simulink model "D_20210914_Modell_Inbetriebnahme_BreakOutBox_Jetson"  (R2021a)
(part 4 of 7)

  CAN Unpack52 : canmsglib/CAN Unpack  CANdbFile=eWolf_SensorCAN.dbc  MsgList=Radar_RawTarget_Data_051  MsgName=Radar_RawTarget_Data_051  MsgIDType=Standard (11-bit identifier)  MsgIdentifier=1075  MsgLength=8  SignalInfo={ 'AZ_Winkel', '22', '10', 'LE', 'unsigned', 'Multiplexed', '0', '0.16', '-81.76', '-81.76', '81.92'; 'EL_Angle', '37', '10', 'LE', 'unsigned', 'Multiplexed', '1', '0.04', '-20.44', '-20.44', '20.48'; 'Internal_used', '14', '8', 'LE', 'unsigned', 'Multiplexed', '0', '1', '0', '-Inf', 'Inf'; 'Internal_used2', '32', '7', 'LE', 'unsigned', 'Multiplexed', '0', '1', '0', '-Inf', 'Inf'; 'Internal_used3', '51', '7', 'LE', 'unsigned', 'Multiplexed', '0', '1', '0', '-Inf', 'Inf'; 'Internal_used4', '58', '6', 'LE', 'unsigned', 'Multiplexed', '0', '1', '0', '-Inf', 'Inf'; 'Internal_used5', '9', '8', 'LE', 'unsigned', 'Multiplexed', '1', '1', '0', '-Inf', 'Inf'; 'Internal_used6', '17', '8', 'LE', 'unsigned', 'Multiplexed', '1', '1', '0', '-Inf', 'Inf'; 'Internal_used7', '25', '7', 'LE', 'unsigned', 'Multiplexed', '1', '1', '0', '-Inf', 'Inf'; 'Mode_Signal', '0', '1', 'LE', 'unsigned', 'Multiplexor', '0', '1', '0', '0', '1'; 'RCS', '1', '7', 'LE', 'unsigned', 'Multiplexed', '1', '0.2', '-15', '-15', '36'; 'Range1', '1', '13', 'LE', 'unsigned', 'Multiplexed', '0', '0.04', '0', '0', '327.64'; 'Reserve_3', '32', '5', 'LE', 'unsigned', 'Multiplexed', '1', '1', '0', '-Inf', 'Inf'; 'Reserve_4', '47', '16', 'LE', 'unsigned', 'Multiplexed', '1', '1', '0', '-Inf', 'Inf'; 'Speed_Radial', '39', '12', 'LE', 'unsigned', 'Multiplexed', '0', '0.04', '-119.68', '-44.12', '119.68' }  IDPort=on  TimestampPort=on  ErrorPort=off  RemotePort=off  LengthPort=off  StatusPort=off  ApplyMinMax=off
      settings: SourceProductBaseCode=ME,XP,VN  DataFormat=CANdb specified signals
  CAN Unpack53 : canmsglib/CAN Unpack  CANdbFile=eWolf_SensorCAN.dbc  MsgList=Radar_RawTarget_Data_052  MsgName=Radar_RawTarget_Data_052  MsgIDType=Standard (11-bit identifier)  MsgIdentifier=1076  MsgLength=8  SignalInfo={ 'AZ_Winkel', '22', '10', 'LE', 'unsigned', 'Multiplexed', '0', '0.16', '-81.76', '-81.76', '81.92'; 'EL_Angle', '37', '10', 'LE', 'unsigned', 'Multiplexed', '1', '0.04', '-20.44', '-20.44', '20.48'; 'Internal_used', '14', '8', 'LE', 'unsigned', 'Multiplexed', '0', '1', '0', '-Inf', 'Inf'; 'Internal_used2', '32', '7', 'LE', 'unsigned', 'Multiplexed', '0', '1', '0', '-Inf', 'Inf'; 'Internal_used3', '51', '7', 'LE', 'unsigned', 'Multiplexed', '0', '1', '0', '-Inf', 'Inf'; 'Internal_used4', '58', '6', 'LE', 'unsigned', 'Multiplexed', '0', '1', '0', '-Inf', 'Inf'; 'Internal_used5', '9', '8', 'LE', 'unsigned', 'Multiplexed', '1', '1', '0', '-Inf', 'Inf'; 'Internal_used6', '17', '8', 'LE', 'unsigned', 'Multiplexed', '1', '1', '0', '-Inf', 'Inf'; 'Internal_used7', '25', '7', 'LE', 'unsigned', 'Multiplexed', '1', '1', '0', '-Inf', 'Inf'; 'Mode_Signal', '0', '1', 'LE', 'unsigned', 'Multiplexor', '0', '1', '0', '0', '1'; 'RCS', '1', '7', 'LE', 'unsigned', 'Multiplexed', '1', '0.2', '-15', '-15', '36'; 'Range1', '1', '13', 'LE', 'unsigned', 'Multiplexed', '0', '0.04', '0', '0', '327.64'; 'Reserve_3', '32', '5', 'LE', 'unsigned', 'Multiplexed', '1', '1', '0', '-Inf', 'Inf'; 'Reserve_4', '47', '16', 'LE', 'unsigned', 'Multiplexed', '1', '1', '0', '-Inf', 'Inf'; 'Speed_Radial', '39', '12', 'LE', 'unsigned', 'Multiplexed', '0', '0.04', '-119.68', '-44.12', '119.68' }  IDPort=on  TimestampPort=on  ErrorPort=off  RemotePort=off  LengthPort=off  StatusPort=off  ApplyMinMax=off
      settings: SourceProductBaseCode=ME,XP,VN  DataFormat=CANdb specified signals
  CAN Unpack54 : canmsglib/CAN Unpack  CANdbFile=eWolf_SensorCAN.dbc  MsgList=Radar_RawTarget_Data_053  MsgName=Radar_RawTarget_Data_053  MsgIDType=Standard (11-bit identifier)  MsgIdentifier=1077  MsgLength=8  SignalInfo={ 'AZ_Winkel', '22', '10', 'LE', 'unsigned', 'Multiplexed', '0', '0.16', '-81.76', '-81.76', '81.92'; 'EL_Angle', '37', '10', 'LE', 'unsigned', 'Multiplexed', '1', '0.04', '-20.44', '-20.44', '20.48'; 'Internal_used', '14', '8', 'LE', 'unsigned', 'Multiplexed', '0', '1', '0', '-Inf', 'Inf'; 'Internal_used2', '32', '7', 'LE', 'unsigned', 'Multiplexed', '0', '1', '0', '-Inf', 'Inf'; 'Internal_used3', '51', '7', 'LE', 'unsigned', 'Multiplexed', '0', '1', '0', '-Inf', 'Inf'; 'Internal_used4', '58', '6', 'LE', 'unsigned', 'Multiplexed', '0', '1', '0', '-Inf', 'Inf'; 'Internal_used5', '9', '8', 'LE', 'unsigned', 'Multiplexed', '1', '1', '0', '-Inf', 'Inf'; 'Internal_used6', '17', '8', 'LE', 'unsigned', 'Multiplexed', '1', '1', '0', '-Inf', 'Inf'; 'Internal_used7', '25', '7', 'LE', 'unsigned', 'Multiplexed', '1', '1', '0', '-Inf', 'Inf'; 'Mode_Signal', '0', '1', 'LE', 'unsigned', 'Multiplexor', '0', '1', '0', '0', '1'; 'RCS', '1', '7', 'LE', 'unsigned', 'Multiplexed', '1', '0.2', '-15', '-15', '36'; 'Range1', '1', '13', 'LE', 'unsigned', 'Multiplexed', '0', '0.04', '0', '0', '327.64'; 'Reserve_3', '32', '5', 'LE', 'unsigned', 'Multiplexed', '1', '1', '0', '-Inf', 'Inf'; 'Reserve_4', '47', '16', 'LE', 'unsigned', 'Multiplexed', '1', '1', '0', '-Inf', 'Inf'; 'Speed_Radial', '39', '12', 'LE', 'unsigned', 'Multiplexed', '0', '0.04', '-119.68', '-44.12', '119.68' }  IDPort=on  TimestampPort=on  ErrorPort=off  RemotePort=off  LengthPort=off  StatusPort=off  ApplyMinMax=off
      settings: SourceProductBaseCode=ME,XP,VN  DataFormat=CANdb specified signals
  CAN Unpack55 : canmsglib/CAN Unpack  CANdbFile=eWolf_SensorCAN.dbc  MsgList=Radar_RawTarget_Data_054  MsgName=Radar_RawTarget_Data_054  MsgIDType=Standard (11-bit identifier)  MsgIdentifier=1078  MsgLength=8  SignalInfo={ 'AZ_Winkel', '22', '10', 'LE', 'unsigned', 'Multiplexed', '0', '0.16', '-81.76', '-81.76', '81.92'; 'EL_Angle', '37', '10', 'LE', 'unsigned', 'Multiplexed', '1', '0.04', '-20.44', '-20.44', '20.48'; 'Internal_used', '14', '8', 'LE', 'unsigned', 'Multiplexed', '0', '1', '0', '-Inf', 'Inf'; 'Internal_used2', '32', '7', 'LE', 'unsigned', 'Multiplexed', '0', '1', '0', '-Inf', 'Inf'; 'Internal_used3', '51', '7', 'LE', 'unsigned', 'Multiplexed', '0', '1', '0', '-Inf', 'Inf'; 'Internal_used4', '58', '6', 'LE', 'unsigned', 'Multiplexed', '0', '1', '0', '-Inf', 'Inf'; 'Internal_used5', '9', '8', 'LE', 'unsigned', 'Multiplexed', '1', '1', '0', '-Inf', 'Inf'; 'Internal_used6', '17', '8', 'LE', 'unsigned', 'Multiplexed', '1', '1', '0', '-Inf', 'Inf'; 'Internal_used7', '25', '7', 'LE', 'unsigned', 'Multiplexed', '1', '1', '0', '-Inf', 'Inf'; 'Mode_Signal', '0', '1', 'LE', 'unsigned', 'Multiplexor', '0', '1', '0', '0', '1'; 'RCS', '1', '7', 'LE', 'unsigned', 'Multiplexed', '1', '0.2', '-15', '-15', '36'; 'Range1', '1', '13', 'LE', 'unsigned', 'Multiplexed', '0', '0.04', '0', '0', '327.64'; 'Reserve_3', '32', '5', 'LE', 'unsigned', 'Multiplexed', '1', '1', '0', '-Inf', 'Inf'; 'Reserve_4', '47', '16', 'LE', 'unsigned', 'Multiplexed', '1', '1', '0', '-Inf', 'Inf'; 'Speed_Radial', '39', '12', 'LE', 'unsigned', 'Multiplexed', '0', '0.04', '-119.68', '-44.12', '119.68' }  IDPort=on  TimestampPort=on  ErrorPort=off  RemotePort=off  LengthPort=off  StatusPort=off  ApplyMinMax=off
      settings: SourceProductBaseCode=ME,XP,VN  DataFormat=CANdb specified signals
  CAN Unpack56 : canmsglib/CAN Unpack  CANdbFile=eWolf_SensorCAN.dbc  MsgList=Radar_RawTarget_Data_055  MsgName=Radar_RawTarget_Data_055  MsgIDType=Standard (11-bit identifier)  MsgIdentifier=1079  MsgLength=8  SignalInfo={ 'AZ_Winkel', '22', '10', 'LE', 'unsigned', 'Multiplexed', '0', '0.16', '-81.76', '-81.76', '81.92'; 'EL_Angle', '37', '10', 'LE', 'unsigned', 'Multiplexed', '1', '0.04', '-20.44', '-20.44', '20.48'; 'Internal_used', '14', '8', 'LE', 'unsigned', 'Multiplexed', '0', '1', '0', '-Inf', 'Inf'; 'Internal_used2', '32', '7', 'LE', 'unsigned', 'Multiplexed', '0', '1', '0', '-Inf', 'Inf'; 'Internal_used3', '51', '7', 'LE', 'unsigned', 'Multiplexed', '0', '1', '0', '-Inf', 'Inf'; 'Internal_used4', '58', '6', 'LE', 'unsigned', 'Multiplexed', '0', '1', '0', '-Inf', 'Inf'; 'Internal_used5', '9', '8', 'LE', 'unsigned', 'Multiplexed', '1', '1', '0', '-Inf', 'Inf'; 'Internal_used6', '17', '8', 'LE', 'unsigned', 'Multiplexed', '1', '1', '0', '-Inf', 'Inf'; 'Internal_used7', '25', '7', 'LE', 'unsigned', 'Multiplexed', '1', '1', '0', '-Inf', 'Inf'; 'Mode_Signal', '0', '1', 'LE', 'unsigned', 'Multiplexor', '0', '1', '0', '0', '1'; 'RCS', '1', '7', 'LE', 'unsigned', 'Multiplexed', '1', '0.2', '-15', '-15', '36'; 'Range1', '1', '13', 'LE', 'unsigned', 'Multiplexed', '0', '0.04', '0', '0', '327.64'; 'Reserve_3', '32', '5', 'LE', 'unsigned', 'Multiplexed', '1', '1', '0', '-Inf', 'Inf'; 'Reserve_4', '47', '16', 'LE', 'unsigned', 'Multiplexed', '1', '1', '0', '-Inf', 'Inf'; 'Speed_Radial', '39', '12', 'LE', 'unsigned', 'Multiplexed', '0', '0.04', '-119.68', '-44.12', '119.68' }  IDPort=on  TimestampPort=on  ErrorPort=off  RemotePort=off  LengthPort=off  StatusPort=off  ApplyMinMax=off
      settings: SourceProductBaseCode=ME,XP,VN  DataFormat=CANdb specified signals
  CAN Unpack57 : canmsglib/CAN Unpack  CANdbFile=eWolf_SensorCAN.dbc  MsgList=Radar_RawTarget_Data_056  MsgName=Radar_RawTarget_Data_056  MsgIDType=Standard (11-bit identifier)  MsgIdentifier=1080  MsgLength=8  SignalInfo={ 'AZ_Winkel', '22', '10', 'LE', 'unsigned', 'Multiplexed', '0', '0.16', '-81.76', '-81.76', '81.92'; 'EL_Angle', '37', '10', 'LE', 'unsigned', 'Multiplexed', '1', '0.04', '-20.44', '-20.44', '20.48'; 'Internal_used', '14', '8', 'LE', 'unsigned', 'Multiplexed', '0', '1', '0', '-Inf', 'Inf'; 'Internal_used2', '32', '7', 'LE', 'unsigned', 'Multiplexed', '0', '1', '0', '-Inf', 'Inf'; 'Internal_used3', '51', '7', 'LE', 'unsigned', 'Multiplexed', '0', '1', '0', '-Inf', 'Inf'; 'Internal_used4', '58', '6', 'LE', 'unsigned', 'Multiplexed', '0', '1', '0', '-Inf', 'Inf'; 'Internal_used5', '9', '8', 'LE', 'unsigned', 'Multiplexed', '1', '1', '0', '-Inf', 'Inf'; 'Internal_used6', '17', '8', 'LE', 'unsigned', 'Multiplexed', '1', '1', '0', '-Inf', 'Inf'; 'Internal_used7', '25', '7', 'LE', 'unsigned', 'Multiplexed', '1', '1', '0', '-Inf', 'Inf'; 'Mode_Signal', '0', '1', 'LE', 'unsigned', 'Multiplexor', '0', '1', '0', '0', '1'; 'RCS', '1', '7', 'LE', 'unsigned', 'Multiplexed', '1', '0.2', '-15', '-15', '36'; 'Range1', '1', '13', 'LE', 'unsigned', 'Multiplexed', '0', '0.04', '0', '0', '327.64'; 'Reserve_3', '32', '5', 'LE', 'unsigned', 'Multiplexed', '1', '1', '0', '-Inf', 'Inf'; 'Reserve_4', '47', '16', 'LE', 'unsigned', 'Multiplexed', '1', '1', '0', '-Inf', 'Inf'; 'Speed_Radial', '39', '12', 'LE', 'unsigned', 'Multiplexed', '0', '0.04', '-119.68', '-44.12', '119.68' }  IDPort=on  TimestampPort=on  ErrorPort=off  RemotePort=off  LengthPort=off  StatusPort=off  ApplyMinMax=off
      settings: SourceProductBaseCode=ME,XP,VN  DataFormat=CANdb specified signals
  CAN Unpack58 : canmsglib/CAN Unpack  CANdbFile=eWolf_SensorCAN.dbc  MsgList=Radar_RawTarget_Data_057  MsgName=Radar_RawTarget_Data_057  MsgIDType=Standard (11-bit identifier)  MsgIdentifier=1081  MsgLength=8  SignalInfo={ 'AZ_Winkel', '22', '10', 'LE', 'unsigned', 'Multiplexed', '0', '0.16', '-81.76', '-81.76', '81.92'; 'EL_Angle', '37', '10', 'LE', 'unsigned', 'Multiplexed', '1', '0.04', '-20.44', '-20.44', '20.48'; 'Internal_used', '14', '8', 'LE', 'unsigned', 'Multiplexed', '0', '1', '0', '-Inf', 'Inf'; 'Internal_used2', '32', '7', 'LE', 'unsigned', 'Multiplexed', '0', '1', '0', '-Inf', 'Inf'; 'Internal_used3', '51', '7', 'LE', 'unsigned', 'Multiplexed', '0', '1', '0', '-Inf', 'Inf'; 'Internal_used4', '58', '6', 'LE', 'unsigned', 'Multiplexed', '0', '1', '0', '-Inf', 'Inf'; 'Internal_used5', '9', '8', 'LE', 'unsigned', 'Multiplexed', '1', '1', '0', '-Inf', 'Inf'; 'Internal_used6', '17', '8', 'LE', 'unsigned', 'Multiplexed', '1', '1', '0', '-Inf', 'Inf'; 'Internal_used7', '25', '7', 'LE', 'unsigned', 'Multiplexed', '1', '1', '0', '-Inf', 'Inf'; 'Mode_Signal', '0', '1', 'LE', 'unsigned', 'Multiplexor', '0', '1', '0', '0', '1'; 'RCS', '1', '7', 'LE', 'unsigned', 'Multiplexed', '1', '0.2', '-15', '-15', '36'; 'Range1', '1', '13', 'LE', 'unsigned', 'Multiplexed', '0', '0.04', '0', '0', '327.64'; 'Reserve_3', '32', '5', 'LE', 'unsigned', 'Multiplexed', '1', '1', '0', '-Inf', 'Inf'; 'Reserve_4', '47', '16', 'LE', 'unsigned', 'Multiplexed', '1', '1', '0', '-Inf', 'Inf'; 'Speed_Radial', '39', '12', 'LE', 'unsigned', 'Multiplexed', '0', '0.04', '-119.68', '-44.12', '119.68' }  IDPort=on  TimestampPort=on  ErrorPort=off  RemotePort=off  LengthPort=off  StatusPort=off  ApplyMinMax=off
      settings: SourceProductBaseCode=ME,XP,VN  DataFormat=CANdb specified signals
  CAN Unpack59 : canmsglib/CAN Unpack  CANdbFile=eWolf_SensorCAN.dbc  MsgList=Radar_RawTarget_Data_058  MsgName=Radar_RawTarget_Data_058  MsgIDType=Standard (11-bit identifier)  MsgIdentifier=1082  MsgLength=8  SignalInfo={ 'AZ_Winkel', '22', '10', 'LE', 'unsigned', 'Multiplexed', '0', '0.16', '-81.76', '-81.76', '81.92'; 'EL_Angle', '37', '10', 'LE', 'unsigned', 'Multiplexed', '1', '0.04', '-20.44', '-20.44', '20.48'; 'Internal_used', '14', '8', 'LE', 'unsigned', 'Multiplexed', '0', '1', '0', '-Inf', 'Inf'; 'Internal_used2', '32', '7', 'LE', 'unsigned', 'Multiplexed', '0', '1', '0', '-Inf', 'Inf'; 'Internal_used3', '51', '7', 'LE', 'unsigned', 'Multiplexed', '0', '1', '0', '-Inf', 'Inf'; 'Internal_used4', '58', '6', 'LE', 'unsigned', 'Multiplexed', '0', '1', '0', '-Inf', 'Inf'; 'Internal_used5', '9', '8', 'LE', 'unsigned', 'Multiplexed', '1', '1', '0', '-Inf', 'Inf'; 'Internal_used6', '17', '8', 'LE', 'unsigned', 'Multiplexed', '1', '1', '0', '-Inf', 'Inf'; 'Internal_used7', '25', '7', 'LE', 'unsigned', 'Multiplexed', '1', '1', '0', '-Inf', 'Inf'; 'Mode_Signal', '0', '1', 'LE', 'unsigned', 'Multiplexor', '0', '1', '0', '0', '1'; 'RCS', '1', '7', 'LE', 'unsigned', 'Multiplexed', '1', '0.2', '-15', '-15', '36'; 'Range1', '1', '13', 'LE', 'unsigned', 'Multiplexed', '0', '0.04', '0', '0', '327.64'; 'Reserve_3', '32', '5', 'LE', 'unsigned', 'Multiplexed', '1', '1', '0', '-Inf', 'Inf'; 'Reserve_4', '47', '16', 'LE', 'unsigned', 'Multiplexed', '1', '1', '0', '-Inf', 'Inf'; 'Speed_Radial', '39', '12', 'LE', 'unsigned', 'Multiplexed', '0', '0.04', '-119.68', '-44.12', '119.68' }  IDPort=on  TimestampPort=on  ErrorPort=off  RemotePort=off  LengthPort=off  StatusPort=off  ApplyMinMax=off
      settings: SourceProductBaseCode=ME,XP,VN  DataFormat=CANdb specified signals
  CAN Unpack6 : canmsglib/CAN Unpack  CANdbFile=eWolf_SensorCAN.dbc  MsgList=Radar_RawTarget_Data_005  MsgName=Radar_RawTarget_Data_005  MsgIDType=Standard (11-bit identifier)  MsgIdentifier=1029  MsgLength=8  SignalInfo={ 'AZ_Winkel', '22', '10', 'LE', 'unsigned', 'Multiplexed', '0', '0.16', '-81.76', '-81.76', '81.92'; 'EL_Angle', '37', '10', 'LE', 'unsigned', 'Multiplexed', '1', '0.04', '-20.44', '-20.44', '20.48'; 'Internal_used', '14', '8', 'LE', 'unsigned', 'Multiplexed', '0', '1', '0', '-Inf', 'Inf'; 'Internal_used2', '32', '7', 'LE', 'unsigned', 'Multiplexed', '0', '1', '0', '-Inf', 'Inf'; 'Internal_used3', '51', '7', 'LE', 'unsigned', 'Multiplexed', '0', '1', '0', '-Inf', 'Inf'; 'Internal_used4', '58', '6', 'LE', 'unsigned', 'Multiplexed', '0', '1', '0', '-Inf', 'Inf'; 'Internal_used5', '9', '8', 'LE', 'unsigned', 'Multiplexed', '1', '1', '0', '-Inf', 'Inf'; 'Internal_used6', '17', '8', 'LE', 'unsigned', 'Multiplexed', '1', '1', '0', '-Inf', 'Inf'; 'Internal_used7', '25', '7', 'LE', 'unsigned', 'Multiplexed', '1', '1', '0', '-Inf', 'Inf'; 'Mode_Signal', '0', '1', 'LE', 'unsigned', 'Multiplexor', '0', '1', '0', '0', '1'; 'RCS', '1', '7', 'LE', 'unsigned', 'Multiplexed', '1', '0.2', '-15', '-15', '36'; 'Range1', '1', '13', 'LE', 'unsigned', 'Multiplexed', '0', '0.04', '0', '0', '327.64'; 'Reserve_3', '32', '5', 'LE', 'unsigned', 'Multiplexed', '1', '1', '0', '-Inf', 'Inf'; 'Reserve_4', '47', '16', 'LE', 'unsigned', 'Multiplexed', '1', '1', '0', '-Inf', 'Inf'; 'Speed_Radial', '39', '12', 'LE', 'unsigned', 'Multiplexed', '0', '0.04', '-119.68', '-44.12', '119.68' }  IDPort=on  TimestampPort=on  ErrorPort=off  RemotePort=off  LengthPort=off  StatusPort=off  ApplyMinMax=off
      settings: SourceProductBaseCode=ME,XP,VN  DataFormat=CANdb specified signals
  CAN Unpack60 : canmsglib/CAN Unpack  CANdbFile=eWolf_SensorCAN.dbc  MsgList=Radar_RawTarget_Data_059  MsgName=Radar_RawTarget_Data_059  MsgIDType=Standard (11-bit identifier)  MsgIdentifier=1083  MsgLength=8  SignalInfo={ 'AZ_Winkel', '22', '10', 'LE', 'unsigned', 'Multiplexed', '0', '0.16', '-81.76', '-81.76', '81.92'; 'EL_Angle', '37', '10', 'LE', 'unsigned', 'Multiplexed', '1', '0.04', '-20.44', '-20.44', '20.48'; 'Internal_used', '14', '8', 'LE', 'unsigned', 'Multiplexed', '0', '1', '0', '-Inf', 'Inf'; 'Internal_used2', '32', '7', 'LE', 'unsigned', 'Multiplexed', '0', '1', '0', '-Inf', 'Inf'; 'Internal_used3', '51', '7', 'LE', 'unsigned', 'Multiplexed', '0', '1', '0', '-Inf', 'Inf'; 'Internal_used4', '58', '6', 'LE', 'unsigned', 'Multiplexed', '0', '1', '0', '-Inf', 'Inf'; 'Internal_used5', '9', '8', 'LE', 'unsigned', 'Multiplexed', '1', '1', '0', '-Inf', 'Inf'; 'Internal_used6', '17', '8', 'LE', 'unsigned', 'Multiplexed', '1', '1', '0', '-Inf', 'Inf'; 'Internal_used7', '25', '7', 'LE', 'unsigned', 'Multiplexed', '1', '1', '0', '-Inf', 'Inf'; 'Mode_Signal', '0', '1', 'LE', 'unsigned', 'Multiplexor', '0', '1', '0', '0', '1'; 'RCS', '1', '7', 'LE', 'unsigned', 'Multiplexed', '1', '0.2', '-15', '-15', '36'; 'Range1', '1', '13', 'LE', 'unsigned', 'Multiplexed', '0', '0.04', '0', '0', '327.64'; 'Reserve_3', '32', '5', 'LE', 'unsigned', 'Multiplexed', '1', '1', '0', '-Inf', 'Inf'; 'Reserve_4', '47', '16', 'LE', 'unsigned', 'Multiplexed', '1', '1', '0', '-Inf', 'Inf'; 'Speed_Radial', '39', '12', 'LE', 'unsigned', 'Multiplexed', '0', '0.04', '-119.68', '-44.12', '119.68' }  IDPort=on  TimestampPort=on  ErrorPort=off  RemotePort=off  LengthPort=off  StatusPort=off  ApplyMinMax=off
      settings: SourceProductBaseCode=ME,XP,VN  DataFormat=CANdb specified signals
  CAN Unpack61 : canmsglib/CAN Unpack  CANdbFile=eWolf_SensorCAN.dbc  MsgList=Radar_RawTarget_Data_060  MsgName=Radar_RawTarget_Data_060  MsgIDType=Standard (11-bit identifier)  MsgIdentifier=1084  MsgLength=8  SignalInfo={ 'AZ_Winkel', '22', '10', 'LE', 'unsigned', 'Multiplexed', '0', '0.16', '-81.76', '-81.76', '81.92'; 'EL_Angle', '37', '10', 'LE', 'unsigned', 'Multiplexed', '1', '0.04', '-20.44', '-20.44', '20.48'; 'Internal_used', '14', '8', 'LE', 'unsigned', 'Multiplexed', '0', '1', '0', '-Inf', 'Inf'; 'Internal_used2', '32', '7', 'LE', 'unsigned', 'Multiplexed', '0', '1', '0', '-Inf', 'Inf'; 'Internal_used3', '51', '7', 'LE', 'unsigned', 'Multiplexed', '0', '1', '0', '-Inf', 'Inf'; 'Internal_used4', '58', '6', 'LE', 'unsigned', 'Multiplexed', '0', '1', '0', '-Inf', 'Inf'; 'Internal_used5', '9', '8', 'LE', 'unsigned', 'Multiplexed', '1', '1', '0', '-Inf', 'Inf'; 'Internal_used6', '17', '8', 'LE', 'unsigned', 'Multiplexed', '1', '1', '0', '-Inf', 'Inf'; 'Internal_used7', '25', '7', 'LE', 'unsigned', 'Multiplexed', '1', '1', '0', '-Inf', 'Inf'; 'Mode_Signal', '0', '1', 'LE', 'unsigned', 'Multiplexor', '0', '1', '0', '0', '1'; 'RCS', '1', '7', 'LE', 'unsigned', 'Multiplexed', '1', '0.2', '-15', '-15', '36'; 'Range1', '1', '13', 'LE', 'unsigned', 'Multiplexed', '0', '0.04', '0', '0', '327.64'; 'Reserve_3', '32', '5', 'LE', 'unsigned', 'Multiplexed', '1', '1', '0', '-Inf', 'Inf'; 'Reserve_4', '47', '16', 'LE', 'unsigned', 'Multiplexed', '1', '1', '0', '-Inf', 'Inf'; 'Speed_Radial', '39', '12', 'LE', 'unsigned', 'Multiplexed', '0', '0.04', '-119.68', '-44.12', '119.68' }  IDPort=on  TimestampPort=on  ErrorPort=off  RemotePort=off  LengthPort=off  StatusPort=off  ApplyMinMax=off
      settings: SourceProductBaseCode=ME,XP,VN  DataFormat=CANdb specified signals
  CAN Unpack62 : canmsglib/CAN Unpack  CANdbFile=eWolf_SensorCAN.dbc  MsgList=Radar_RawTarget_Data_061  MsgName=Radar_RawTarget_Data_061  MsgIDType=Standard (11-bit identifier)  MsgIdentifier=1085  MsgLength=8  SignalInfo={ 'AZ_Winkel', '22', '10', 'LE', 'unsigned', 'Multiplexed', '0', '0.16', '-81.76', '-81.76', '81.92'; 'EL_Angle', '37', '10', 'LE', 'unsigned', 'Multiplexed', '1', '0.04', '-20.44', '-20.44', '20.48'; 'Internal_used', '14', '8', 'LE', 'unsigned', 'Multiplexed', '0', '1', '0', '-Inf', 'Inf'; 'Internal_used2', '32', '7', 'LE', 'unsigned', 'Multiplexed', '0', '1', '0', '-Inf', 'Inf'; 'Internal_used3', '51', '7', 'LE', 'unsigned', 'Multiplexed', '0', '1', '0', '-Inf', 'Inf'; 'Internal_used4', '58', '6', 'LE', 'unsigned', 'Multiplexed', '0', '1', '0', '-Inf', 'Inf'; 'Internal_used5', '9', '8', 'LE', 'unsigned', 'Multiplexed', '1', '1', '0', '-Inf', 'Inf'; 'Internal_used6', '17', '8', 'LE', 'unsigned', 'Multiplexed', '1', '1', '0', '-Inf', 'Inf'; 'Internal_used7', '25', '7', 'LE', 'unsigned', 'Multiplexed', '1', '1', '0', '-Inf', 'Inf'; 'Mode_Signal', '0', '1', 'LE', 'unsigned', 'Multiplexor', '0', '1', '0', '0', '1'; 'RCS', '1', '7', 'LE', 'unsigned', 'Multiplexed', '1', '0.2', '-15', '-15', '36'; 'Range1', '1', '13', 'LE', 'unsigned', 'Multiplexed', '0', '0.04', '0', '0', '327.64'; 'Reserve_3', '32', '5', 'LE', 'unsigned', 'Multiplexed', '1', '1', '0', '-Inf', 'Inf'; 'Reserve_4', '47', '16', 'LE', 'unsigned', 'Multiplexed', '1', '1', '0', '-Inf', 'Inf'; 'Speed_Radial', '39', '12', 'LE', 'unsigned', 'Multiplexed', '0', '0.04', '-119.68', '-44.12', '119.68' }  IDPort=on  TimestampPort=on  ErrorPort=off  RemotePort=off  LengthPort=off  StatusPort=off  ApplyMinMax=off
      settings: SourceProductBaseCode=ME,XP,VN  DataFormat=CANdb specified signals
  CAN Unpack63 : canmsglib/CAN Unpack  CANdbFile=eWolf_SensorCAN.dbc  MsgList=Radar_RawTarget_Data_062  MsgName=Radar_RawTarget_Data_062  MsgIDType=Standard (11-bit identifier)  MsgIdentifier=1086  MsgLength=8  SignalInfo={ 'AZ_Winkel', '22', '10', 'LE', 'unsigned', 'Multiplexed', '0', '0.16', '-81.76', '-81.76', '81.92'; 'EL_Angle', '37', '10', 'LE', 'unsigned', 'Multiplexed', '1', '0.04', '-20.44', '-20.44', '20.48'; 'Internal_used', '14', '8', 'LE', 'unsigned', 'Multiplexed', '0', '1', '0', '-Inf', 'Inf'; 'Internal_used2', '32', '7', 'LE', 'unsigned', 'Multiplexed', '0', '1', '0', '-Inf', 'Inf'; 'Internal_used3', '51', '7', 'LE', 'unsigned', 'Multiplexed', '0', '1', '0', '-Inf', 'Inf'; 'Internal_used4', '58', '6', 'LE', 'unsigned', 'Multiplexed', '0', '1', '0', '-Inf', 'Inf'; 'Internal_used5', '9', '8', 'LE', 'unsigned', 'Multiplexed', '1', '1', '0', '-Inf', 'Inf'; 'Internal_used6', '17', '8', 'LE', 'unsigned', 'Multiplexed', '1', '1', '0', '-Inf', 'Inf'; 'Internal_used7', '25', '7', 'LE', 'unsigned', 'Multiplexed', '1', '1', '0', '-Inf', 'Inf'; 'Mode_Signal', '0', '1', 'LE', 'unsigned', 'Multiplexor', '0', '1', '0', '0', '1'; 'RCS', '1', '7', 'LE', 'unsigned', 'Multiplexed', '1', '0.2', '-15', '-15', '36'; 'Range1', '1', '13', 'LE', 'unsigned', 'Multiplexed', '0', '0.04', '0', '0', '327.64'; 'Reserve_3', '32', '5', 'LE', 'unsigned', 'Multiplexed', '1', '1', '0', '-Inf', 'Inf'; 'Reserve_4', '47', '16', 'LE', 'unsigned', 'Multiplexed', '1', '1', '0', '-Inf', 'Inf'; 'Speed_Radial', '39', '12', 'LE', 'unsigned', 'Multiplexed', '0', '0.04', '-119.68', '-44.12', '119.68' }  IDPort=on  TimestampPort=on  ErrorPort=off  RemotePort=off  LengthPort=off  StatusPort=off  ApplyMinMax=off
      settings: SourceProductBaseCode=ME,XP,VN  DataFormat=CANdb specified signals
  CAN Unpack64 : canmsglib/CAN Unpack  CANdbFile=eWolf_SensorCAN.dbc  MsgList=Radar_RawTarget_Data_063  MsgName=Radar_RawTarget_Data_063  MsgIDType=Standard (11-bit identifier)  MsgIdentifier=1087  MsgLength=8  SignalInfo={ 'AZ_Winkel', '22', '10', 'LE', 'unsigned', 'Multiplexed', '0', '0.16', '-81.76', '-81.76', '81.92'; 'EL_Angle', '37', '10', 'LE', 'unsigned', 'Multiplexed', '1', '0.04', '-20.44', '-20.44', '20.48'; 'Internal_used', '14', '8', 'LE', 'unsigned', 'Multiplexed', '0', '1', '0', '-Inf', 'Inf'; 'Internal_used2', '32', '7', 'LE', 'unsigned', 'Multiplexed', '0', '1', '0', '-Inf', 'Inf'; 'Internal_used3', '51', '7', 'LE', 'unsigned', 'Multiplexed', '0', '1', '0', '-Inf', 'Inf'; 'Internal_used4', '58', '6', 'LE', 'unsigned', 'Multiplexed', '0', '1', '0', '-Inf', 'Inf'; 'Internal_used5', '9', '8', 'LE', 'unsigned', 'Multiplexed', '1', '1', '0', '-Inf', 'Inf'; 'Internal_used6', '17', '8', 'LE', 'unsigned', 'Multiplexed', '1', '1', '0', '-Inf', 'Inf'; 'Internal_used7', '25', '7', 'LE', 'unsigned', 'Multiplexed', '1', '1', '0', '-Inf', 'Inf'; 'Mode_Signal', '0', '1', 'LE', 'unsigned', 'Multiplexor', '0', '1', '0', '0', '1'; 'RCS', '1', '7', 'LE', 'unsigned', 'Multiplexed', '1', '0.2', '-15', '-15', '36'; 'Range1', '1', '13', 'LE', 'unsigned', 'Multiplexed', '0', '0.04', '0', '0', '327.64'; 'Reserve_3', '32', '5', 'LE', 'unsigned', 'Multiplexed', '1', '1', '0', '-Inf', 'Inf'; 'Reserve_4', '47', '16', 'LE', 'unsigned', 'Multiplexed', '1', '1', '0', '-Inf', 'Inf'; 'Speed_Radial', '39', '12', 'LE', 'unsigned', 'Multiplexed', '0', '0.04', '-119.68', '-44.12', '119.68' }  IDPort=on  TimestampPort=on  ErrorPort=off  RemotePort=off  LengthPort=off  StatusPort=off  ApplyMinMax=off
      settings: SourceProductBaseCode=ME,XP,VN  DataFormat=CANdb specified signals
  CAN Unpack65 : canmsglib/CAN Unpack  CANdbFile=eWolf_SensorCAN.dbc  MsgList=Radar_RawTarget_Data_064  MsgName=Radar_RawTarget_Data_064  MsgIDType=Standard (11-bit identifier)  MsgIdentifier=1088  MsgLength=8  SignalInfo={ 'AZ_Winkel', '22', '10', 'LE', 'unsigned', 'Multiplexed', '0', '0.16', '-81.76', '-81.76', '81.92'; 'EL_Angle', '37', '10', 'LE', 'unsigned', 'Multiplexed', '1', '0.04', '-20.44', '-20.44', '20.48'; 'Internal_used', '14', '8', 'LE', 'unsigned', 'Multiplexed', '0', '1', '0', '-Inf', 'Inf'; 'Internal_used2', '32', '7', 'LE', 'unsigned', 'Multiplexed', '0', '1', '0', '-Inf', 'Inf'; 'Internal_used3', '51', '7', 'LE', 'unsigned', 'Multiplexed', '0', '1', '0', '-Inf', 'Inf'; 'Internal_used4', '58', '6', 'LE', 'unsigned', 'Multiplexed', '0', '1', '0', '-Inf', 'Inf'; 'Internal_used5', '9', '8', 'LE', 'unsigned', 'Multiplexed', '1', '1', '0', '-Inf', 'Inf'; 'Internal_used6', '17', '8', 'LE', 'unsigned', 'Multiplexed', '1', '1', '0', '-Inf', 'Inf'; 'Internal_used7', '25', '7', 'LE', 'unsigned', 'Multiplexed', '1', '1', '0', '-Inf', 'Inf'; 'Mode_Signal', '0', '1', 'LE', 'unsigned', 'Multiplexor', '0', '1', '0', '0', '1'; 'RCS', '1', '7', 'LE', 'unsigned', 'Multiplexed', '1', '0.2', '-15', '-15', '36'; 'Range1', '1', '13', 'LE', 'unsigned', 'Multiplexed', '0', '0.04', '0', '0', '327.64'; 'Reserve_3', '32', '5', 'LE', 'unsigned', 'Multiplexed', '1', '1', '0', '-Inf', 'Inf'; 'Reserve_4', '47', '16', 'LE', 'unsigned', 'Multiplexed', '1', '1', '0', '-Inf', 'Inf'; 'Speed_Radial', '39', '12', 'LE', 'unsigned', 'Multiplexed', '0', '0.04', '-119.68', '-44.12', '119.68' }  IDPort=on  TimestampPort=on  ErrorPort=off  RemotePort=off  LengthPort=off  StatusPort=off  ApplyMinMax=off
      settings: SourceProductBaseCode=ME,XP,VN  DataFormat=CANdb specified signals
  CAN Unpack66 : canmsglib/CAN Unpack  CANdbFile=eWolf_SensorCAN.dbc  MsgList=Radar_RawTarget_Data_065  MsgName=Radar_RawTarget_Data_065  MsgIDType=Standard (11-bit identifier)  MsgIdentifier=1089  MsgLength=8  SignalInfo={ 'AZ_Winkel', '22', '10', 'LE', 'unsigned', 'Multiplexed', '0', '0.16', '-81.76', '-81.76', '81.92'; 'EL_Angle', '37', '10', 'LE', 'unsigned', 'Multiplexed', '1', '0.04', '-20.44', '-20.44', '20.48'; 'Internal_used', '14', '8', 'LE', 'unsigned', 'Multiplexed', '0', '1', '0', '-Inf', 'Inf'; 'Internal_used2', '32', '7', 'LE', 'unsigned', 'Multiplexed', '0', '1', '0', '-Inf', 'Inf'; 'Internal_used3', '51', '7', 'LE', 'unsigned', 'Multiplexed', '0', '1', '0', '-Inf', 'Inf'; 'Internal_used4', '58', '6', 'LE', 'unsigned', 'Multiplexed', '0', '1', '0', '-Inf', 'Inf'; 'Internal_used5', '9', '8', 'LE', 'unsigned', 'Multiplexed', '1', '1', '0', '-Inf', 'Inf'; 'Internal_used6', '17', '8', 'LE', 'unsigned', 'Multiplexed', '1', '1', '0', '-Inf', 'Inf'; 'Internal_used7', '25', '7', 'LE', 'unsigned', 'Multiplexed', '1', '1', '0', '-Inf', 'Inf'; 'Mode_Signal', '0', '1', 'LE', 'unsigned', 'Multiplexor', '0', '1', '0', '0', '1'; 'RCS', '1', '7', 'LE', 'unsigned', 'Multiplexed', '1', '0.2', '-15', '-15', '36'; 'Range1', '1', '13', 'LE', 'unsigned', 'Multiplexed', '0', '0.04', '0', '0', '327.64'; 'Reserve_3', '32', '5', 'LE', 'unsigned', 'Multiplexed', '1', '1', '0', '-Inf', 'Inf'; 'Reserve_4', '47', '16', 'LE', 'unsigned', 'Multiplexed', '1', '1', '0', '-Inf', 'Inf'; 'Speed_Radial', '39', '12', 'LE', 'unsigned', 'Multiplexed', '0', '0.04', '-119.68', '-44.12', '119.68' }  IDPort=on  TimestampPort=on  ErrorPort=off  RemotePort=off  LengthPort=off  StatusPort=off  ApplyMinMax=off
      settings: SourceProductBaseCode=ME,XP,VN  DataFormat=CANdb specified signals
  CAN Unpack67 : canmsglib/CAN Unpack  CANdbFile=eWolf_SensorCAN.dbc  MsgList=Radar_RawTarget_Data_066  MsgName=Radar_RawTarget_Data_066  MsgIDType=Standard (11-bit identifier)  MsgIdentifier=1090  MsgLength=8  SignalInfo={ 'AZ_Winkel', '22', '10', 'LE', 'unsigned', 'Multiplexed', '0', '0.16', '-81.76', '-81.76', '81.92'; 'EL_Angle', '37', '10', 'LE', 'unsigned', 'Multiplexed', '1', '0.04', '-20.44', '-20.44', '20.48'; 'Internal_used', '14', '8', 'LE', 'unsigned', 'Multiplexed', '0', '1', '0', '-Inf', 'Inf'; 'Internal_used2', '32', '7', 'LE', 'unsigned', 'Multiplexed', '0', '1', '0', '-Inf', 'Inf'; 'Internal_used3', '51', '7', 'LE', 'unsigned', 'Multiplexed', '0', '1', '0', '-Inf', 'Inf'; 'Internal_used4', '58', '6', 'LE', 'unsigned', 'Multiplexed', '0', '1', '0', '-Inf', 'Inf'; 'Internal_used5', '9', '8', 'LE', 'unsigned', 'Multiplexed', '1', '1', '0', '-Inf', 'Inf'; 'Internal_used6', '17', '8', 'LE', 'unsigned', 'Multiplexed', '1', '1', '0', '-Inf', 'Inf'; 'Internal_used7', '25', '7', 'LE', 'unsigned', 'Multiplexed', '1', '1', '0', '-Inf', 'Inf'; 'Mode_Signal', '0', '1', 'LE', 'unsigned', 'Multiplexor', '0', '1', '0', '0', '1'; 'RCS', '1', '7', 'LE', 'unsigned', 'Multiplexed', '1', '0.2', '-15', '-15', '36'; 'Range1', '1', '13', 'LE', 'unsigned', 'Multiplexed', '0', '0.04', '0', '0', '327.64'; 'Reserve_3', '32', '5', 'LE', 'unsigned', 'Multiplexed', '1', '1', '0', '-Inf', 'Inf'; 'Reserve_4', '47', '16', 'LE', 'unsigned', 'Multiplexed', '1', '1', '0', '-Inf', 'Inf'; 'Speed_Radial', '39', '12', 'LE', 'unsigned', 'Multiplexed', '0', '0.04', '-119.68', '-44.12', '119.68' }  IDPort=on  TimestampPort=on  ErrorPort=off  RemotePort=off  LengthPort=off  StatusPort=off  ApplyMinMax=off
      settings: SourceProductBaseCode=ME,XP,VN  DataFormat=CANdb specified signals
  CAN Unpack68 : canmsglib/CAN Unpack  CANdbFile=eWolf_SensorCAN.dbc  MsgList=Radar_RawTarget_Data_067  MsgName=Radar_RawTarget_Data_067  MsgIDType=Standard (11-bit identifier)  MsgIdentifier=1091  MsgLength=8  SignalInfo={ 'AZ_Winkel', '22', '10', 'LE', 'unsigned', 'Multiplexed', '0', '0.16', '-81.76', '-81.76', '81.92'; 'EL_Angle', '37', '10', 'LE', 'unsigned', 'Multiplexed', '1', '0.04', '-20.44', '-20.44', '20.48'; 'Internal_used', '14', '8', 'LE', 'unsigned', 'Multiplexed', '0', '1', '0', '-Inf', 'Inf'; 'Internal_used2', '32', '7', 'LE', 'unsigned', 'Multiplexed', '0', '1', '0', '-Inf', 'Inf'; 'Internal_used3', '51', '7', 'LE', 'unsigned', 'Multiplexed', '0', '1', '0', '-Inf', 'Inf'; 'Internal_used4', '58', '6', 'LE', 'unsigned', 'Multiplexed', '0', '1', '0', '-Inf', 'Inf'; 'Internal_used5', '9', '8', 'LE', 'unsigned', 'Multiplexed', '1', '1', '0', '-Inf', 'Inf'; 'Internal_used6', '17', '8', 'LE', 'unsigned', 'Multiplexed', '1', '1', '0', '-Inf', 'Inf'; 'Internal_used7', '25', '7', 'LE', 'unsigned', 'Multiplexed', '1', '1', '0', '-Inf', 'Inf'; 'Mode_Signal', '0', '1', 'LE', 'unsigned', 'Multiplexor', '0', '1', '0', '0', '1'; 'RCS', '1', '7', 'LE', 'unsigned', 'Multiplexed', '1', '0.2', '-15', '-15', '36'; 'Range1', '1', '13', 'LE', 'unsigned', 'Multiplexed', '0', '0.04', '0', '0', '327.64'; 'Reserve_3', '32', '5', 'LE', 'unsigned', 'Multiplexed', '1', '1', '0', '-Inf', 'Inf'; 'Reserve_4', '47', '16', 'LE', 'unsigned', 'Multiplexed', '1', '1', '0', '-Inf', 'Inf'; 'Speed_Radial', '39', '12', 'LE', 'unsigned', 'Multiplexed', '0', '0.04', '-119.68', '-44.12', '119.68' }  IDPort=on  TimestampPort=on  ErrorPort=off  RemotePort=off  LengthPort=off  StatusPort=off  ApplyMinMax=off
      settings: SourceProductBaseCode=ME,XP,VN  DataFormat=CANdb specified signals
  CAN Unpack69 : canmsglib/CAN Unpack  CANdbFile=eWolf_SensorCAN.dbc  MsgList=Radar_RawTarget_Data_068  MsgName=Radar_RawTarget_Data_068  MsgIDType=Standard (11-bit identifier)  MsgIdentifier=1092  MsgLength=8  SignalInfo={ 'AZ_Winkel', '22', '10', 'LE', 'unsigned', 'Multiplexed', '0', '0.16', '-81.76', '-81.76', '81.92'; 'EL_Angle', '37', '10', 'LE', 'unsigned', 'Multiplexed', '1', '0.04', '-20.44', '-20.44', '20.48'; 'Internal_used', '14', '8', 'LE', 'unsigned', 'Multiplexed', '0', '1', '0', '-Inf', 'Inf'; 'Internal_used2', '32', '7', 'LE', 'unsigned', 'Multiplexed', '0', '1', '0', '-Inf', 'Inf'; 'Internal_used3', '51', '7', 'LE', 'unsigned', 'Multiplexed', '0', '1', '0', '-Inf', 'Inf'; 'Internal_used4', '58', '6', 'LE', 'unsigned', 'Multiplexed', '0', '1', '0', '-Inf', 'Inf'; 'Internal_used5', '9', '8', 'LE', 'unsigned', 'Multiplexed', '1', '1', '0', '-Inf', 'Inf'; 'Internal_used6', '17', '8', 'LE', 'unsigned', 'Multiplexed', '1', '1', '0', '-Inf', 'Inf'; 'Internal_used7', '25', '7', 'LE', 'unsigned', 'Multiplexed', '1', '1', '0', '-Inf', 'Inf'; 'Mode_Signal', '0', '1', 'LE', 'unsigned', 'Multiplexor', '0', '1', '0', '0', '1'; 'RCS', '1', '7', 'LE', 'unsigned', 'Multiplexed', '1', '0.2', '-15', '-15', '36'; 'Range1', '1', '13', 'LE', 'unsigned', 'Multiplexed', '0', '0.04', '0', '0', '327.64'; 'Reserve_3', '32', '5', 'LE', 'unsigned', 'Multiplexed', '1', '1', '0', '-Inf', 'Inf'; 'Reserve_4', '47', '16', 'LE', 'unsigned', 'Multiplexed', '1', '1', '0', '-Inf', 'Inf'; 'Speed_Radial', '39', '12', 'LE', 'unsigned', 'Multiplexed', '0', '0.04', '-119.68', '-44.12', '119.68' }  IDPort=on  TimestampPort=on  ErrorPort=off  RemotePort=off  LengthPort=off  StatusPort=off  ApplyMinMax=off
      settings: SourceProductBaseCode=ME,XP,VN  DataFormat=CANdb specified signals
  CAN Unpack7 : canmsglib/CAN Unpack  CANdbFile=eWolf_SensorCAN.dbc  MsgList=Radar_RawTarget_Data_006  MsgName=Radar_RawTarget_Data_006  MsgIDType=Standard (11-bit identifier)  MsgIdentifier=1030  MsgLength=8  SignalInfo={ 'AZ_Winkel', '22', '10', 'LE', 'unsigned', 'Multiplexed', '0', '0.16', '-81.76', '-81.76', '81.92'; 'EL_Angle', '37', '10', 'LE', 'unsigned', 'Multiplexed', '1', '0.04', '-20.44', '-20.44', '20.48'; 'Internal_used', '14', '8', 'LE', 'unsigned', 'Multiplexed', '0', '1', '0', '-Inf', 'Inf'; 'Internal_used2', '32', '7', 'LE', 'unsigned', 'Multiplexed', '0', '1', '0', '-Inf', 'Inf'; 'Internal_used3', '51', '7', 'LE', 'unsigned', 'Multiplexed', '0', '1', '0', '-Inf', 'Inf'; 'Internal_used4', '58', '6', 'LE', 'unsigned', 'Multiplexed', '0', '1', '0', '-Inf', 'Inf'; 'Internal_used5', '9', '8', 'LE', 'unsigned', 'Multiplexed', '1', '1', '0', '-Inf', 'Inf'; 'Internal_used6', '17', '8', 'LE', 'unsigned', 'Multiplexed', '1', '1', '0', '-Inf', 'Inf'; 'Internal_used7', '25', '7', 'LE', 'unsigned', 'Multiplexed', '1', '1', '0', '-Inf', 'Inf'; 'Mode_Signal', '0', '1', 'LE', 'unsigned', 'Multiplexor', '0', '1', '0', '0', '1'; 'RCS', '1', '7', 'LE', 'unsigned', 'Multiplexed', '1', '0.2', '-15', '-15', '36'; 'Range1', '1', '13', 'LE', 'unsigned', 'Multiplexed', '0', '0.04', '0', '0', '327.64'; 'Reserve_3', '32', '5', 'LE', 'unsigned', 'Multiplexed', '1', '1', '0', '-Inf', 'Inf'; 'Reserve_4', '47', '16', 'LE', 'unsigned', 'Multiplexed', '1', '1', '0', '-Inf', 'Inf'; 'Speed_Radial', '39', '12', 'LE', 'unsigned', 'Multiplexed', '0', '0.04', '-119.68', '-44.12', '119.68' }  IDPort=on  TimestampPort=on  ErrorPort=off  RemotePort=off  LengthPort=off  StatusPort=off  ApplyMinMax=off
      settings: SourceProductBaseCode=ME,XP,VN  DataFormat=CANdb specified signals
  CAN Unpack70 : canmsglib/CAN Unpack  CANdbFile=eWolf_SensorCAN.dbc  MsgList=Radar_RawTarget_Data_069  MsgName=Radar_RawTarget_Data_069  MsgIDType=Standard (11-bit identifier)  MsgIdentifier=1093  MsgLength=8  SignalInfo={ 'AZ_Winkel', '22', '10', 'LE', 'unsigned', 'Multiplexed', '0', '0.16', '-81.76', '-81.76', '81.92'; 'EL_Angle', '37', '10', 'LE', 'unsigned', 'Multiplexed', '1', '0.04', '-20.44', '-20.44', '20.48'; 'Internal_used', '14', '8', 'LE', 'unsigned', 'Multiplexed', '0', '1', '0', '-Inf', 'Inf'; 'Internal_used2', '32', '7', 'LE', 'unsigned', 'Multiplexed', '0', '1', '0', '-Inf', 'Inf'; 'Internal_used3', '51', '7', 'LE', 'unsigned', 'Multiplexed', '0', '1', '0', '-Inf', 'Inf'; 'Internal_used4', '58', '6', 'LE', 'unsigned', 'Multiplexed', '0', '1', '0', '-Inf', 'Inf'; 'Internal_used5', '9', '8', 'LE', 'unsigned', 'Multiplexed', '1', '1', '0', '-Inf', 'Inf'; 'Internal_used6', '17', '8', 'LE', 'unsigned', 'Multiplexed', '1', '1', '0', '-Inf', 'Inf'; 'Internal_used7', '25', '7', 'LE', 'unsigned', 'Multiplexed', '1', '1', '0', '-Inf', 'Inf'; 'Mode_Signal', '0', '1', 'LE', 'unsigned', 'Multiplexor', '0', '1', '0', '0', '1'; 'RCS', '1', '7', 'LE', 'unsigned', 'Multiplexed', '1', '0.2', '-15', '-15', '36'; 'Range1', '1', '13', 'LE', 'unsigned', 'Multiplexed', '0', '0.04', '0', '0', '327.64'; 'Reserve_3', '32', '5', 'LE', 'unsigned', 'Multiplexed', '1', '1', '0', '-Inf', 'Inf'; 'Reserve_4', '47', '16', 'LE', 'unsigned', 'Multiplexed', '1', '1', '0', '-Inf', 'Inf'; 'Speed_Radial', '39', '12', 'LE', 'unsigned', 'Multiplexed', '0', '0.04', '-119.68', '-44.12', '119.68' }  IDPort=on  TimestampPort=on  ErrorPort=off  RemotePort=off  LengthPort=off  StatusPort=off  ApplyMinMax=off
      settings: SourceProductBaseCode=ME,XP,VN  DataFormat=CANdb specified signals
  CAN Unpack71 : canmsglib/CAN Unpack  CANdbFile=eWolf_SensorCAN.dbc  MsgList=Radar_RawTarget_Data_070  MsgName=Radar_RawTarget_Data_070  MsgIDType=Standard (11-bit identifier)  MsgIdentifier=1094  MsgLength=8  SignalInfo={ 'AZ_Winkel', '22', '10', 'LE', 'unsigned', 'Multiplexed', '0', '0.16', '-81.76', '-81.76', '81.92'; 'EL_Angle', '37', '10', 'LE', 'unsigned', 'Multiplexed', '1', '0.04', '-20.44', '-20.44', '20.48'; 'Internal_used', '14', '8', 'LE', 'unsigned', 'Multiplexed', '0', '1', '0', '-Inf', 'Inf'; 'Internal_used2', '32', '7', 'LE', 'unsigned', 'Multiplexed', '0', '1', '0', '-Inf', 'Inf'; 'Internal_used3', '51', '7', 'LE', 'unsigned', 'Multiplexed', '0', '1', '0', '-Inf', 'Inf'; 'Internal_used4', '58', '6', 'LE', 'unsigned', 'Multiplexed', '0', '1', '0', '-Inf', 'Inf'; 'Internal_used5', '9', '8', 'LE', 'unsigned', 'Multiplexed', '1', '1', '0', '-Inf', 'Inf'; 'Internal_used6', '17', '8', 'LE', 'unsigned', 'Multiplexed', '1', '1', '0', '-Inf', 'Inf'; 'Internal_used7', '25', '7', 'LE', 'unsigned', 'Multiplexed', '1', '1', '0', '-Inf', 'Inf'; 'Mode_Signal', '0', '1', 'LE', 'unsigned', 'Multiplexor', '0', '1', '0', '0', '1'; 'RCS', '1', '7', 'LE', 'unsigned', 'Multiplexed', '1', '0.2', '-15', '-15', '36'; 'Range1', '1', '13', 'LE', 'unsigned', 'Multiplexed', '0', '0.04', '0', '0', '327.64'; 'Reserve_3', '32', '5', 'LE', 'unsigned', 'Multiplexed', '1', '1', '0', '-Inf', 'Inf'; 'Reserve_4', '47', '16', 'LE', 'unsigned', 'Multiplexed', '1', '1', '0', '-Inf', 'Inf'; 'Speed_Radial', '39', '12', 'LE', 'unsigned', 'Multiplexed', '0', '0.04', '-119.68', '-44.12', '119.68' }  IDPort=on  TimestampPort=on  ErrorPort=off  RemotePort=off  LengthPort=off  StatusPort=off  ApplyMinMax=off
      settings: SourceProductBaseCode=ME,XP,VN  DataFormat=CANdb specified signals
  CAN Unpack72 : canmsglib/CAN Unpack  CANdbFile=eWolf_SensorCAN.dbc  MsgList=Radar_RawTarget_Data_071  MsgName=Radar_RawTarget_Data_071  MsgIDType=Standard (11-bit identifier)  MsgIdentifier=1095  MsgLength=8  SignalInfo={ 'AZ_Winkel', '22', '10', 'LE', 'unsigned', 'Multiplexed', '0', '0.16', '-81.76', '-81.76', '81.92'; 'EL_Angle', '37', '10', 'LE', 'unsigned', 'Multiplexed', '1', '0.04', '-20.44', '-20.44', '20.48'; 'Internal_used', '14', '8', 'LE', 'unsigned', 'Multiplexed', '0', '1', '0', '-Inf', 'Inf'; 'Internal_used2', '32', '7', 'LE', 'unsigned', 'Multiplexed', '0', '1', '0', '-Inf', 'Inf'; 'Internal_used3', '51', '7', 'LE', 'unsigned', 'Multiplexed', '0', '1', '0', '-Inf', 'Inf'; 'Internal_used4', '58', '6', 'LE', 'unsigned', 'Multiplexed', '0', '1', '0', '-Inf', 'Inf'; 'Internal_used5', '9', '8', 'LE', 'unsigned', 'Multiplexed', '1', '1', '0', '-Inf', 'Inf'; 'Internal_used6', '17', '8', 'LE', 'unsigned', 'Multiplexed', '1', '1', '0', '-Inf', 'Inf'; 'Internal_used7', '25', '7', 'LE', 'unsigned', 'Multiplexed', '1', '1', '0', '-Inf', 'Inf'; 'Mode_Signal', '0', '1', 'LE', 'unsigned', 'Multiplexor', '0', '1', '0', '0', '1'; 'RCS', '1', '7', 'LE', 'unsigned', 'Multiplexed', '1', '0.2', '-15', '-15', '36'; 'Range1', '1', '13', 'LE', 'unsigned', 'Multiplexed', '0', '0.04', '0', '0', '327.64'; 'Reserve_3', '32', '5', 'LE', 'unsigned', 'Multiplexed', '1', '1', '0', '-Inf', 'Inf'; 'Reserve_4', '47', '16', 'LE', 'unsigned', 'Multiplexed', '1', '1', '0', '-Inf', 'Inf'; 'Speed_Radial', '39', '12', 'LE', 'unsigned', 'Multiplexed', '0', '0.04', '-119.68', '-44.12', '119.68' }  IDPort=on  TimestampPort=on  ErrorPort=off  RemotePort=off  LengthPort=off  StatusPort=off  ApplyMinMax=off
      settings: SourceProductBaseCode=ME,XP,VN  DataFormat=CANdb specified signals
  CAN Unpack73 : canmsglib/CAN Unpack  CANdbFile=eWolf_SensorCAN.dbc  MsgList=Radar_RawTarget_Data_072  MsgName=Radar_RawTarget_Data_072  MsgIDType=Standard (11-bit identifier)  MsgIdentifier=1096  MsgLength=8  SignalInfo={ 'AZ_Winkel', '22', '10', 'LE', 'unsigned', 'Multiplexed', '0', '0.16', '-81.76', '-81.76', '81.92'; 'EL_Angle', '37', '10', 'LE', 'unsigned', 'Multiplexed', '1', '0.04', '-20.44', '-20.44', '20.48'; 'Internal_used', '14', '8', 'LE', 'unsigned', 'Multiplexed', '0', '1', '0', '-Inf', 'Inf'; 'Internal_used2', '32', '7', 'LE', 'unsigned', 'Multiplexed', '0', '1', '0', '-Inf', 'Inf'; 'Internal_used3', '51', '7', 'LE', 'unsigned', 'Multiplexed', '0', '1', '0', '-Inf', 'Inf'; 'Internal_used4', '58', '6', 'LE', 'unsigned', 'Multiplexed', '0', '1', '0', '-Inf', 'Inf'; 'Internal_used5', '9', '8', 'LE', 'unsigned', 'Multiplexed', '1', '1', '0', '-Inf', 'Inf'; 'Internal_used6', '17', '8', 'LE', 'unsigned', 'Multiplexed', '1', '1', '0', '-Inf', 'Inf'; 'Internal_used7', '25', '7', 'LE', 'unsigned', 'Multiplexed', '1', '1', '0', '-Inf', 'Inf'; 'Mode_Signal', '0', '1', 'LE', 'unsigned', 'Multiplexor', '0', '1', '0', '0', '1'; 'RCS', '1', '7', 'LE', 'unsigned', 'Multiplexed', '1', '0.2', '-15', '-15', '36'; 'Range1', '1', '13', 'LE', 'unsigned', 'Multiplexed', '0', '0.04', '0', '0', '327.64'; 'Reserve_3', '32', '5', 'LE', 'unsigned', 'Multiplexed', '1', '1', '0', '-Inf', 'Inf'; 'Reserve_4', '47', '16', 'LE', 'unsigned', 'Multiplexed', '1', '1', '0', '-Inf', 'Inf'; 'Speed_Radial', '39', '12', 'LE', 'unsigned', 'Multiplexed', '0', '0.04', '-119.68', '-44.12', '119.68' }  IDPort=on  TimestampPort=on  ErrorPort=off  RemotePort=off  LengthPort=off  StatusPort=off  ApplyMinMax=off
      settings: SourceProductBaseCode=ME,XP,VN  DataFormat=CANdb specified signals
  CAN Unpack74 : canmsglib/CAN Unpack  CANdbFile=eWolf_SensorCAN.dbc  MsgList=Radar_RawTarget_Data_073  MsgName=Radar_RawTarget_Data_073  MsgIDType=Standard (11-bit identifier)  MsgIdentifier=1097  MsgLength=8  SignalInfo={ 'AZ_Winkel', '22', '10', 'LE', 'unsigned', 'Multiplexed', '0', '0.16', '-81.76', '-81.76', '81.92'; 'EL_Angle', '37', '10', 'LE', 'unsigned', 'Multiplexed', '1', '0.04', '-20.44', '-20.44', '20.48'; 'Internal_used', '14', '8', 'LE', 'unsigned', 'Multiplexed', '0', '1', '0', '-Inf', 'Inf'; 'Internal_used2', '32', '7', 'LE', 'unsigned', 'Multiplexed', '0', '1', '0', '-Inf', 'Inf'; 'Internal_used3', '51', '7', 'LE', 'unsigned', 'Multiplexed', '0', '1', '0', '-Inf', 'Inf'; 'Internal_used4', '58', '6', 'LE', 'unsigned', 'Multiplexed', '0', '1', '0', '-Inf', 'Inf'; 'Internal_used5', '9', '8', 'LE', 'unsigned', 'Multiplexed', '1', '1', '0', '-Inf', 'Inf'; 'Internal_used6', '17', '8', 'LE', 'unsigned', 'Multiplexed', '1', '1', '0', '-Inf', 'Inf'; 'Internal_used7', '25', '7', 'LE', 'unsigned', 'Multiplexed', '1', '1', '0', '-Inf', 'Inf'; 'Mode_Signal', '0', '1', 'LE', 'unsigned', 'Multiplexor', '0', '1', '0', '0', '1'; 'RCS', '1', '7', 'LE', 'unsigned', 'Multiplexed', '1', '0.2', '-15', '-15', '36'; 'Range1', '1', '13', 'LE', 'unsigned', 'Multiplexed', '0', '0.04', '0', '0', '327.64'; 'Reserve_3', '32', '5', 'LE', 'unsigned', 'Multiplexed', '1', '1', '0', '-Inf', 'Inf'; 'Reserve_4', '47', '16', 'LE', 'unsigned', 'Multiplexed', '1', '1', '0', '-Inf', 'Inf'; 'Speed_Radial', '39', '12', 'LE', 'unsigned', 'Multiplexed', '0', '0.04', '-119.68', '-44.12', '119.68' }  IDPort=on  TimestampPort=on  ErrorPort=off  RemotePort=off  LengthPort=off  StatusPort=off  ApplyMinMax=off
      settings: SourceProductBaseCode=ME,XP,VN  DataFormat=CANdb specified signals
  CAN Unpack75 : canmsglib/CAN Unpack  CANdbFile=eWolf_SensorCAN.dbc  MsgList=Radar_RawTarget_Data_074  MsgName=Radar_RawTarget_Data_074  MsgIDType=Standard (11-bit identifier)  MsgIdentifier=1098  MsgLength=8  SignalInfo={ 'AZ_Winkel', '22', '10', 'LE', 'unsigned', 'Multiplexed', '0', '0.16', '-81.76', '-81.76', '81.92'; 'EL_Angle', '37', '10', 'LE', 'unsigned', 'Multiplexed', '1', '0.04', '-20.44', '-20.44', '20.48'; 'Internal_used', '14', '8', 'LE', 'unsigned', 'Multiplexed', '0', '1', '0', '-Inf', 'Inf'; 'Internal_used2', '32', '7', 'LE', 'unsigned', 'Multiplexed', '0', '1', '0', '-Inf', 'Inf'; 'Internal_used3', '51', '7', 'LE', 'unsigned', 'Multiplexed', '0', '1', '0', '-Inf', 'Inf'; 'Internal_used4', '58', '6', 'LE', 'unsigned', 'Multiplexed', '0', '1', '0', '-Inf', 'Inf'; 'Internal_used5', '9', '8', 'LE', 'unsigned', 'Multiplexed', '1', '1', '0', '-Inf', 'Inf'; 'Internal_used6', '17', '8', 'LE', 'unsigned', 'Multiplexed', '1', '1', '0', '-Inf', 'Inf'; 'Internal_used7', '25', '7', 'LE', 'unsigned', 'Multiplexed', '1', '1', '0', '-Inf', 'Inf'; 'Mode_Signal', '0', '1', 'LE', 'unsigned', 'Multiplexor', '0', '1', '0', '0', '1'; 'RCS', '1', '7', 'LE', 'unsigned', 'Multiplexed', '1', '0.2', '-15', '-15', '36'; 'Range1', '1', '13', 'LE', 'unsigned', 'Multiplexed', '0', '0.04', '0', '0', '327.64'; 'Reserve_3', '32', '5', 'LE', 'unsigned', 'Multiplexed', '1', '1', '0', '-Inf', 'Inf'; 'Reserve_4', '47', '16', 'LE', 'unsigned', 'Multiplexed', '1', '1', '0', '-Inf', 'Inf'; 'Speed_Radial', '39', '12', 'LE', 'unsigned', 'Multiplexed', '0', '0.04', '-119.68', '-44.12', '119.68' }  IDPort=on  TimestampPort=on  ErrorPort=off  RemotePort=off  LengthPort=off  StatusPort=off  ApplyMinMax=off
      settings: SourceProductBaseCode=ME,XP,VN  DataFormat=CANdb specified signals
  CAN Unpack76 : canmsglib/CAN Unpack  CANdbFile=eWolf_SensorCAN.dbc  MsgList=Radar_RawTarget_Data_075  MsgName=Radar_RawTarget_Data_075  MsgIDType=Standard (11-bit identifier)  MsgIdentifier=1099  MsgLength=8  SignalInfo={ 'AZ_Winkel', '22', '10', 'LE', 'unsigned', 'Multiplexed', '0', '0.16', '-81.76', '-81.76', '81.92'; 'EL_Angle', '37', '10', 'LE', 'unsigned', 'Multiplexed', '1', '0.04', '-20.44', '-20.44', '20.48'; 'Internal_used', '14', '8', 'LE', 'unsigned', 'Multiplexed', '0', '1', '0', '-Inf', 'Inf'; 'Internal_used2', '32', '7', 'LE', 'unsigned', 'Multiplexed', '0', '1', '0', '-Inf', 'Inf'; 'Internal_used3', '51', '7', 'LE', 'unsigned', 'Multiplexed', '0', '1', '0', '-Inf', 'Inf'; 'Internal_used4', '58', '6', 'LE', 'unsigned', 'Multiplexed', '0', '1', '0', '-Inf', 'Inf'; 'Internal_used5', '9', '8', 'LE', 'unsigned', 'Multiplexed', '1', '1', '0', '-Inf', 'Inf'; 'Internal_used6', '17', '8', 'LE', 'unsigned', 'Multiplexed', '1', '1', '0', '-Inf', 'Inf'; 'Internal_used7', '25', '7', 'LE', 'unsigned', 'Multiplexed', '1', '1', '0', '-Inf', 'Inf'; 'Mode_Signal', '0', '1', 'LE', 'unsigned', 'Multiplexor', '0', '1', '0', '0', '1'; 'RCS', '1', '7', 'LE', 'unsigned', 'Multiplexed', '1', '0.2', '-15', '-15', '36'; 'Range1', '1', '13', 'LE', 'unsigned', 'Multiplexed', '0', '0.04', '0', '0', '327.64'; 'Reserve_3', '32', '5', 'LE', 'unsigned', 'Multiplexed', '1', '1', '0', '-Inf', 'Inf'; 'Reserve_4', '47', '16', 'LE', 'unsigned', 'Multiplexed', '1', '1', '0', '-Inf', 'Inf'; 'Speed_Radial', '39', '12', 'LE', 'unsigned', 'Multiplexed', '0', '0.04', '-119.68', '-44.12', '119.68' }  IDPort=on  TimestampPort=on  ErrorPort=off  RemotePort=off  LengthPort=off  StatusPort=off  ApplyMinMax=off
      settings: SourceProductBaseCode=ME,XP,VN  DataFormat=CANdb specified signals
  CAN Unpack77 : canmsglib/CAN Unpack  CANdbFile=eWolf_SensorCAN.dbc  MsgList=Radar_RawTarget_Data_076  MsgName=Radar_RawTarget_Data_076  MsgIDType=Standard (11-bit identifier)  MsgIdentifier=1100  MsgLength=8  SignalInfo={ 'AZ_Winkel', '22', '10', 'LE', 'unsigned', 'Multiplexed', '0', '0.16', '-81.76', '-81.76', '81.92'; 'EL_Angle', '37', '10', 'LE', 'unsigned', 'Multiplexed', '1', '0.04', '-20.44', '-20.44', '20.48'; 'Internal_used', '14', '8', 'LE', 'unsigned', 'Multiplexed', '0', '1', '0', '-Inf', 'Inf'; 'Internal_used2', '32', '7', 'LE', 'unsigned', 'Multiplexed', '0', '1', '0', '-Inf', 'Inf'; 'Internal_used3', '51', '7', 'LE', 'unsigned', 'Multiplexed', '0', '1', '0', '-Inf', 'Inf'; 'Internal_used4', '58', '6', 'LE', 'unsigned', 'Multiplexed', '0', '1', '0', '-Inf', 'Inf'; 'Internal_used5', '9', '8', 'LE', 'unsigned', 'Multiplexed', '1', '1', '0', '-Inf', 'Inf'; 'Internal_used6', '17', '8', 'LE', 'unsigned', 'Multiplexed', '1', '1', '0', '-Inf', 'Inf'; 'Internal_used7', '25', '7', 'LE', 'unsigned', 'Multiplexed', '1', '1', '0', '-Inf', 'Inf'; 'Mode_Signal', '0', '1', 'LE', 'unsigned', 'Multiplexor', '0', '1', '0', '0', '1'; 'RCS', '1', '7', 'LE', 'unsigned', 'Multiplexed', '1', '0.2', '-15', '-15', '36'; 'Range1', '1', '13', 'LE', 'unsigned', 'Multiplexed', '0', '0.04', '0', '0', '327.64'; 'Reserve_3', '32', '5', 'LE', 'unsigned', 'Multiplexed', '1', '1', '0', '-Inf', 'Inf'; 'Reserve_4', '47', '16', 'LE', 'unsigned', 'Multiplexed', '1', '1', '0', '-Inf', 'Inf'; 'Speed_Radial', '39', '12', 'LE', 'unsigned', 'Multiplexed', '0', '0.04', '-119.68', '-44.12', '119.68' }  IDPort=on  TimestampPort=on  ErrorPort=off  RemotePort=off  LengthPort=off  StatusPort=off  ApplyMinMax=off
      settings: SourceProductBaseCode=ME,XP,VN  DataFormat=CANdb specified signals
  CAN Unpack78 : canmsglib/CAN Unpack  CANdbFile=eWolf_SensorCAN.dbc  MsgList=Radar_RawTarget_Data_077  MsgName=Radar_RawTarget_Data_077  MsgIDType=Standard (11-bit identifier)  MsgIdentifier=1101  MsgLength=8  SignalInfo={ 'AZ_Winkel', '22', '10', 'LE', 'unsigned', 'Multiplexed', '0', '0.16', '-81.76', '-81.76', '81.92'; 'EL_Angle', '37', '10', 'LE', 'unsigned', 'Multiplexed', '1', '0.04', '-20.44', '-20.44', '20.48'; 'Internal_used', '14', '8', 'LE', 'unsigned', 'Multiplexed', '0', '1', '0', '-Inf', 'Inf'; 'Internal_used2', '32', '7', 'LE', 'unsigned', 'Multiplexed', '0', '1', '0', '-Inf', 'Inf'; 'Internal_used3', '51', '7', 'LE', 'unsigned', 'Multiplexed', '0', '1', '0', '-Inf', 'Inf'; 'Internal_used4', '58', '6', 'LE', 'unsigned', 'Multiplexed', '0', '1', '0', '-Inf', 'Inf'; 'Internal_used5', '9', '8', 'LE', 'unsigned', 'Multiplexed', '1', '1', '0', '-Inf', 'Inf'; 'Internal_used6', '17', '8', 'LE', 'unsigned', 'Multiplexed', '1', '1', '0', '-Inf', 'Inf'; 'Internal_used7', '25', '7', 'LE', 'unsigned', 'Multiplexed', '1', '1', '0', '-Inf', 'Inf'; 'Mode_Signal', '0', '1', 'LE', 'unsigned', 'Multiplexor', '0', '1', '0', '0', '1'; 'RCS', '1', '7', 'LE', 'unsigned', 'Multiplexed', '1', '0.2', '-15', '-15', '36'; 'Range1', '1', '13', 'LE', 'unsigned', 'Multiplexed', '0', '0.04', '0', '0', '327.64'; 'Reserve_3', '32', '5', 'LE', 'unsigned', 'Multiplexed', '1', '1', '0', '-Inf', 'Inf'; 'Reserve_4', '47', '16', 'LE', 'unsigned', 'Multiplexed', '1', '1', '0', '-Inf', 'Inf'; 'Speed_Radial', '39', '12', 'LE', 'unsigned', 'Multiplexed', '0', '0.04', '-119.68', '-44.12', '119.68' }  IDPort=on  TimestampPort=on  ErrorPort=off  RemotePort=off  LengthPort=off  StatusPort=off  ApplyMinMax=off
      settings: SourceProductBaseCode=ME,XP,VN  DataFormat=CANdb specified signals
  CAN Unpack79 : canmsglib/CAN Unpack  CANdbFile=eWolf_SensorCAN.dbc  MsgList=Radar_RawTarget_Data_078  MsgName=Radar_RawTarget_Data_078  MsgIDType=Standard (11-bit identifier)  MsgIdentifier=1102  MsgLength=8  SignalInfo={ 'AZ_Winkel', '22', '10', 'LE', 'unsigned', 'Multiplexed', '0', '0.16', '-81.76', '-81.76', '81.92'; 'EL_Angle', '37', '10', 'LE', 'unsigned', 'Multiplexed', '1', '0.04', '-20.44', '-20.44', '20.48'; 'Internal_used', '14', '8', 'LE', 'unsigned', 'Multiplexed', '0', '1', '0', '-Inf', 'Inf'; 'Internal_used2', '32', '7', 'LE', 'unsigned', 'Multiplexed', '0', '1', '0', '-Inf', 'Inf'; 'Internal_used3', '51', '7', 'LE', 'unsigned', 'Multiplexed', '0', '1', '0', '-Inf', 'Inf'; 'Internal_used4', '58', '6', 'LE', 'unsigned', 'Multiplexed', '0', '1', '0', '-Inf', 'Inf'; 'Internal_used5', '9', '8', 'LE', 'unsigned', 'Multiplexed', '1', '1', '0', '-Inf', 'Inf'; 'Internal_used6', '17', '8', 'LE', 'unsigned', 'Multiplexed', '1', '1', '0', '-Inf', 'Inf'; 'Internal_used7', '25', '7', 'LE', 'unsigned', 'Multiplexed', '1', '1', '0', '-Inf', 'Inf'; 'Mode_Signal', '0', '1', 'LE', 'unsigned', 'Multiplexor', '0', '1', '0', '0', '1'; 'RCS', '1', '7', 'LE', 'unsigned', 'Multiplexed', '1', '0.2', '-15', '-15', '36'; 'Range1', '1', '13', 'LE', 'unsigned', 'Multiplexed', '0', '0.04', '0', '0', '327.64'; 'Reserve_3', '32', '5', 'LE', 'unsigned', 'Multiplexed', '1', '1', '0', '-Inf', 'Inf'; 'Reserve_4', '47', '16', 'LE', 'unsigned', 'Multiplexed', '1', '1', '0', '-Inf', 'Inf'; 'Speed_Radial', '39', '12', 'LE', 'unsigned', 'Multiplexed', '0', '0.04', '-119.68', '-44.12', '119.68' }  IDPort=on  TimestampPort=on  ErrorPort=off  RemotePort=off  LengthPort=off  StatusPort=off  ApplyMinMax=off
      settings: SourceProductBaseCode=ME,XP,VN  DataFormat=CANdb specified signals
  CAN Unpack8 : canmsglib/CAN Unpack  CANdbFile=eWolf_SensorCAN.dbc  MsgList=Radar_RawTarget_Data_007  MsgName=Radar_RawTarget_Data_007  MsgIDType=Standard (11-bit identifier)  MsgIdentifier=1031  MsgLength=8  SignalInfo={ 'AZ_Winkel', '22', '10', 'LE', 'unsigned', 'Multiplexed', '0', '0.16', '-81.76', '-81.76', '81.92'; 'EL_Angle', '37', '10', 'LE', 'unsigned', 'Multiplexed', '1', '0.04', '-20.44', '-20.44', '20.48'; 'Internal_used', '14', '8', 'LE', 'unsigned', 'Multiplexed', '0', '1', '0', '-Inf', 'Inf'; 'Internal_used2', '32', '7', 'LE', 'unsigned', 'Multiplexed', '0', '1', '0', '-Inf', 'Inf'; 'Internal_used3', '51', '7', 'LE', 'unsigned', 'Multiplexed', '0', '1', '0', '-Inf', 'Inf'; 'Internal_used4', '58', '6', 'LE', 'unsigned', 'Multiplexed', '0', '1', '0', '-Inf', 'Inf'; 'Internal_used5', '9', '8', 'LE', 'unsigned', 'Multiplexed', '1', '1', '0', '-Inf', 'Inf'; 'Internal_used6', '17', '8', 'LE', 'unsigned', 'Multiplexed', '1', '1', '0', '-Inf', 'Inf'; 'Internal_used7', '25', '7', 'LE', 'unsigned', 'Multiplexed', '1', '1', '0', '-Inf', 'Inf'; 'Mode_Signal', '0', '1', 'LE', 'unsigned', 'Multiplexor', '0', '1', '0', '0', '1'; 'RCS', '1', '7', 'LE', 'unsigned', 'Multiplexed', '1', '0.2', '-15', '-15', '36'; 'Range1', '1', '13', 'LE', 'unsigned', 'Multiplexed', '0', '0.04', '0', '0', '327.64'; 'Reserve_3', '32', '5', 'LE', 'unsigned', 'Multiplexed', '1', '1', '0', '-Inf', 'Inf'; 'Reserve_4', '47', '16', 'LE', 'unsigned', 'Multiplexed', '1', '1', '0', '-Inf', 'Inf'; 'Speed_Radial', '39', '12', 'LE', 'unsigned', 'Multiplexed', '0', '0.04', '-119.68', '-44.12', '119.68' }  IDPort=on  TimestampPort=on  ErrorPort=off  RemotePort=off  LengthPort=off  StatusPort=off  ApplyMinMax=off
      settings: SourceProductBaseCode=ME,XP,VN  DataFormat=CANdb specified signals
  CAN Unpack80 : canmsglib/CAN Unpack  CANdbFile=eWolf_SensorCAN.dbc  MsgList=Radar_RawTarget_Data_079  MsgName=Radar_RawTarget_Data_079  MsgIDType=Standard (11-bit identifier)  MsgIdentifier=1103  MsgLength=8  SignalInfo={ 'AZ_Winkel', '22', '10', 'LE', 'unsigned', 'Multiplexed', '0', '0.16', '-81.76', '-81.76', '81.92'; 'EL_Angle', '37', '10', 'LE', 'unsigned', 'Multiplexed', '1', '0.04', '-20.44', '-20.44', '20.48'; 'Internal_used', '14', '8', 'LE', 'unsigned', 'Multiplexed', '0', '1', '0', '-Inf', 'Inf'; 'Internal_used2', '32', '7', 'LE', 'unsigned', 'Multiplexed', '0', '1', '0', '-Inf', 'Inf'; 'Internal_used3', '51', '7', 'LE', 'unsigned', 'Multiplexed', '0', '1', '0', '-Inf', 'Inf'; 'Internal_used4', '58', '6', 'LE', 'unsigned', 'Multiplexed', '0', '1', '0', '-Inf', 'Inf'; 'Internal_used5', '9', '8', 'LE', 'unsigned', 'Multiplexed', '1', '1', '0', '-Inf', 'Inf'; 'Internal_used6', '17', '8', 'LE', 'unsigned', 'Multiplexed', '1', '1', '0', '-Inf', 'Inf'; 'Internal_used7', '25', '7', 'LE', 'unsigned', 'Multiplexed', '1', '1', '0', '-Inf', 'Inf'; 'Mode_Signal', '0', '1', 'LE', 'unsigned', 'Multiplexor', '0', '1', '0', '0', '1'; 'RCS', '1', '7', 'LE', 'unsigned', 'Multiplexed', '1', '0.2', '-15', '-15', '36'; 'Range1', '1', '13', 'LE', 'unsigned', 'Multiplexed', '0', '0.04', '0', '0', '327.64'; 'Reserve_3', '32', '5', 'LE', 'unsigned', 'Multiplexed', '1', '1', '0', '-Inf', 'Inf'; 'Reserve_4', '47', '16', 'LE', 'unsigned', 'Multiplexed', '1', '1', '0', '-Inf', 'Inf'; 'Speed_Radial', '39', '12', 'LE', 'unsigned', 'Multiplexed', '0', '0.04', '-119.68', '-44.12', '119.68' }  IDPort=on  TimestampPort=on  ErrorPort=off  RemotePort=off  LengthPort=off  StatusPort=off  ApplyMinMax=off
      settings: SourceProductBaseCode=ME,XP,VN  DataFormat=CANdb specified signals
  CAN Unpack81 : canmsglib/CAN Unpack  CANdbFile=eWolf_SensorCAN.dbc  MsgList=Radar_RawTarget_Data_080  MsgName=Radar_RawTarget_Data_080  MsgIDType=Standard (11-bit identifier)  MsgIdentifier=1104  MsgLength=8  SignalInfo={ 'AZ_Winkel', '22', '10', 'LE', 'unsigned', 'Multiplexed', '0', '0.16', '-81.76', '-81.76', '81.92'; 'EL_Angle', '37', '10', 'LE', 'unsigned', 'Multiplexed', '1', '0.04', '-20.44', '-20.44', '20.48'; 'Internal_used', '14', '8', 'LE', 'unsigned', 'Multiplexed', '0', '1', '0', '-Inf', 'Inf'; 'Internal_used2', '32', '7', 'LE', 'unsigned', 'Multiplexed', '0', '1', '0', '-Inf', 'Inf'; 'Internal_used3', '51', '7', 'LE', 'unsigned', 'Multiplexed', '0', '1', '0', '-Inf', 'Inf'; 'Internal_used4', '58', '6', 'LE', 'unsigned', 'Multiplexed', '0', '1', '0', '-Inf', 'Inf'; 'Internal_used5', '9', '8', 'LE', 'unsigned', 'Multiplexed', '1', '1', '0', '-Inf', 'Inf'; 'Internal_used6', '17', '8', 'LE', 'unsigned', 'Multiplexed', '1', '1', '0', '-Inf', 'Inf'; 'Internal_used7', '25', '7', 'LE', 'unsigned', 'Multiplexed', '1', '1', '0', '-Inf', 'Inf'; 'Mode_Signal', '0', '1', 'LE', 'unsigned', 'Multiplexor', '0', '1', '0', '0', '1'; 'RCS', '1', '7', 'LE', 'unsigned', 'Multiplexed', '1', '0.2', '-15', '-15', '36'; 'Range1', '1', '13', 'LE', 'unsigned', 'Multiplexed', '0', '0.04', '0', '0', '327.64'; 'Reserve_3', '32', '5', 'LE', 'unsigned', 'Multiplexed', '1', '1', '0', '-Inf', 'Inf'; 'Reserve_4', '47', '16', 'LE', 'unsigned', 'Multiplexed', '1', '1', '0', '-Inf', 'Inf'; 'Speed_Radial', '39', '12', 'LE', 'unsigned', 'Multiplexed', '0', '0.04', '-119.68', '-44.12', '119.68' }  IDPort=on  TimestampPort=on  ErrorPort=off  RemotePort=off  LengthPort=off  StatusPort=off  ApplyMinMax=off
      settings: SourceProductBaseCode=ME,XP,VN  DataFormat=CANdb specified signals
  CAN Unpack82 : canmsglib/CAN Unpack  CANdbFile=eWolf_SensorCAN.dbc  MsgList=Radar_RawTarget_Data_081  MsgName=Radar_RawTarget_Data_081  MsgIDType=Standard (11-bit identifier)  MsgIdentifier=1105  MsgLength=8  SignalInfo={ 'AZ_Winkel', '22', '10', 'LE', 'unsigned', 'Multiplexed', '0', '0.16', '-81.76', '-81.76', '81.92'; 'EL_Angle', '37', '10', 'LE', 'unsigned', 'Multiplexed', '1', '0.04', '-20.44', '-20.44', '20.48'; 'Internal_used', '14', '8', 'LE', 'unsigned', 'Multiplexed', '0', '1', '0', '-Inf', 'Inf'; 'Internal_used2', '32', '7', 'LE', 'unsigned', 'Multiplexed', '0', '1', '0', '-Inf', 'Inf'; 'Internal_used3', '51', '7', 'LE', 'unsigned', 'Multiplexed', '0', '1', '0', '-Inf', 'Inf'; 'Internal_used4', '58', '6', 'LE', 'unsigned', 'Multiplexed', '0', '1', '0', '-Inf', 'Inf'; 'Internal_used5', '9', '8', 'LE', 'unsigned', 'Multiplexed', '1', '1', '0', '-Inf', 'Inf'; 'Internal_used6', '17', '8', 'LE', 'unsigned', 'Multiplexed', '1', '1', '0', '-Inf', 'Inf'; 'Internal_used7', '25', '7', 'LE', 'unsigned', 'Multiplexed', '1', '1', '0', '-Inf', 'Inf'; 'Mode_Signal', '0', '1', 'LE', 'unsigned', 'Multiplexor', '0', '1', '0', '0', '1'; 'RCS', '1', '7', 'LE', 'unsigned', 'Multiplexed', '1', '0.2', '-15', '-15', '36'; 'Range1', '1', '13', 'LE', 'unsigned', 'Multiplexed', '0', '0.04', '0', '0', '327.64'; 'Reserve_3', '32', '5', 'LE', 'unsigned', 'Multiplexed', '1', '1', '0', '-Inf', 'Inf'; 'Reserve_4', '47', '16', 'LE', 'unsigned', 'Multiplexed', '1', '1', '0', '-Inf', 'Inf'; 'Speed_Radial', '39', '12', 'LE', 'unsigned', 'Multiplexed', '0', '0.04', '-119.68', '-44.12', '119.68' }  IDPort=on  TimestampPort=on  ErrorPort=off  RemotePort=off  LengthPort=off  StatusPort=off  ApplyMinMax=off
      settings: SourceProductBaseCode=ME,XP,VN  DataFormat=CANdb specified signals
  CAN Unpack83 : canmsglib/CAN Unpack  CANdbFile=eWolf_SensorCAN.dbc  MsgList=Radar_RawTarget_Data_082  MsgName=Radar_RawTarget_Data_082  MsgIDType=Standard (11-bit identifier)  MsgIdentifier=1106  MsgLength=8  SignalInfo={ 'AZ_Winkel', '22', '10', 'LE', 'unsigned', 'Multiplexed', '0', '0.16', '-81.76', '-81.76', '81.92'; 'EL_Angle', '37', '10', 'LE', 'unsigned', 'Multiplexed', '1', '0.04', '-20.44', '-20.44', '20.48'; 'Internal_used', '14', '8', 'LE', 'unsigned', 'Multiplexed', '0', '1', '0', '-Inf', 'Inf'; 'Internal_used2', '32', '7', 'LE', 'unsigned', 'Multiplexed', '0', '1', '0', '-Inf', 'Inf'; 'Internal_used3', '51', '7', 'LE', 'unsigned', 'Multiplexed', '0', '1', '0', '-Inf', 'Inf'; 'Internal_used4', '58', '6', 'LE', 'unsigned', 'Multiplexed', '0', '1', '0', '-Inf', 'Inf'; 'Internal_used5', '9', '8', 'LE', 'unsigned', 'Multiplexed', '1', '1', '0', '-Inf', 'Inf'; 'Internal_used6', '17', '8', 'LE', 'unsigned', 'Multiplexed', '1', '1', '0', '-Inf', 'Inf'; 'Internal_used7', '25', '7', 'LE', 'unsigned', 'Multiplexed', '1', '1', '0', '-Inf', 'Inf'; 'Mode_Signal', '0', '1', 'LE', 'unsigned', 'Multiplexor', '0', '1', '0', '0', '1'; 'RCS', '1', '7', 'LE', 'unsigned', 'Multiplexed', '1', '0.2', '-15', '-15', '36'; 'Range1', '1', '13', 'LE', 'unsigned', 'Multiplexed', '0', '0.04', '0', '0', '327.64'; 'Reserve_3', '32', '5', 'LE', 'unsigned', 'Multiplexed', '1', '1', '0', '-Inf', 'Inf'; 'Reserve_4', '47', '16', 'LE', 'unsigned', 'Multiplexed', '1', '1', '0', '-Inf', 'Inf'; 'Speed_Radial', '39', '12', 'LE', 'unsigned', 'Multiplexed', '0', '0.04', '-119.68', '-44.12', '119.68' }  IDPort=on  TimestampPort=on  ErrorPort=off  RemotePort=off  LengthPort=off  StatusPort=off  ApplyMinMax=off
      settings: SourceProductBaseCode=ME,XP,VN  DataFormat=CANdb specified signals
  CAN Unpack84 : canmsglib/CAN Unpack  CANdbFile=eWolf_SensorCAN.dbc  MsgList=Radar_RawTarget_Data_083  MsgName=Radar_RawTarget_Data_083  MsgIDType=Standard (11-bit identifier)  MsgIdentifier=1107  MsgLength=8  SignalInfo={ 'AZ_Winkel', '22', '10', 'LE', 'unsigned', 'Multiplexed', '0', '0.16', '-81.76', '-81.76', '81.92'; 'EL_Angle', '37', '10', 'LE', 'unsigned', 'Multiplexed', '1', '0.04', '-20.44', '-20.44', '20.48'; 'Internal_used', '14', '8', 'LE', 'unsigned', 'Multiplexed', '0', '1', '0', '-Inf', 'Inf'; 'Internal_used2', '32', '7', 'LE', 'unsigned', 'Multiplexed', '0', '1', '0', '-Inf', 'Inf'; 'Internal_used3', '51', '7', 'LE', 'unsigned', 'Multiplexed', '0', '1', '0', '-Inf', 'Inf'; 'Internal_used4', '58', '6', 'LE', 'unsigned', 'Multiplexed', '0', '1', '0', '-Inf', 'Inf'; 'Internal_used5', '9', '8', 'LE', 'unsigned', 'Multiplexed', '1', '1', '0', '-Inf', 'Inf'; 'Internal_used6', '17', '8', 'LE', 'unsigned', 'Multiplexed', '1', '1', '0', '-Inf', 'Inf'; 'Internal_used7', '25', '7', 'LE', 'unsigned', 'Multiplexed', '1', '1', '0', '-Inf', 'Inf'; 'Mode_Signal', '0', '1', 'LE', 'unsigned', 'Multiplexor', '0', '1', '0', '0', '1'; 'RCS', '1', '7', 'LE', 'unsigned', 'Multiplexed', '1', '0.2', '-15', '-15', '36'; 'Range1', '1', '13', 'LE', 'unsigned', 'Multiplexed', '0', '0.04', '0', '0', '327.64'; 'Reserve_3', '32', '5', 'LE', 'unsigned', 'Multiplexed', '1', '1', '0', '-Inf', 'Inf'; 'Reserve_4', '47', '16', 'LE', 'unsigned', 'Multiplexed', '1', '1', '0', '-Inf', 'Inf'; 'Speed_Radial', '39', '12', 'LE', 'unsigned', 'Multiplexed', '0', '0.04', '-119.68', '-44.12', '119.68' }  IDPort=on  TimestampPort=on  ErrorPort=off  RemotePort=off  LengthPort=off  StatusPort=off  ApplyMinMax=off
      settings: SourceProductBaseCode=ME,XP,VN  DataFormat=CANdb specified signals
  CAN Unpack85 : canmsglib/CAN Unpack  CANdbFile=eWolf_SensorCAN.dbc  MsgList=Radar_RawTarget_Data_084  MsgName=Radar_RawTarget_Data_084  MsgIDType=Standard (11-bit identifier)  MsgIdentifier=1108  MsgLength=8  SignalInfo={ 'AZ_Winkel', '22', '10', 'LE', 'unsigned', 'Multiplexed', '0', '0.16', '-81.76', '-81.76', '81.92'; 'EL_Angle', '37', '10', 'LE', 'unsigned', 'Multiplexed', '1', '0.04', '-20.44', '-20.44', '20.48'; 'Internal_used', '14', '8', 'LE', 'unsigned', 'Multiplexed', '0', '1', '0', '-Inf', 'Inf'; 'Internal_used2', '32', '7', 'LE', 'unsigned', 'Multiplexed', '0', '1', '0', '-Inf', 'Inf'; 'Internal_used3', '51', '7', 'LE', 'unsigned', 'Multiplexed', '0', '1', '0', '-Inf', 'Inf'; 'Internal_used4', '58', '6', 'LE', 'unsigned', 'Multiplexed', '0', '1', '0', '-Inf', 'Inf'; 'Internal_used5', '9', '8', 'LE', 'unsigned', 'Multiplexed', '1', '1', '0', '-Inf', 'Inf'; 'Internal_used6', '17', '8', 'LE', 'unsigned', 'Multiplexed', '1', '1', '0', '-Inf', 'Inf'; 'Internal_used7', '25', '7', 'LE', 'unsigned', 'Multiplexed', '1', '1', '0', '-Inf', 'Inf'; 'Mode_Signal', '0', '1', 'LE', 'unsigned', 'Multiplexor', '0', '1', '0', '0', '1'; 'RCS', '1', '7', 'LE', 'unsigned', 'Multiplexed', '1', '0.2', '-15', '-15', '36'; 'Range1', '1', '13', 'LE', 'unsigned', 'Multiplexed', '0', '0.04', '0', '0', '327.64'; 'Reserve_3', '32', '5', 'LE', 'unsigned', 'Multiplexed', '1', '1', '0', '-Inf', 'Inf'; 'Reserve_4', '47', '16', 'LE', 'unsigned', 'Multiplexed', '1', '1', '0', '-Inf', 'Inf'; 'Speed_Radial', '39', '12', 'LE', 'unsigned', 'Multiplexed', '0', '0.04', '-119.68', '-44.12', '119.68' }  IDPort=on  TimestampPort=on  ErrorPort=off  RemotePort=off  LengthPort=off  StatusPort=off  ApplyMinMax=off
      settings: SourceProductBaseCode=ME,XP,VN  DataFormat=CANdb specified signals
  CAN Unpack86 : canmsglib/CAN Unpack  CANdbFile=eWolf_SensorCAN.dbc  MsgList=Radar_RawTarget_Data_085  MsgName=Radar_RawTarget_Data_085  MsgIDType=Standard (11-bit identifier)  MsgIdentifier=1109  MsgLength=8  SignalInfo={ 'AZ_Winkel', '22', '10', 'LE', 'unsigned', 'Multiplexed', '0', '0.16', '-81.76', '-81.76', '81.92'; 'EL_Angle', '37', '10', 'LE', 'unsigned', 'Multiplexed', '1', '0.04', '-20.44', '-20.44', '20.48'; 'Internal_used', '14', '8', 'LE', 'unsigned', 'Multiplexed', '0', '1', '0', '-Inf', 'Inf'; 'Internal_used2', '32', '7', 'LE', 'unsigned', 'Multiplexed', '0', '1', '0', '-Inf', 'Inf'; 'Internal_used3', '51', '7', 'LE', 'unsigned', 'Multiplexed', '0', '1', '0', '-Inf', 'Inf'; 'Internal_used4', '58', '6', 'LE', 'unsigned', 'Multiplexed', '0', '1', '0', '-Inf', 'Inf'; 'Internal_used5', '9', '8', 'LE', 'unsigned', 'Multiplexed', '1', '1', '0', '-Inf', 'Inf'; 'Internal_used6', '17', '8', 'LE', 'unsigned', 'Multiplexed', '1', '1', '0', '-Inf', 'Inf'; 'Internal_used7', '25', '7', 'LE', 'unsigned', 'Multiplexed', '1', '1', '0', '-Inf', 'Inf'; 'Mode_Signal', '0', '1', 'LE', 'unsigned', 'Multiplexor', '0', '1', '0', '0', '1'; 'RCS', '1', '7', 'LE', 'unsigned', 'Multiplexed', '1', '0.2', '-15', '-15', '36'; 'Range1', '1', '13', 'LE', 'unsigned', 'Multiplexed', '0', '0.04', '0', '0', '327.64'; 'Reserve_3', '32', '5', 'LE', 'unsigned', 'Multiplexed', '1', '1', '0', '-Inf', 'Inf'; 'Reserve_4', '47', '16', 'LE', 'unsigned', 'Multiplexed', '1', '1', '0', '-Inf', 'Inf'; 'Speed_Radial', '39', '12', 'LE', 'unsigned', 'Multiplexed', '0', '0.04', '-119.68', '-44.12', '119.68' }  IDPort=on  TimestampPort=on  ErrorPort=off  RemotePort=off  LengthPort=off  StatusPort=off  ApplyMinMax=off
      settings: SourceProductBaseCode=ME,XP,VN  DataFormat=CANdb specified signals
  CAN Unpack87 : canmsglib/CAN Unpack  CANdbFile=eWolf_SensorCAN.dbc  MsgList=Radar_RawTarget_Data_086  MsgName=Radar_RawTarget_Data_086  MsgIDType=Standard (11-bit identifier)  MsgIdentifier=1110  MsgLength=8  SignalInfo={ 'AZ_Winkel', '22', '10', 'LE', 'unsigned', 'Multiplexed', '0', '0.16', '-81.76', '-81.76', '81.92'; 'EL_Angle', '37', '10', 'LE', 'unsigned', 'Multiplexed', '1', '0.04', '-20.44', '-20.44', '20.48'; 'Internal_used', '14', '8', 'LE', 'unsigned', 'Multiplexed', '0', '1', '0', '-Inf', 'Inf'; 'Internal_used2', '32', '7', 'LE', 'unsigned', 'Multiplexed', '0', '1', '0', '-Inf', 'Inf'; 'Internal_used3', '51', '7', 'LE', 'unsigned', 'Multiplexed', '0', '1', '0', '-Inf', 'Inf'; 'Internal_used4', '58', '6', 'LE', 'unsigned', 'Multiplexed', '0', '1', '0', '-Inf', 'Inf'; 'Internal_used5', '9', '8', 'LE', 'unsigned', 'Multiplexed', '1', '1', '0', '-Inf', 'Inf'; 'Internal_used6', '17', '8', 'LE', 'unsigned', 'Multiplexed', '1', '1', '0', '-Inf', 'Inf'; 'Internal_used7', '25', '7', 'LE', 'unsigned', 'Multiplexed', '1', '1', '0', '-Inf', 'Inf'; 'Mode_Signal', '0', '1', 'LE', 'unsigned', 'Multiplexor', '0', '1', '0', '0', '1'; 'RCS', '1', '7', 'LE', 'unsigned', 'Multiplexed', '1', '0.2', '-15', '-15', '36'; 'Range1', '1', '13', 'LE', 'unsigned', 'Multiplexed', '0', '0.04', '0', '0', '327.64'; 'Reserve_3', '32', '5', 'LE', 'unsigned', 'Multiplexed', '1', '1', '0', '-Inf', 'Inf'; 'Reserve_4', '47', '16', 'LE', 'unsigned', 'Multiplexed', '1', '1', '0', '-Inf', 'Inf'; 'Speed_Radial', '39', '12', 'LE', 'unsigned', 'Multiplexed', '0', '0.04', '-119.68', '-44.12', '119.68' }  IDPort=on  TimestampPort=on  ErrorPort=off  RemotePort=off  LengthPort=off  StatusPort=off  ApplyMinMax=off
      settings: SourceProductBaseCode=ME,XP,VN  DataFormat=CANdb specified signals
  CAN Unpack88 : canmsglib/CAN Unpack  CANdbFile=eWolf_SensorCAN.dbc  MsgList=Radar_RawTarget_Data_087  MsgName=Radar_RawTarget_Data_087  MsgIDType=Standard (11-bit identifier)  MsgIdentifier=1111  MsgLength=8  SignalInfo={ 'AZ_Winkel', '22', '10', 'LE', 'unsigned', 'Multiplexed', '0', '0.16', '-81.76', '-81.76', '81.92'; 'EL_Angle', '37', '10', 'LE', 'unsigned', 'Multiplexed', '1', '0.04', '-20.44', '-20.44', '20.48'; 'Internal_used', '14', '8', 'LE', 'unsigned', 'Multiplexed', '0', '1', '0', '-Inf', 'Inf'; 'Internal_used2', '32', '7', 'LE', 'unsigned', 'Multiplexed', '0', '1', '0', '-Inf', 'Inf'; 'Internal_used3', '51', '7', 'LE', 'unsigned', 'Multiplexed', '0', '1', '0', '-Inf', 'Inf'; 'Internal_used4', '58', '6', 'LE', 'unsigned', 'Multiplexed', '0', '1', '0', '-Inf', 'Inf'; 'Internal_used5', '9', '8', 'LE', 'unsigned', 'Multiplexed', '1', '1', '0', '-Inf', 'Inf'; 'Internal_used6', '17', '8', 'LE', 'unsigned', 'Multiplexed', '1', '1', '0', '-Inf', 'Inf'; 'Internal_used7', '25', '7', 'LE', 'unsigned', 'Multiplexed', '1', '1', '0', '-Inf', 'Inf'; 'Mode_Signal', '0', '1', 'LE', 'unsigned', 'Multiplexor', '0', '1', '0', '0', '1'; 'RCS', '1', '7', 'LE', 'unsigned', 'Multiplexed', '1', '0.2', '-15', '-15', '36'; 'Range1', '1', '13', 'LE', 'unsigned', 'Multiplexed', '0', '0.04', '0', '0', '327.64'; 'Reserve_3', '32', '5', 'LE', 'unsigned', 'Multiplexed', '1', '1', '0', '-Inf', 'Inf'; 'Reserve_4', '47', '16', 'LE', 'unsigned', 'Multiplexed', '1', '1', '0', '-Inf', 'Inf'; 'Speed_Radial', '39', '12', 'LE', 'unsigned', 'Multiplexed', '0', '0.04', '-119.68', '-44.12', '119.68' }  IDPort=on  TimestampPort=on  ErrorPort=off  RemotePort=off  LengthPort=off  StatusPort=off  ApplyMinMax=off
      settings: SourceProductBaseCode=ME,XP,VN  DataFormat=CANdb specified signals
  CAN Unpack89 : canmsglib/CAN Unpack  CANdbFile=eWolf_SensorCAN.dbc  MsgList=Radar_RawTarget_Data_088  MsgName=Radar_RawTarget_Data_088  MsgIDType=Standard (11-bit identifier)  MsgIdentifier=1112  MsgLength=8  SignalInfo={ 'AZ_Winkel', '22', '10', 'LE', 'unsigned', 'Multiplexed', '0', '0.16', '-81.76', '-81.76', '81.92'; 'EL_Angle', '37', '10', 'LE', 'unsigned', 'Multiplexed', '1', '0.04', '-20.44', '-20.44', '20.48'; 'Internal_used', '14', '8', 'LE', 'unsigned', 'Multiplexed', '0', '1', '0', '-Inf', 'Inf'; 'Internal_used2', '32', '7', 'LE', 'unsigned', 'Multiplexed', '0', '1', '0', '-Inf', 'Inf'; 'Internal_used3', '51', '7', 'LE', 'unsigned', 'Multiplexed', '0', '1', '0', '-Inf', 'Inf'; 'Internal_used4', '58', '6', 'LE', 'unsigned', 'Multiplexed', '0', '1', '0', '-Inf', 'Inf'; 'Internal_used5', '9', '8', 'LE', 'unsigned', 'Multiplexed', '1', '1', '0', '-Inf', 'Inf'; 'Internal_used6', '17', '8', 'LE', 'unsigned', 'Multiplexed', '1', '1', '0', '-Inf', 'Inf'; 'Internal_used7', '25', '7', 'LE', 'unsigned', 'Multiplexed', '1', '1', '0', '-Inf', 'Inf'; 'Mode_Signal', '0', '1', 'LE', 'unsigned', 'Multiplexor', '0', '1', '0', '0', '1'; 'RCS', '1', '7', 'LE', 'unsigned', 'Multiplexed', '1', '0.2', '-15', '-15', '36'; 'Range1', '1', '13', 'LE', 'unsigned', 'Multiplexed', '0', '0.04', '0', '0', '327.64'; 'Reserve_3', '32', '5', 'LE', 'unsigned', 'Multiplexed', '1', '1', '0', '-Inf', 'Inf'; 'Reserve_4', '47', '16', 'LE', 'unsigned', 'Multiplexed', '1', '1', '0', '-Inf', 'Inf'; 'Speed_Radial', '39', '12', 'LE', 'unsigned', 'Multiplexed', '0', '0.04', '-119.68', '-44.12', '119.68' }  IDPort=on  TimestampPort=on  ErrorPort=off  RemotePort=off  LengthPort=off  StatusPort=off  ApplyMinMax=off
      settings: SourceProductBaseCode=ME,XP,VN  DataFormat=CANdb specified signals
  CAN Unpack9 : canmsglib/CAN Unpack  CANdbFile=eWolf_SensorCAN.dbc  MsgList=Radar_RawTarget_Data_008  MsgName=Radar_RawTarget_Data_008  MsgIDType=Standard (11-bit identifier)  MsgIdentifier=1032  MsgLength=8  SignalInfo={ 'AZ_Winkel', '22', '10', 'LE', 'unsigned', 'Multiplexed', '0', '0.16', '-81.76', '-81.76', '81.92'; 'EL_Angle', '37', '10', 'LE', 'unsigned', 'Multiplexed', '1', '0.04', '-20.44', '-20.44', '20.48'; 'Internal_used', '14', '8', 'LE', 'unsigned', 'Multiplexed', '0', '1', '0', '-Inf', 'Inf'; 'Internal_used2', '32', '7', 'LE', 'unsigned', 'Multiplexed', '0', '1', '0', '-Inf', 'Inf'; 'Internal_used3', '51', '7', 'LE', 'unsigned', 'Multiplexed', '0', '1', '0', '-Inf', 'Inf'; 'Internal_used4', '58', '6', 'LE', 'unsigned', 'Multiplexed', '0', '1', '0', '-Inf', 'Inf'; 'Internal_used5', '9', '8', 'LE', 'unsigned', 'Multiplexed', '1', '1', '0', '-Inf', 'Inf'; 'Internal_used6', '17', '8', 'LE', 'unsigned', 'Multiplexed', '1', '1', '0', '-Inf', 'Inf'; 'Internal_used7', '25', '7', 'LE', 'unsigned', 'Multiplexed', '1', '1', '0', '-Inf', 'Inf'; 'Mode_Signal', '0', '1', 'LE', 'unsigned', 'Multiplexor', '0', '1', '0', '0', '1'; 'RCS', '1', '7', 'LE', 'unsigned', 'Multiplexed', '1', '0.2', '-15', '-15', '36'; 'Range1', '1', '13', 'LE', 'unsigned', 'Multiplexed', '0', '0.04', '0', '0', '327.64'; 'Reserve_3', '32', '5', 'LE', 'unsigned', 'Multiplexed', '1', '1', '0', '-Inf', 'Inf'; 'Reserve_4', '47', '16', 'LE', 'unsigned', 'Multiplexed', '1', '1', '0', '-Inf', 'Inf'; 'Speed_Radial', '39', '12', 'LE', 'unsigned', 'Multiplexed', '0', '0.04', '-119.68', '-44.12', '119.68' }  IDPort=on  TimestampPort=on  ErrorPort=off  RemotePort=off  LengthPort=off  StatusPort=off  ApplyMinMax=off
      settings: SourceProductBaseCode=ME,XP,VN  DataFormat=CANdb specified signals
  CAN Unpack90 : canmsglib/CAN Unpack  CANdbFile=eWolf_SensorCAN.dbc  MsgList=Radar_RawTarget_Data_089  MsgName=Radar_RawTarget_Data_089  MsgIDType=Standard (11-bit identifier)  MsgIdentifier=1113  MsgLength=8  SignalInfo={ 'AZ_Winkel', '22', '10', 'LE', 'unsigned', 'Multiplexed', '0', '0.16', '-81.76', '-81.76', '81.92'; 'EL_Angle', '37', '10', 'LE', 'unsigned', 'Multiplexed', '1', '0.04', '-20.44', '-20.44', '20.48'; 'Internal_used', '14', '8', 'LE', 'unsigned', 'Multiplexed', '0', '1', '0', '-Inf', 'Inf'; 'Internal_used2', '32', '7', 'LE', 'unsigned', 'Multiplexed', '0', '1', '0', '-Inf', 'Inf'; 'Internal_used3', '51', '7', 'LE', 'unsigned', 'Multiplexed', '0', '1', '0', '-Inf', 'Inf'; 'Internal_used4', '58', '6', 'LE', 'unsigned', 'Multiplexed', '0', '1', '0', '-Inf', 'Inf'; 'Internal_used5', '9', '8', 'LE', 'unsigned', 'Multiplexed', '1', '1', '0', '-Inf', 'Inf'; 'Internal_used6', '17', '8', 'LE', 'unsigned', 'Multiplexed', '1', '1', '0', '-Inf', 'Inf'; 'Internal_used7', '25', '7', 'LE', 'unsigned', 'Multiplexed', '1', '1', '0', '-Inf', 'Inf'; 'Mode_Signal', '0', '1', 'LE', 'unsigned', 'Multiplexor', '0', '1', '0', '0', '1'; 'RCS', '1', '7', 'LE', 'unsigned', 'Multiplexed', '1', '0.2', '-15', '-15', '36'; 'Range1', '1', '13', 'LE', 'unsigned', 'Multiplexed', '0', '0.04', '0', '0', '327.64'; 'Reserve_3', '32', '5', 'LE', 'unsigned', 'Multiplexed', '1', '1', '0', '-Inf', 'Inf'; 'Reserve_4', '47', '16', 'LE', 'unsigned', 'Multiplexed', '1', '1', '0', '-Inf', 'Inf'; 'Speed_Radial', '39', '12', 'LE', 'unsigned', 'Multiplexed', '0', '0.04', '-119.68', '-44.12', '119.68' }  IDPort=on  TimestampPort=on  ErrorPort=off  RemotePort=off  LengthPort=off  StatusPort=off  ApplyMinMax=off
      settings: SourceProductBaseCode=ME,XP,VN  DataFormat=CANdb specified signals
  CAN Unpack91 : canmsglib/CAN Unpack  CANdbFile=eWolf_SensorCAN.dbc  MsgList=Radar_RawTarget_Data_090  MsgName=Radar_RawTarget_Data_090  MsgIDType=Standard (11-bit identifier)  MsgIdentifier=1114  MsgLength=8  SignalInfo={ 'AZ_Winkel', '22', '10', 'LE', 'unsigned', 'Multiplexed', '0', '0.16', '-81.76', '-81.76', '81.92'; 'EL_Angle', '37', '10', 'LE', 'unsigned', 'Multiplexed', '1', '0.04', '-20.44', '-20.44', '20.48'; 'Internal_used', '14', '8', 'LE', 'unsigned', 'Multiplexed', '0', '1', '0', '-Inf', 'Inf'; 'Internal_used2', '32', '7', 'LE', 'unsigned', 'Multiplexed', '0', '1', '0', '-Inf', 'Inf'; 'Internal_used3', '51', '7', 'LE', 'unsigned', 'Multiplexed', '0', '1', '0', '-Inf', 'Inf'; 'Internal_used4', '58', '6', 'LE', 'unsigned', 'Multiplexed', '0', '1', '0', '-Inf', 'Inf'; 'Internal_used5', '9', '8', 'LE', 'unsigned', 'Multiplexed', '1', '1', '0', '-Inf', 'Inf'; 'Internal_used6', '17', '8', 'LE', 'unsigned', 'Multiplexed', '1', '1', '0', '-Inf', 'Inf'; 'Internal_used7', '25', '7', 'LE', 'unsigned', 'Multiplexed', '1', '1', '0', '-Inf', 'Inf'; 'Mode_Signal', '0', '1', 'LE', 'unsigned', 'Multiplexor', '0', '1', '0', '0', '1'; 'RCS', '1', '7', 'LE', 'unsigned', 'Multiplexed', '1', '0.2', '-15', '-15', '36'; 'Range1', '1', '13', 'LE', 'unsigned', 'Multiplexed', '0', '0.04', '0', '0', '327.64'; 'Reserve_3', '32', '5', 'LE', 'unsigned', 'Multiplexed', '1', '1', '0', '-Inf', 'Inf'; 'Reserve_4', '47', '16', 'LE', 'unsigned', 'Multiplexed', '1', '1', '0', '-Inf', 'Inf'; 'Speed_Radial', '39', '12', 'LE', 'unsigned', 'Multiplexed', '0', '0.04', '-119.68', '-44.12', '119.68' }  IDPort=on  TimestampPort=on  ErrorPort=off  RemotePort=off  LengthPort=off  StatusPort=off  ApplyMinMax=off
      settings: SourceProductBaseCode=ME,XP,VN  DataFormat=CANdb specified signals
  CAN Unpack92 : canmsglib/CAN Unpack  CANdbFile=eWolf_SensorCAN.dbc  MsgList=Radar_RawTarget_Data_091  MsgName=Radar_RawTarget_Data_091  MsgIDType=Standard (11-bit identifier)  MsgIdentifier=1115  MsgLength=8  SignalInfo={ 'AZ_Winkel', '22', '10', 'LE', 'unsigned', 'Multiplexed', '0', '0.16', '-81.76', '-81.76', '81.92'; 'EL_Angle', '37', '10', 'LE', 'unsigned', 'Multiplexed', '1', '0.04', '-20.44', '-20.44', '20.48'; 'Internal_used', '14', '8', 'LE', 'unsigned', 'Multiplexed', '0', '1', '0', '-Inf', 'Inf'; 'Internal_used2', '32', '7', 'LE', 'unsigned', 'Multiplexed', '0', '1', '0', '-Inf', 'Inf'; 'Internal_used3', '51', '7', 'LE', 'unsigned', 'Multiplexed', '0', '1', '0', '-Inf', 'Inf'; 'Internal_used4', '58', '6', 'LE', 'unsigned', 'Multiplexed', '0', '1', '0', '-Inf', 'Inf'; 'Internal_used5', '9', '8', 'LE', 'unsigned', 'Multiplexed', '1', '1', '0', '-Inf', 'Inf'; 'Internal_used6', '17', '8', 'LE', 'unsigned', 'Multiplexed', '1', '1', '0', '-Inf', 'Inf'; 'Internal_used7', '25', '7', 'LE', 'unsigned', 'Multiplexed', '1', '1', '0', '-Inf', 'Inf'; 'Mode_Signal', '0', '1', 'LE', 'unsigned', 'Multiplexor', '0', '1', '0', '0', '1'; 'RCS', '1', '7', 'LE', 'unsigned', 'Multiplexed', '1', '0.2', '-15', '-15', '36'; 'Range1', '1', '13', 'LE', 'unsigned', 'Multiplexed', '0', '0.04', '0', '0', '327.64'; 'Reserve_3', '32', '5', 'LE', 'unsigned', 'Multiplexed', '1', '1', '0', '-Inf', 'Inf'; 'Reserve_4', '47', '16', 'LE', 'unsigned', 'Multiplexed', '1', '1', '0', '-Inf', 'Inf'; 'Speed_Radial', '39', '12', 'LE', 'unsigned', 'Multiplexed', '0', '0.04', '-119.68', '-44.12', '119.68' }  IDPort=on  TimestampPort=on  ErrorPort=off  RemotePort=off  LengthPort=off  StatusPort=off  ApplyMinMax=off
      settings: SourceProductBaseCode=ME,XP,VN  DataFormat=CANdb specified signals
  CAN Unpack93 : canmsglib/CAN Unpack  CANdbFile=eWolf_SensorCAN.dbc  MsgList=Radar_RawTarget_Data_092  MsgName=Radar_RawTarget_Data_092  MsgIDType=Standard (11-bit identifier)  MsgIdentifier=1116  MsgLength=8  SignalInfo={ 'AZ_Winkel', '22', '10', 'LE', 'unsigned', 'Multiplexed', '0', '0.16', '-81.76', '-81.76', '81.92'; 'EL_Angle', '37', '10', 'LE', 'unsigned', 'Multiplexed', '1', '0.04', '-20.44', '-20.44', '20.48'; 'Internal_used', '14', '8', 'LE', 'unsigned', 'Multiplexed', '0', '1', '0', '-Inf', 'Inf'; 'Internal_used2', '32', '7', 'LE', 'unsigned', 'Multiplexed', '0', '1', '0', '-Inf', 'Inf'; 'Internal_used3', '51', '7', 'LE', 'unsigned', 'Multiplexed', '0', '1', '0', '-Inf', 'Inf'; 'Internal_used4', '58', '6', 'LE', 'unsigned', 'Multiplexed', '0', '1', '0', '-Inf', 'Inf'; 'Internal_used5', '9', '8', 'LE', 'unsigned', 'Multiplexed', '1', '1', '0', '-Inf', 'Inf'; 'Internal_used6', '17', '8', 'LE', 'unsigned', 'Multiplexed', '1', '1', '0', '-Inf', 'Inf'; 'Internal_used7', '25', '7', 'LE', 'unsigned', 'Multiplexed', '1', '1', '0', '-Inf', 'Inf'; 'Mode_Signal', '0', '1', 'LE', 'unsigned', 'Multiplexor', '0', '1', '0', '0', '1'; 'RCS', '1', '7', 'LE', 'unsigned', 'Multiplexed', '1', '0.2', '-15', '-15', '36'; 'Range1', '1', '13', 'LE', 'unsigned', 'Multiplexed', '0', '0.04', '0', '0', '327.64'; 'Reserve_3', '32', '5', 'LE', 'unsigned', 'Multiplexed', '1', '1', '0', '-Inf', 'Inf'; 'Reserve_4', '47', '16', 'LE', 'unsigned', 'Multiplexed', '1', '1', '0', '-Inf', 'Inf'; 'Speed_Radial', '39', '12', 'LE', 'unsigned', 'Multiplexed', '0', '0.04', '-119.68', '-44.12', '119.68' }  IDPort=on  TimestampPort=on  ErrorPort=off  RemotePort=off  LengthPort=off  StatusPort=off  ApplyMinMax=off
      settings: SourceProductBaseCode=ME,XP,VN  DataFormat=CANdb specified signals
  CAN Unpack94 : canmsglib/CAN Unpack  CANdbFile=eWolf_SensorCAN.dbc  MsgList=Radar_RawTarget_Data_093  MsgName=Radar_RawTarget_Data_093  MsgIDType=Standard (11-bit identifier)  MsgIdentifier=1117  MsgLength=8  SignalInfo={ 'AZ_Winkel', '22', '10', 'LE', 'unsigned', 'Multiplexed', '0', '0.16', '-81.76', '-81.76', '81.92'; 'EL_Angle', '37', '10', 'LE', 'unsigned', 'Multiplexed', '1', '0.04', '-20.44', '-20.44', '20.48'; 'Internal_used', '14', '8', 'LE', 'unsigned', 'Multiplexed', '0', '1', '0', '-Inf', 'Inf'; 'Internal_used2', '32', '7', 'LE', 'unsigned', 'Multiplexed', '0', '1', '0', '-Inf', 'Inf'; 'Internal_used3', '51', '7', 'LE', 'unsigned', 'Multiplexed', '0', '1', '0', '-Inf', 'Inf'; 'Internal_used4', '58', '6', 'LE', 'unsigned', 'Multiplexed', '0', '1', '0', '-Inf', 'Inf'; 'Internal_used5', '9', '8', 'LE', 'unsigned', 'Multiplexed', '1', '1', '0', '-Inf', 'Inf'; 'Internal_used6', '17', '8', 'LE', 'unsigned', 'Multiplexed', '1', '1', '0', '-Inf', 'Inf'; 'Internal_used7', '25', '7', 'LE', 'unsigned', 'Multiplexed', '1', '1', '0', '-Inf', 'Inf'; 'Mode_Signal', '0', '1', 'LE', 'unsigned', 'Multiplexor', '0', '1', '0', '0', '1'; 'RCS', '1', '7', 'LE', 'unsigned', 'Multiplexed', '1', '0.2', '-15', '-15', '36'; 'Range1', '1', '13', 'LE', 'unsigned', 'Multiplexed', '0', '0.04', '0', '0', '327.64'; 'Reserve_3', '32', '5', 'LE', 'unsigned', 'Multiplexed', '1', '1', '0', '-Inf', 'Inf'; 'Reserve_4', '47', '16', 'LE', 'unsigned', 'Multiplexed', '1', '1', '0', '-Inf', 'Inf'; 'Speed_Radial', '39', '12', 'LE', 'unsigned', 'Multiplexed', '0', '0.04', '-119.68', '-44.12', '119.68' }  IDPort=on  TimestampPort=on  ErrorPort=off  RemotePort=off  LengthPort=off  StatusPort=off  ApplyMinMax=off
      settings: SourceProductBaseCode=ME,XP,VN  DataFormat=CANdb specified signals
  CAN Unpack95 : canmsglib/CAN Unpack  CANdbFile=eWolf_SensorCAN.dbc  MsgList=Radar_RawTarget_Data_094  MsgName=Radar_RawTarget_Data_094  MsgIDType=Standard (11-bit identifier)  MsgIdentifier=1118  MsgLength=8  SignalInfo={ 'AZ_Winkel', '22', '10', 'LE', 'unsigned', 'Multiplexed', '0', '0.16', '-81.76', '-81.76', '81.92'; 'EL_Angle', '37', '10', 'LE', 'unsigned', 'Multiplexed', '1', '0.04', '-20.44', '-20.44', '20.48'; 'Internal_used', '14', '8', 'LE', 'unsigned', 'Multiplexed', '0', '1', '0', '-Inf', 'Inf'; 'Internal_used2', '32', '7', 'LE', 'unsigned', 'Multiplexed', '0', '1', '0', '-Inf', 'Inf'; 'Internal_used3', '51', '7', 'LE', 'unsigned', 'Multiplexed', '0', '1', '0', '-Inf', 'Inf'; 'Internal_used4', '58', '6', 'LE', 'unsigned', 'Multiplexed', '0', '1', '0', '-Inf', 'Inf'; 'Internal_used5', '9', '8', 'LE', 'unsigned', 'Multiplexed', '1', '1', '0', '-Inf', 'Inf'; 'Internal_used6', '17', '8', 'LE', 'unsigned', 'Multiplexed', '1', '1', '0', '-Inf', 'Inf'; 'Internal_used7', '25', '7', 'LE', 'unsigned', 'Multiplexed', '1', '1', '0', '-Inf', 'Inf'; 'Mode_Signal', '0', '1', 'LE', 'unsigned', 'Multiplexor', '0', '1', '0', '0', '1'; 'RCS', '1', '7', 'LE', 'unsigned', 'Multiplexed', '1', '0.2', '-15', '-15', '36'; 'Range1', '1', '13', 'LE', 'unsigned', 'Multiplexed', '0', '0.04', '0', '0', '327.64'; 'Reserve_3', '32', '5', 'LE', 'unsigned', 'Multiplexed', '1', '1', '0', '-Inf', 'Inf'; 'Reserve_4', '47', '16', 'LE', 'unsigned', 'Multiplexed', '1', '1', '0', '-Inf', 'Inf'; 'Speed_Radial', '39', '12', 'LE', 'unsigned', 'Multiplexed', '0', '0.04', '-119.68', '-44.12', '119.68' }  IDPort=on  TimestampPort=on  ErrorPort=off  RemotePort=off  LengthPort=off  StatusPort=off  ApplyMinMax=off
      settings: SourceProductBaseCode=ME,XP,VN  DataFormat=CANdb specified signals
  CAN Unpack96 : canmsglib/CAN Unpack  CANdbFile=eWolf_SensorCAN.dbc  MsgList=Radar_RawTarget_Data_095  MsgName=Radar_RawTarget_Data_095  MsgIDType=Standard (11-bit identifier)  MsgIdentifier=1119  MsgLength=8  SignalInfo={ 'AZ_Winkel', '22', '10', 'LE', 'unsigned', 'Multiplexed', '0', '0.16', '-81.76', '-81.76', '81.92'; 'EL_Angle', '37', '10', 'LE', 'unsigned', 'Multiplexed', '1', '0.04', '-20.44', '-20.44', '20.48'; 'Internal_used', '14', '8', 'LE', 'unsigned', 'Multiplexed', '0', '1', '0', '-Inf', 'Inf'; 'Internal_used2', '32', '7', 'LE', 'unsigned', 'Multiplexed', '0', '1', '0', '-Inf', 'Inf'; 'Internal_used3', '51', '7', 'LE', 'unsigned', 'Multiplexed', '0', '1', '0', '-Inf', 'Inf'; 'Internal_used4', '58', '6', 'LE', 'unsigned', 'Multiplexed', '0', '1', '0', '-Inf', 'Inf'; 'Internal_used5', '9', '8', 'LE', 'unsigned', 'Multiplexed', '1', '1', '0', '-Inf', 'Inf'; 'Internal_used6', '17', '8', 'LE', 'unsigned', 'Multiplexed', '1', '1', '0', '-Inf', 'Inf'; 'Internal_used7', '25', '7', 'LE', 'unsigned', 'Multiplexed', '1', '1', '0', '-Inf', 'Inf'; 'Mode_Signal', '0', '1', 'LE', 'unsigned', 'Multiplexor', '0', '1', '0', '0', '1'; 'RCS', '1', '7', 'LE', 'unsigned', 'Multiplexed', '1', '0.2', '-15', '-15', '36'; 'Range1', '1', '13', 'LE', 'unsigned', 'Multiplexed', '0', '0.04', '0', '0', '327.64'; 'Reserve_3', '32', '5', 'LE', 'unsigned', 'Multiplexed', '1', '1', '0', '-Inf', 'Inf'; 'Reserve_4', '47', '16', 'LE', 'unsigned', 'Multiplexed', '1', '1', '0', '-Inf', 'Inf'; 'Speed_Radial', '39', '12', 'LE', 'unsigned', 'Multiplexed', '0', '0.04', '-119.68', '-44.12', '119.68' }  IDPort=on  TimestampPort=on  ErrorPort=off  RemotePort=off  LengthPort=off  StatusPort=off  ApplyMinMax=off
      settings: SourceProductBaseCode=ME,XP,VN  DataFormat=CANdb specified signals
  CAN Unpack97 : canmsglib/CAN Unpack  CANdbFile=eWolf_SensorCAN.dbc  MsgList=Radar_RawTarget_Data_096  MsgName=Radar_RawTarget_Data_096  MsgIDType=Standard (11-bit identifier)  MsgIdentifier=1120  MsgLength=8  SignalInfo={ 'AZ_Winkel', '22', '10', 'LE', 'unsigned', 'Multiplexed', '0', '0.16', '-81.76', '-81.76', '81.92'; 'EL_Angle', '37', '10', 'LE', 'unsigned', 'Multiplexed', '1', '0.04', '-20.44', '-20.44', '20.48'; 'Internal_used', '14', '8', 'LE', 'unsigned', 'Multiplexed', '0', '1', '0', '-Inf', 'Inf'; 'Internal_used2', '32', '7', 'LE', 'unsigned', 'Multiplexed', '0', '1', '0', '-Inf', 'Inf'; 'Internal_used3', '51', '7', 'LE', 'unsigned', 'Multiplexed', '0', '1', '0', '-Inf', 'Inf'; 'Internal_used4', '58', '6', 'LE', 'unsigned', 'Multiplexed', '0', '1', '0', '-Inf', 'Inf'; 'Internal_used5', '9', '8', 'LE', 'unsigned', 'Multiplexed', '1', '1', '0', '-Inf', 'Inf'; 'Internal_used6', '17', '8', 'LE', 'unsigned', 'Multiplexed', '1', '1', '0', '-Inf', 'Inf'; 'Internal_used7', '25', '7', 'LE', 'unsigned', 'Multiplexed', '1', '1', '0', '-Inf', 'Inf'; 'Mode_Signal', '0', '1', 'LE', 'unsigned', 'Multiplexor', '0', '1', '0', '0', '1'; 'RCS', '1', '7', 'LE', 'unsigned', 'Multiplexed', '1', '0.2', '-15', '-15', '36'; 'Range1', '1', '13', 'LE', 'unsigned', 'Multiplexed', '0', '0.04', '0', '0', '327.64'; 'Reserve_3', '32', '5', 'LE', 'unsigned', 'Multiplexed', '1', '1', '0', '-Inf', 'Inf'; 'Reserve_4', '47', '16', 'LE', 'unsigned', 'Multiplexed', '1', '1', '0', '-Inf', 'Inf'; 'Speed_Radial', '39', '12', 'LE', 'unsigned', 'Multiplexed', '0', '0.04', '-119.68', '-44.12', '119.68' }  IDPort=on  TimestampPort=on  ErrorPort=off  RemotePort=off  LengthPort=off  StatusPort=off  ApplyMinMax=off
      settings: SourceProductBaseCode=ME,XP,VN  DataFormat=CANdb specified signals
  CAN Unpack98 : canmsglib/CAN Unpack  CANdbFile=eWolf_SensorCAN.dbc  MsgList=Radar_RawTarget_Data_097  MsgName=Radar_RawTarget_Data_097  MsgIDType=Standard (11-bit identifier)  MsgIdentifier=1121  MsgLength=8  SignalInfo={ 'AZ_Winkel', '22', '10', 'LE', 'unsigned', 'Multiplexed', '0', '0.16', '-81.76', '-81.76', '81.92'; 'EL_Angle', '37', '10', 'LE', 'unsigned', 'Multiplexed', '1', '0.04', '-20.44', '-20.44', '20.48'; 'Internal_used', '14', '8', 'LE', 'unsigned', 'Multiplexed', '0', '1', '0', '-Inf', 'Inf'; 'Internal_used2', '32', '7', 'LE', 'unsigned', 'Multiplexed', '0', '1', '0', '-Inf', 'Inf'; 'Internal_used3', '51', '7', 'LE', 'unsigned', 'Multiplexed', '0', '1', '0', '-Inf', 'Inf'; 'Internal_used4', '58', '6', 'LE', 'unsigned', 'Multiplexed', '0', '1', '0', '-Inf', 'Inf'; 'Internal_used5', '9', '8', 'LE', 'unsigned', 'Multiplexed', '1', '1', '0', '-Inf', 'Inf'; 'Internal_used6', '17', '8', 'LE', 'unsigned', 'Multiplexed', '1', '1', '0', '-Inf', 'Inf'; 'Internal_used7', '25', '7', 'LE', 'unsigned', 'Multiplexed', '1', '1', '0', '-Inf', 'Inf'; 'Mode_Signal', '0', '1', 'LE', 'unsigned', 'Multiplexor', '0', '1', '0', '0', '1'; 'RCS', '1', '7', 'LE', 'unsigned', 'Multiplexed', '1', '0.2', '-15', '-15', '36'; 'Range1', '1', '13', 'LE', 'unsigned', 'Multiplexed', '0', '0.04', '0', '0', '327.64'; 'Reserve_3', '32', '5', 'LE', 'unsigned', 'Multiplexed', '1', '1', '0', '-Inf', 'Inf'; 'Reserve_4', '47', '16', 'LE', 'unsigned', 'Multiplexed', '1', '1', '0', '-Inf', 'Inf'; 'Speed_Radial', '39', '12', 'LE', 'unsigned', 'Multiplexed', '0', '0.04', '-119.68', '-44.12', '119.68' }  IDPort=on  TimestampPort=on  ErrorPort=off  RemotePort=off  LengthPort=off  StatusPort=off  ApplyMinMax=off
      settings: SourceProductBaseCode=ME,XP,VN  DataFormat=CANdb specified signals
  CAN Unpack99 : canmsglib/CAN Unpack  CANdbFile=eWolf_SensorCAN.dbc  MsgList=Radar_RawTarget_Data_098  MsgName=Radar_RawTarget_Data_098  MsgIDType=Standard (11-bit identifier)  MsgIdentifier=1122  MsgLength=8  SignalInfo={ 'AZ_Winkel', '22', '10', 'LE', 'unsigned', 'Multiplexed', '0', '0.16', '-81.76', '-81.76', '81.92'; 'EL_Angle', '37', '10', 'LE', 'unsigned', 'Multiplexed', '1', '0.04', '-20.44', '-20.44', '20.48'; 'Internal_used', '14', '8', 'LE', 'unsigned', 'Multiplexed', '0', '1', '0', '-Inf', 'Inf'; 'Internal_used2', '32', '7', 'LE', 'unsigned', 'Multiplexed', '0', '1', '0', '-Inf', 'Inf'; 'Internal_used3', '51', '7', 'LE', 'unsigned', 'Multiplexed', '0', '1', '0', '-Inf', 'Inf'; 'Internal_used4', '58', '6', 'LE', 'unsigned', 'Multiplexed', '0', '1', '0', '-Inf', 'Inf'; 'Internal_used5', '9', '8', 'LE', 'unsigned', 'Multiplexed', '1', '1', '0', '-Inf', 'Inf'; 'Internal_used6', '17', '8', 'LE', 'unsigned', 'Multiplexed', '1', '1', '0', '-Inf', 'Inf'; 'Internal_used7', '25', '7', 'LE', 'unsigned', 'Multiplexed', '1', '1', '0', '-Inf', 'Inf'; 'Mode_Signal', '0', '1', 'LE', 'unsigned', 'Multiplexor', '0', '1', '0', '0', '1'; 'RCS', '1', '7', 'LE', 'unsigned', 'Multiplexed', '1', '0.2', '-15', '-15', '36'; 'Range1', '1', '13', 'LE', 'unsigned', 'Multiplexed', '0', '0.04', '0', '0', '327.64'; 'Reserve_3', '32', '5', 'LE', 'unsigned', 'Multiplexed', '1', '1', '0', '-Inf', 'Inf'; 'Reserve_4', '47', '16', 'LE', 'unsigned', 'Multiplexed', '1', '1', '0', '-Inf', 'Inf'; 'Speed_Radial', '39', '12', 'LE', 'unsigned', 'Multiplexed', '0', '0.04', '-119.68', '-44.12', '119.68' }  IDPort=on  TimestampPort=on  ErrorPort=off  RemotePort=off  LengthPort=off  StatusPort=off  ApplyMinMax=off
      settings: SourceProductBaseCode=ME,XP,VN  DataFormat=CANdb specified signals
  Terminator{1..1154} (1154 alike) : Terminator
  Radar Out : Outport
  wires:
  CAN Unpack3/13 -> Terminator20/1
  CAN Unpack3/15 -> Bus Creator3/6  "Speed_Radial"
  CAN Unpack3/6 -> Terminator16/1
  CAN Unpack3/7 -> Terminator17/1
  CAN Unpack3/1 -> Bus Creator3/1  "AZ_Winkel"
  CAN Unpack3/2 -> Bus Creator3/2  "EL_Angle"
  CAN Unpack3/3 -> Terminator13/1
  CAN Unpack3/12 -> Bus Creator3/5  "Range"
  CAN Unpack3/11 -> Bus Creator3/4  "RCS"
  CAN Unpack3/5 -> Terminator15/1
  CAN Unpack3/8 -> Terminator18/1
  CAN Unpack3/9 -> Terminator19/1
  CAN Unpack3/14 -> Terminator21/1
  CAN Unpack3/4 -> Terminator14/1
  CAN Unpack3/10 -> Bus Creator3/3  "Mode_Signal"
  CAN Msg/1 -> CAN Unpack1/1, CAN Unpack8/1, CAN Unpack44/1, CAN Unpack77/1, CAN Unpack106/1, CAN Unpack129/1, CAN Unpack128/1, CAN Unpack127/1, CAN Unpack126/1, CAN Unpack125/1, CAN Unpack124/1, CAN Unpack123/1, CAN Unpack122/1, CAN Unpack121/1, CAN Unpack120/1, CAN Unpack119/1, CAN Unpack118/1, CAN Unpack117/1, CAN Unpack116/1, CAN Unpack115/1, CAN Unpack114/1, CAN Unpack113/1, CAN Unpack112/1, CAN Unpack111/1, CAN Unpack110/1, CAN Unpack109/1, CAN Unpack108/1, CAN Unpack107/1, CAN Unpack105/1, CAN Unpack104/1, CAN Unpack103/1, CAN Unpack102/1, CAN Unpack101/1, CAN Unpack100/1, CAN Unpack99/1, CAN Unpack98/1, CAN Unpack97/1, CAN Unpack96/1, CAN Unpack95/1, CAN Unpack94/1, CAN Unpack93/1, CAN Unpack92/1, CAN Unpack91/1, CAN Unpack90/1, CAN Unpack89/1, CAN Unpack88/1, CAN Unpack87/1, CAN Unpack86/1, CAN Unpack85/1, CAN Unpack84/1, CAN Unpack83/1, CAN Unpack82/1, CAN Unpack81/1, CAN Unpack80/1, CAN Unpack79/1, CAN Unpack78/1, CAN Unpack76/1, CAN Unpack75/1, CAN Unpack74/1, CAN Unpack73/1, CAN Unpack72/1, CAN Unpack71/1, CAN Unpack70/1, CAN Unpack69/1, CAN Unpack68/1, CAN Unpack67/1, CAN Unpack66/1, CAN Unpack65/1, CAN Unpack64/1, CAN Unpack63/1, CAN Unpack62/1, CAN Unpack61/1, CAN Unpack60/1, CAN Unpack59/1, CAN Unpack58/1, CAN Unpack57/1, CAN Unpack56/1, CAN Unpack55/1, CAN Unpack54/1, CAN Unpack53/1, CAN Unpack52/1, CAN Unpack51/1, CAN Unpack50/1, CAN Unpack49/1, CAN Unpack48/1, CAN Unpack47/1, CAN Unpack46/1, CAN Unpack45/1, CAN Unpack43/1, CAN Unpack42/1, CAN Unpack41/1, CAN Unpack40/1, CAN Unpack39/1, CAN Unpack38/1, CAN Unpack37/1, CAN Unpack36/1, CAN Unpack35/1, CAN Unpack34/1, CAN Unpack33/1, CAN Unpack32/1, CAN Unpack31/1, CAN Unpack30/1, CAN Unpack29/1, CAN Unpack28/1, CAN Unpack27/1, CAN Unpack26/1, CAN Unpack25/1, CAN Unpack24/1, CAN Unpack23/1, CAN Unpack22/1, CAN Unpack21/1, CAN Unpack20/1, CAN Unpack19/1, CAN Unpack18/1, CAN Unpack17/1, CAN Unpack16/1, CAN Unpack15/1, CAN Unpack14/1, CAN Unpack13/1, CAN Unpack12/1, CAN Unpack11/1, CAN Unpack10/1, CAN Unpack9/1, CAN Unpack7/1, CAN Unpack6/1, CAN Unpack5/1, CAN Unpack4/1, CAN Unpack2/1, CAN Unpack3/1
  Bus Creator3/1 -> Bus Creator1/2  "Data_001"
  CAN Unpack3/16 -> Bus Creator3/7  "CAN ID"
  CAN Unpack3/17 -> Bus Creator3/8  "Timestamp"
  CAN Unpack1/1 -> Bus Creator/1  "Cycle_Duration"
  CAN Unpack1/2 -> Bus Creator/2  "Cycle_counter"
  CAN Unpack1/3 -> Bus Creator/3  "Number_of_Objects"
  CAN Unpack1/4 -> Terminator1/1
  CAN Unpack1/6 -> Bus Creator/4  "CAN ID"
  CAN Unpack1/7 -> Bus Creator/5  "Timestamp"
  CAN Unpack1/5 -> Terminator2/1
  Bus Creator/1 -> Bus Creator1/1  "Radar_Header"
  Bus Creator1/1 -> Radar Out/1
  Bus Creator2/1 -> Bus Creator1/3  "Data_002"
  CAN Unpack2/16 -> Bus Creator2/7  "CAN ID"
  CAN Unpack2/17 -> Bus Creator2/8  "Timestamp"
  CAN Unpack2/10 -> Bus Creator2/3  "Mode_Signal"
  CAN Unpack2/14 -> Terminator11/1
  CAN Unpack2/12 -> Bus Creator2/5  "Range"
  CAN Unpack2/9 -> Terminator9/1
  CAN Unpack2/5 -> Terminator5/1
  CAN Unpack2/8 -> Terminator8/1
  CAN Unpack2/4 -> Terminator4/1
  CAN Unpack2/7 -> Terminator7/1
  CAN Unpack2/11 -> Bus Creator2/4  "RCS"
  CAN Unpack2/2 -> Bus Creator2/2  "EL_Angle"
  CAN Unpack2/15 -> Bus Creator2/6  "Speed_Radial"
  CAN Unpack2/1 -> Bus Creator2/1  "AZ_Winkel"
  CAN Unpack2/6 -> Terminator6/1
  CAN Unpack2/3 -> Terminator3/1
  CAN Unpack2/13 -> Terminator10/1
  Bus Creator4/1 -> Bus Creator1/4  "Data_003"
  CAN Unpack4/16 -> Bus Creator4/7  "CAN ID"
  CAN Unpack4/17 -> Bus Creator4/8  "Timestamp"
  CAN Unpack4/10 -> Bus Creator4/3  "Mode_Signal"
  CAN Unpack4/14 -> Terminator29/1
  CAN Unpack4/12 -> Bus Creator4/5  "Range"
  CAN Unpack4/9 -> Terminator27/1
  CAN Unpack4/5 -> Terminator23/1
  CAN Unpack4/8 -> Terminator26/1
  CAN Unpack4/4 -> Terminator22/1
  CAN Unpack4/7 -> Terminator25/1
  CAN Unpack4/11 -> Bus Creator4/4  "RCS"
  CAN Unpack4/2 -> Bus Creator4/2  "EL_Angle"
  CAN Unpack4/15 -> Bus Creator4/6  "Speed_Radial"
  CAN Unpack4/1 -> Bus Creator4/1  "AZ_Winkel"
  CAN Unpack4/6 -> Terminator24/1
  CAN Unpack4/3 -> Terminator12/1
  CAN Unpack4/13 -> Terminator28/1
  Bus Creator5/1 -> Bus Creator1/5  "Data_004"
  CAN Unpack5/16 -> Bus Creator5/7  "CAN ID"
  CAN Unpack5/17 -> Bus Creator5/8  "Timestamp"
  CAN Unpack5/10 -> Bus Creator5/3  "Mode_Signal"
  CAN Unpack5/14 -> Terminator38/1
  CAN Unpack5/12 -> Bus Creator5/5  "Range"
  CAN Unpack5/9 -> Terminator36/1
  CAN Unpack5/5 -> Terminator32/1
  CAN Unpack5/8 -> Terminator35/1
  CAN Unpack5/4 -> Terminator31/1
  CAN Unpack5/7 -> Terminator34/1
  CAN Unpack5/11 -> Bus Creator5/4  "RCS"
  CAN Unpack5/2 -> Bus Creator5/2  "EL_Angle"
  CAN Unpack5/15 -> Bus Creator5/6  "Speed_Radial"
  CAN Unpack5/1 -> Bus Creator5/1  "AZ_Winkel"
  CAN Unpack5/6 -> Terminator33/1
  CAN Unpack5/3 -> Terminator30/1
  CAN Unpack5/13 -> Terminator37/1
  Bus Creator6/1 -> Bus Creator1/6  "Data_005"
  CAN Unpack6/16 -> Bus Creator6/7  "CAN ID"
  CAN Unpack6/17 -> Bus Creator6/8  "Timestamp"
  CAN Unpack6/10 -> Bus Creator6/3  "Mode_Signal"
  CAN Unpack6/14 -> Terminator47/1
  CAN Unpack6/12 -> Bus Creator6/5  "Range"
  CAN Unpack6/9 -> Terminator45/1
  CAN Unpack6/5 -> Terminator41/1
  CAN Unpack6/8 -> Terminator44/1
  CAN Unpack6/4 -> Terminator40/1
  CAN Unpack6/7 -> Terminator43/1
  CAN Unpack6/11 -> Bus Creator6/4  "RCS"
  CAN Unpack6/2 -> Bus Creator6/2  "EL_Angle"
  CAN Unpack6/15 -> Bus Creator6/6  "Speed_Radial"
  CAN Unpack6/1 -> Bus Creator6/1  "AZ_Winkel"
  CAN Unpack6/6 -> Terminator42/1
  CAN Unpack6/3 -> Terminator39/1
  CAN Unpack6/13 -> Terminator46/1
  Bus Creator7/1 -> Bus Creator1/7  "Data_006"
  CAN Unpack7/16 -> Bus Creator7/7  "CAN ID"
  CAN Unpack7/17 -> Bus Creator7/8  "Timestamp"
  CAN Unpack7/10 -> Bus Creator7/3  "Mode_Signal"
  CAN Unpack7/14 -> Terminator56/1
  CAN Unpack7/12 -> Bus Creator7/5  "Range"
  CAN Unpack7/9 -> Terminator54/1
  CAN Unpack7/5 -> Terminator50/1
  CAN Unpack7/8 -> Terminator53/1
  CAN Unpack7/4 -> Terminator49/1
  CAN Unpack7/7 -> Terminator52/1
  CAN Unpack7/11 -> Bus Creator7/4  "RCS"
  CAN Unpack7/2 -> Bus Creator7/2  "EL_Angle"
  CAN Unpack7/15 -> Bus Creator7/6  "Speed_Radial"
  CAN Unpack7/1 -> Bus Creator7/1  "AZ_Winkel"
  CAN Unpack7/6 -> Terminator51/1
  CAN Unpack7/3 -> Terminator48/1
  CAN Unpack7/13 -> Terminator55/1
  Bus Creator8/1 -> Bus Creator1/8  "Data_007"
  CAN Unpack8/16 -> Bus Creator8/7  "CAN ID"
  CAN Unpack8/17 -> Bus Creator8/8  "Timestamp"
  CAN Unpack8/10 -> Bus Creator8/3  "Mode_Signal"
  CAN Unpack8/14 -> Terminator65/1
  CAN Unpack8/12 -> Bus Creator8/5  "Range"
  CAN Unpack8/9 -> Terminator63/1
  CAN Unpack8/5 -> Terminator59/1
  CAN Unpack8/8 -> Terminator62/1
  CAN Unpack8/4 -> Terminator58/1
  CAN Unpack8/7 -> Terminator61/1
  CAN Unpack8/11 -> Bus Creator8/4  "RCS"
  CAN Unpack8/2 -> Bus Creator8/2  "EL_Angle"
  CAN Unpack8/15 -> Bus Creator8/6  "Speed_Radial"
  CAN Unpack8/1 -> Bus Creator8/1  "AZ_Winkel"
  CAN Unpack8/6 -> Terminator60/1
  CAN Unpack8/3 -> Terminator57/1
  CAN Unpack8/13 -> Terminator64/1
  Bus Creator9/1 -> Bus Creator1/9  "Data_008"
  CAN Unpack9/16 -> Bus Creator9/7  "CAN ID"
  CAN Unpack9/17 -> Bus Creator9/8  "Timestamp"
  CAN Unpack9/10 -> Bus Creator9/3  "Mode_Signal"
  CAN Unpack9/14 -> Terminator74/1
  CAN Unpack9/12 -> Bus Creator9/5  "Range"
  CAN Unpack9/9 -> Terminator72/1
  CAN Unpack9/5 -> Terminator68/1
  CAN Unpack9/8 -> Terminator71/1
  CAN Unpack9/4 -> Terminator67/1
  CAN Unpack9/7 -> Terminator70/1
  CAN Unpack9/11 -> Bus Creator9/4  "RCS"
  CAN Unpack9/2 -> Bus Creator9/2  "EL_Angle"
  CAN Unpack9/15 -> Bus Creator9/6  "Speed_Radial"
  CAN Unpack9/1 -> Bus Creator9/1  "AZ_Winkel"
  CAN Unpack9/6 -> Terminator69/1
  CAN Unpack9/3 -> Terminator66/1
  CAN Unpack9/13 -> Terminator73/1
  Bus Creator10/1 -> Bus Creator1/10  "Data_009"
  CAN Unpack10/16 -> Bus Creator10/7  "CAN ID"
  CAN Unpack10/17 -> Bus Creator10/8  "Timestamp"
  CAN Unpack10/10 -> Bus Creator10/3  "Mode_Signal"
  CAN Unpack10/14 -> Terminator83/1
  CAN Unpack10/12 -> Bus Creator10/5  "Range"
  CAN Unpack10/9 -> Terminator81/1
  CAN Unpack10/5 -> Terminator77/1
  CAN Unpack10/8 -> Terminator80/1
  CAN Unpack10/4 -> Terminator76/1
  CAN Unpack10/7 -> Terminator79/1
  CAN Unpack10/11 -> Bus Creator10/4  "RCS"
  CAN Unpack10/2 -> Bus Creator10/2  "EL_Angle"
  CAN Unpack10/15 -> Bus Creator10/6  "Speed_Radial"
  CAN Unpack10/1 -> Bus Creator10/1  "AZ_Winkel"
  CAN Unpack10/6 -> Terminator78/1
  CAN Unpack10/3 -> Terminator75/1
  CAN Unpack10/13 -> Terminator82/1
  Bus Creator11/1 -> Bus Creator1/11  "Data_010"
  CAN Unpack11/16 -> Bus Creator11/7  "CAN ID"
  CAN Unpack11/17 -> Bus Creator11/8  "Timestamp"
  CAN Unpack11/10 -> Bus Creator11/3  "Mode_Signal"
  CAN Unpack11/14 -> Terminator92/1
  CAN Unpack11/12 -> Bus Creator11/5  "Range"
  CAN Unpack11/9 -> Terminator90/1
  CAN Unpack11/5 -> Terminator86/1
  CAN Unpack11/8 -> Terminator89/1
  CAN Unpack11/4 -> Terminator85/1
  CAN Unpack11/7 -> Terminator88/1
  CAN Unpack11/11 -> Bus Creator11/4  "RCS"
  CAN Unpack11/2 -> Bus Creator11/2  "EL_Angle"
  CAN Unpack11/15 -> Bus Creator11/6  "Speed_Radial"
  CAN Unpack11/1 -> Bus Creator11/1  "AZ_Winkel"
  CAN Unpack11/6 -> Terminator87/1
  CAN Unpack11/3 -> Terminator84/1
  CAN Unpack11/13 -> Terminator91/1
  Bus Creator12/1 -> Bus Creator1/12  "Data_011"
  CAN Unpack12/16 -> Bus Creator12/7  "CAN ID"
  CAN Unpack12/17 -> Bus Creator12/8  "Timestamp"
  CAN Unpack12/10 -> Bus Creator12/3  "Mode_Signal"
  CAN Unpack12/14 -> Terminator101/1
  CAN Unpack12/12 -> Bus Creator12/5  "Range"
  CAN Unpack12/9 -> Terminator99/1
  CAN Unpack12/5 -> Terminator95/1
  CAN Unpack12/8 -> Terminator98/1
  CAN Unpack12/4 -> Terminator94/1
  CAN Unpack12/7 -> Terminator97/1
  CAN Unpack12/11 -> Bus Creator12/4  "RCS"
  CAN Unpack12/2 -> Bus Creator12/2  "EL_Angle"
  CAN Unpack12/15 -> Bus Creator12/6  "Speed_Radial"
  CAN Unpack12/1 -> Bus Creator12/1  "AZ_Winkel"
  CAN Unpack12/6 -> Terminator96/1
  CAN Unpack12/3 -> Terminator93/1
  CAN Unpack12/13 -> Terminator100/1
  Bus Creator13/1 -> Bus Creator1/13  "Data_012"
  CAN Unpack13/16 -> Bus Creator13/7  "CAN ID"
  CAN Unpack13/17 -> Bus Creator13/8  "Timestamp"
  CAN Unpack13/10 -> Bus Creator13/3  "Mode_Signal"
  CAN Unpack13/14 -> Terminator110/1
  CAN Unpack13/12 -> Bus Creator13/5  "Range"
  CAN Unpack13/9 -> Terminator108/1
  CAN Unpack13/5 -> Terminator104/1
  CAN Unpack13/8 -> Terminator107/1
  CAN Unpack13/4 -> Terminator103/1
  CAN Unpack13/7 -> Terminator106/1
  CAN Unpack13/11 -> Bus Creator13/4  "RCS"
  CAN Unpack13/2 -> Bus Creator13/2  "EL_Angle"
  CAN Unpack13/15 -> Bus Creator13/6  "Speed_Radial"
  CAN Unpack13/1 -> Bus Creator13/1  "AZ_Winkel"
  CAN Unpack13/6 -> Terminator105/1
  CAN Unpack13/3 -> Terminator102/1
  CAN Unpack13/13 -> Terminator109/1
  CAN Unpack14/16 -> Bus Creator14/7  "CAN ID"
  CAN Unpack14/17 -> Bus Creator14/8  "Timestamp"
  CAN Unpack14/10 -> Bus Creator14/3  "Mode_Signal"
  CAN Unpack14/14 -> Terminator119/1
  CAN Unpack14/12 -> Bus Creator14/5  "Range"
  CAN Unpack14/9 -> Terminator117/1
  CAN Unpack14/5 -> Terminator113/1
  CAN Unpack14/8 -> Terminator116/1
  CAN Unpack14/4 -> Terminator112/1
  CAN Unpack14/7 -> Terminator115/1
  CAN Unpack14/11 -> Bus Creator14/4  "RCS"
  CAN Unpack14/2 -> Bus Creator14/2  "EL_Angle"
  CAN Unpack14/15 -> Bus Creator14/6  "Speed_Radial"
  CAN Unpack14/1 -> Bus Creator14/1  "AZ_Winkel"
  CAN Unpack14/6 -> Terminator114/1
  CAN Unpack14/3 -> Terminator111/1
  CAN Unpack14/13 -> Terminator118/1
  Bus Creator14/1 -> Bus Creator1/14  "Data_013"
  CAN Unpack15/16 -> Bus Creator15/7  "CAN ID"
  CAN Unpack15/17 -> Bus Creator15/8  "Timestamp"
  CAN Unpack15/10 -> Bus Creator15/3  "Mode_Signal"
  CAN Unpack15/14 -> Terminator128/1
  CAN Unpack15/12 -> Bus Creator15/5  "Range"
  CAN Unpack15/9 -> Terminator126/1
  CAN Unpack15/5 -> Terminator122/1
  CAN Unpack15/8 -> Terminator125/1
  CAN Unpack15/4 -> Terminator121/1
  CAN Unpack15/7 -> Terminator124/1
  CAN Unpack15/11 -> Bus Creator15/4  "RCS"
  CAN Unpack15/2 -> Bus Creator15/2  "EL_Angle"
  CAN Unpack15/15 -> Bus Creator15/6  "Speed_Radial"
  CAN Unpack15/1 -> Bus Creator15/1  "AZ_Winkel"
  CAN Unpack15/6 -> Terminator123/1
  CAN Unpack15/3 -> Terminator120/1
  CAN Unpack15/13 -> Terminator127/1
  Bus Creator15/1 -> Bus Creator1/15  "Data_014"
  CAN Unpack16/16 -> Bus Creator16/7  "CAN ID"
  CAN Unpack16/17 -> Bus Creator16/8  "Timestamp"
  CAN Unpack16/10 -> Bus Creator16/3  "Mode_Signal"
  CAN Unpack16/14 -> Terminator137/1
  CAN Unpack16/12 -> Bus Creator16/5  "Range"
  CAN Unpack16/9 -> Terminator135/1
  CAN Unpack16/5 -> Terminator131/1
  CAN Unpack16/8 -> Terminator134/1
  CAN Unpack16/4 -> Terminator130/1
  CAN Unpack16/7 -> Terminator133/1
  CAN Unpack16/11 -> Bus Creator16/4  "RCS"
  CAN Unpack16/2 -> Bus Creator16/2  "EL_Angle"
  CAN Unpack16/15 -> Bus Creator16/6  "Speed_Radial"
  CAN Unpack16/1 -> Bus Creator16/1  "AZ_Winkel"
  CAN Unpack16/6 -> Terminator132/1
  CAN Unpack16/3 -> Terminator129/1
  CAN Unpack16/13 -> Terminator136/1
  Bus Creator16/1 -> Bus Creator1/16  "Data_015"
  CAN Unpack17/16 -> Bus Creator17/7  "CAN ID"
  CAN Unpack17/17 -> Bus Creator17/8  "Timestamp"
  CAN Unpack17/10 -> Bus Creator17/3  "Mode_Signal"
  CAN Unpack17/14 -> Terminator146/1
  CAN Unpack17/12 -> Bus Creator17/5  "Range"
  CAN Unpack17/9 -> Terminator144/1
  CAN Unpack17/5 -> Terminator140/1
  CAN Unpack17/8 -> Terminator143/1
  CAN Unpack17/4 -> Terminator139/1
  CAN Unpack17/7 -> Terminator142/1
  CAN Unpack17/11 -> Bus Creator17/4  "RCS"
  CAN Unpack17/2 -> Bus Creator17/2  "EL_Angle"
  CAN Unpack17/15 -> Bus Creator17/6  "Speed_Radial"
  CAN Unpack17/1 -> Bus Creator17/1  "AZ_Winkel"
  CAN Unpack17/6 -> Terminator141/1
  CAN Unpack17/3 -> Terminator138/1
  CAN Unpack17/13 -> Terminator145/1
  Bus Creator17/1 -> Bus Creator1/17  "Data_016"
  CAN Unpack18/16 -> Bus Creator18/7  "CAN ID"
  CAN Unpack18/17 -> Bus Creator18/8  "Timestamp"
  CAN Unpack18/10 -> Bus Creator18/3  "Mode_Signal"
  CAN Unpack18/14 -> Terminator155/1
  CAN Unpack18/12 -> Bus Creator18/5  "Range"
  CAN Unpack18/9 -> Terminator153/1
  CAN Unpack18/5 -> Terminator149/1
  CAN Unpack18/8 -> Terminator152/1
  CAN Unpack18/4 -> Terminator148/1
  CAN Unpack18/7 -> Terminator151/1
  CAN Unpack18/11 -> Bus Creator18/4  "RCS"
  CAN Unpack18/2 -> Bus Creator18/2  "EL_Angle"
  CAN Unpack18/15 -> Bus Creator18/6  "Speed_Radial"
  CAN Unpack18/1 -> Bus Creator18/1  "AZ_Winkel"
  CAN Unpack18/6 -> Terminator150/1
  CAN Unpack18/3 -> Terminator147/1
  CAN Unpack18/13 -> Terminator154/1
  Bus Creator18/1 -> Bus Creator1/18  "Data_017"
  CAN Unpack19/16 -> Bus Creator19/7  "CAN ID"
  CAN Unpack19/17 -> Bus Creator19/8  "Timestamp"
  CAN Unpack19/10 -> Bus Creator19/3  "Mode_Signal"
  CAN Unpack19/14 -> Terminator164/1
  CAN Unpack19/12 -> Bus Creator19/5  "Range"
  CAN Unpack19/9 -> Terminator162/1
  CAN Unpack19/5 -> Terminator158/1
  CAN Unpack19/8 -> Terminator161/1
  CAN Unpack19/4 -> Terminator157/1
  CAN Unpack19/7 -> Terminator160/1
  CAN Unpack19/11 -> Bus Creator19/4  "RCS"
  CAN Unpack19/2 -> Bus Creator19/2  "EL_Angle"
  CAN Unpack19/15 -> Bus Creator19/6  "Speed_Radial"
  CAN Unpack19/1 -> Bus Creator19/1  "AZ_Winkel"
  CAN Unpack19/6 -> Terminator159/1
  CAN Unpack19/3 -> Terminator156/1
  CAN Unpack19/13 -> Terminator163/1
  Bus Creator19/1 -> Bus Creator1/19  "Data_018"
  CAN Unpack20/16 -> Bus Creator20/7  "CAN ID"
  CAN Unpack20/17 -> Bus Creator20/8  "Timestamp"
  CAN Unpack20/10 -> Bus Creator20/3  "Mode_Signal"
  CAN Unpack20/14 -> Terminator173/1
  CAN Unpack20/12 -> Bus Creator20/5  "Range"
  CAN Unpack20/9 -> Terminator171/1
  CAN Unpack20/5 -> Terminator167/1
  CAN Unpack20/8 -> Terminator170/1
  CAN Unpack20/4 -> Terminator166/1
  CAN Unpack20/7 -> Terminator169/1
  CAN Unpack20/11 -> Bus Creator20/4  "RCS"
  CAN Unpack20/2 -> Bus Creator20/2  "EL_Angle"
  CAN Unpack20/15 -> Bus Creator20/6  "Speed_Radial"
  CAN Unpack20/1 -> Bus Creator20/1  "AZ_Winkel"
  CAN Unpack20/6 -> Terminator168/1
  CAN Unpack20/3 -> Terminator165/1
  CAN Unpack20/13 -> Terminator172/1
  Bus Creator20/1 -> Bus Creator1/20  "Data_019"
  CAN Unpack21/16 -> Bus Creator21/7  "CAN ID"
  CAN Unpack21/17 -> Bus Creator21/8  "Timestamp"
  CAN Unpack21/10 -> Bus Creator21/3  "Mode_Signal"
  CAN Unpack21/14 -> Terminator182/1
  CAN Unpack21/12 -> Bus Creator21/5  "Range"
  CAN Unpack21/9 -> Terminator180/1
  CAN Unpack21/5 -> Terminator176/1
  CAN Unpack21/8 -> Terminator179/1
  CAN Unpack21/4 -> Terminator175/1
  CAN Unpack21/7 -> Terminator178/1
  CAN Unpack21/11 -> Bus Creator21/4  "RCS"
  CAN Unpack21/2 -> Bus Creator21/2  "EL_Angle"
  CAN Unpack21/15 -> Bus Creator21/6  "Speed_Radial"
  CAN Unpack21/1 -> Bus Creator21/1  "AZ_Winkel"
  CAN Unpack21/6 -> Terminator177/1
  CAN Unpack21/3 -> Terminator174/1
  CAN Unpack21/13 -> Terminator181/1
  Bus Creator21/1 -> Bus Creator1/21  "Data_020"
  CAN Unpack22/16 -> Bus Creator22/7  "CAN ID"
  CAN Unpack22/17 -> Bus Creator22/8  "Timestamp"
  CAN Unpack22/10 -> Bus Creator22/3  "Mode_Signal"
  CAN Unpack22/14 -> Terminator191/1
  CAN Unpack22/12 -> Bus Creator22/5  "Range"
  CAN Unpack22/9 -> Terminator189/1
  CAN Unpack22/5 -> Terminator185/1
  CAN Unpack22/8 -> Terminator188/1
  CAN Unpack22/4 -> Terminator184/1
  CAN Unpack22/7 -> Terminator187/1
  CAN Unpack22/11 -> Bus Creator22/4  "RCS"
  CAN Unpack22/2 -> Bus Creator22/2  "EL_Angle"
  CAN Unpack22/15 -> Bus Creator22/6  "Speed_Radial"
  CAN Unpack22/1 -> Bus Creator22/1  "AZ_Winkel"
  CAN Unpack22/6 -> Terminator186/1
  CAN Unpack22/3 -> Terminator183/1
  CAN Unpack22/13 -> Terminator190/1
  Bus Creator22/1 -> Bus Creator1/22  "Data_021"
  CAN Unpack23/16 -> Bus Creator23/7  "CAN ID"
  CAN Unpack23/17 -> Bus Creator23/8  "Timestamp"
  CAN Unpack23/10 -> Bus Creator23/3  "Mode_Signal"
  CAN Unpack23/14 -> Terminator200/1
  CAN Unpack23/12 -> Bus Creator23/5  "Range"
  CAN Unpack23/9 -> Terminator198/1
  CAN Unpack23/5 -> Terminator194/1
  CAN Unpack23/8 -> Terminator197/1
  CAN Unpack23/4 -> Terminator193/1
  CAN Unpack23/7 -> Terminator196/1
  CAN Unpack23/11 -> Bus Creator23/4  "RCS"
  CAN Unpack23/2 -> Bus Creator23/2  "EL_Angle"
  CAN Unpack23/15 -> Bus Creator23/6  "Speed_Radial"
  CAN Unpack23/1 -> Bus Creator23/1  "AZ_Winkel"
  CAN Unpack23/6 -> Terminator195/1
  CAN Unpack23/3 -> Terminator192/1
  CAN Unpack23/13 -> Terminator199/1
  Bus Creator23/1 -> Bus Creator1/23  "Data_022"
  CAN Unpack24/16 -> Bus Creator24/7  "CAN ID"
  CAN Unpack24/17 -> Bus Creator24/8  "Timestamp"
  CAN Unpack24/10 -> Bus Creator24/3  "Mode_Signal"
  CAN Unpack24/14 -> Terminator209/1
  CAN Unpack24/12 -> Bus Creator24/5  "Range"
  CAN Unpack24/9 -> Terminator207/1
  CAN Unpack24/5 -> Terminator203/1
  CAN Unpack24/8 -> Terminator206/1
  CAN Unpack24/4 -> Terminator202/1
  CAN Unpack24/7 -> Terminator205/1
  CAN Unpack24/11 -> Bus Creator24/4  "RCS"
  CAN Unpack24/2 -> Bus Creator24/2  "EL_Angle"
  CAN Unpack24/15 -> Bus Creator24/6  "Speed_Radial"
  CAN Unpack24/1 -> Bus Creator24/1  "AZ_Winkel"
  CAN Unpack24/6 -> Terminator204/1
  CAN Unpack24/3 -> Terminator201/1
  CAN Unpack24/13 -> Terminator208/1
  Bus Creator24/1 -> Bus Creator1/24  "Data_023"
  CAN Unpack25/16 -> Bus Creator25/7  "CAN ID"
  CAN Unpack25/17 -> Bus Creator25/8  "Timestamp"
  CAN Unpack25/10 -> Bus Creator25/3  "Mode_Signal"
  CAN Unpack25/14 -> Terminator218/1
  CAN Unpack25/12 -> Bus Creator25/5  "Range"
  CAN Unpack25/9 -> Terminator216/1
  CAN Unpack25/5 -> Terminator212/1
  CAN Unpack25/8 -> Terminator215/1
  CAN Unpack25/4 -> Terminator211/1
  CAN Unpack25/7 -> Terminator214/1
  CAN Unpack25/11 -> Bus Creator25/4  "RCS"
  CAN Unpack25/2 -> Bus Creator25/2  "EL_Angle"
  CAN Unpack25/15 -> Bus Creator25/6  "Speed_Radial"
  CAN Unpack25/1 -> Bus Creator25/1  "AZ_Winkel"
  CAN Unpack25/6 -> Terminator213/1
  CAN Unpack25/3 -> Terminator210/1
  CAN Unpack25/13 -> Terminator217/1
  Bus Creator25/1 -> Bus Creator1/25  "Data_024"
  CAN Unpack26/16 -> Bus Creator26/7  "CAN ID"
  CAN Unpack26/17 -> Bus Creator26/8  "Timestamp"
  CAN Unpack26/10 -> Bus Creator26/3  "Mode_Signal"
  CAN Unpack26/14 -> Terminator227/1
  CAN Unpack26/12 -> Bus Creator26/5  "Range"
  CAN Unpack26/9 -> Terminator225/1
  CAN Unpack26/5 -> Terminator221/1
  CAN Unpack26/8 -> Terminator224/1
  CAN Unpack26/4 -> Terminator220/1
  CAN Unpack26/7 -> Terminator223/1
  CAN Unpack26/11 -> Bus Creator26/4  "RCS"
  CAN Unpack26/2 -> Bus Creator26/2  "EL_Angle"
  CAN Unpack26/15 -> Bus Creator26/6  "Speed_Radial"
  CAN Unpack26/1 -> Bus Creator26/1  "AZ_Winkel"
  CAN Unpack26/6 -> Terminator222/1
  CAN Unpack26/3 -> Terminator219/1
  CAN Unpack26/13 -> Terminator226/1
  Bus Creator26/1 -> Bus Creator1/26  "Data_025"
  CAN Unpack27/16 -> Bus Creator27/7  "CAN ID"
  CAN Unpack27/17 -> Bus Creator27/8  "Timestamp"
  CAN Unpack27/10 -> Bus Creator27/3  "Mode_Signal"
  CAN Unpack27/14 -> Terminator236/1
  CAN Unpack27/12 -> Bus Creator27/5  "Range"
  CAN Unpack27/9 -> Terminator234/1
  CAN Unpack27/5 -> Terminator230/1
  CAN Unpack27/8 -> Terminator233/1
  CAN Unpack27/4 -> Terminator229/1
  CAN Unpack27/7 -> Terminator232/1
  CAN Unpack27/11 -> Bus Creator27/4  "RCS"
  CAN Unpack27/2 -> Bus Creator27/2  "EL_Angle"
  CAN Unpack27/15 -> Bus Creator27/6  "Speed_Radial"
  CAN Unpack27/1 -> Bus Creator27/1  "AZ_Winkel"
  CAN Unpack27/6 -> Terminator231/1
  CAN Unpack27/3 -> Terminator228/1
  CAN Unpack27/13 -> Terminator235/1
  Bus Creator27/1 -> Bus Creator1/27  "Data_026"
  CAN Unpack28/16 -> Bus Creator28/7  "CAN ID"
  CAN Unpack28/17 -> Bus Creator28/8  "Timestamp"
  CAN Unpack28/10 -> Bus Creator28/3  "Mode_Signal"
  CAN Unpack28/14 -> Terminator245/1
  CAN Unpack28/12 -> Bus Creator28/5  "Range"
  CAN Unpack28/9 -> Terminator243/1
  CAN Unpack28/5 -> Terminator239/1
  CAN Unpack28/8 -> Terminator242/1
  CAN Unpack28/4 -> Terminator238/1
  CAN Unpack28/7 -> Terminator241/1
  CAN Unpack28/11 -> Bus Creator28/4  "RCS"
  CAN Unpack28/2 -> Bus Creator28/2  "EL_Angle"
  CAN Unpack28/15 -> Bus Creator28/6  "Speed_Radial"
  CAN Unpack28/1 -> Bus Creator28/1  "AZ_Winkel"
  CAN Unpack28/6 -> Terminator240/1
  CAN Unpack28/3 -> Terminator237/1
  CAN Unpack28/13 -> Terminator244/1
  Bus Creator28/1 -> Bus Creator1/28  "Data_027"
  CAN Unpack29/16 -> Bus Creator29/7  "CAN ID"
  CAN Unpack29/17 -> Bus Creator29/8  "Timestamp"
  CAN Unpack29/10 -> Bus Creator29/3  "Mode_Signal"
  CAN Unpack29/14 -> Terminator254/1
  CAN Unpack29/12 -> Bus Creator29/5  "Range"
  CAN Unpack29/9 -> Terminator252/1
  CAN Unpack29/5 -> Terminator248/1
  CAN Unpack29/8 -> Terminator251/1
  CAN Unpack29/4 -> Terminator247/1
  CAN Unpack29/7 -> Terminator250/1
  CAN Unpack29/11 -> Bus Creator29/4  "RCS"
  CAN Unpack29/2 -> Bus Creator29/2  "EL_Angle"
  CAN Unpack29/15 -> Bus Creator29/6  "Speed_Radial"
  CAN Unpack29/1 -> Bus Creator29/1  "AZ_Winkel"
  CAN Unpack29/6 -> Terminator249/1
  CAN Unpack29/3 -> Terminator246/1
  CAN Unpack29/13 -> Terminator253/1
  Bus Creator29/1 -> Bus Creator1/29  "Data_028"
  CAN Unpack30/4 -> Terminator256/1
  CAN Unpack30/2 -> Bus Creator30/2  "EL_Angle"
  CAN Unpack30/13 -> Terminator262/1
  CAN Unpack30/5 -> Terminator257/1
  CAN Unpack30/7 -> Terminator259/1
  CAN Unpack30/3 -> Terminator255/1
  CAN Unpack30/8 -> Terminator260/1
  CAN Unpack30/1 -> Bus Creator30/1  "AZ_Winkel"
  CAN Unpack30/6 -> Terminator258/1
  CAN Unpack30/10 -> Bus Creator30/3  "Mode_Signal"
  CAN Unpack30/15 -> Bus Creator30/6  "Speed_Radial"
  CAN Unpack30/14 -> Terminator263/1
  CAN Unpack30/12 -> Bus Creator30/5  "Range"
  CAN Unpack30/11 -> Bus Creator30/4  "RCS"
  CAN Unpack30/16 -> Bus Creator30/7  "CAN ID"
  CAN Unpack30/17 -> Bus Creator30/8  "Timestamp"
  CAN Unpack30/9 -> Terminator261/1
  Bus Creator30/1 -> Bus Creator1/30  "Data_029"
  CAN Unpack31/4 -> Terminator265/1
  CAN Unpack31/2 -> Bus Creator31/2  "EL_Angle"
  CAN Unpack31/13 -> Terminator271/1
  CAN Unpack31/5 -> Terminator266/1
  CAN Unpack31/7 -> Terminator268/1
  CAN Unpack31/3 -> Terminator264/1
  CAN Unpack31/8 -> Terminator269/1
  CAN Unpack31/1 -> Bus Creator31/1  "AZ_Winkel"
  CAN Unpack31/6 -> Terminator267/1
  CAN Unpack31/10 -> Bus Creator31/3  "Mode_Signal"
  CAN Unpack31/15 -> Bus Creator31/6  "Speed_Radial"
  CAN Unpack31/14 -> Terminator272/1
  CAN Unpack31/12 -> Bus Creator31/5  "Range"
  CAN Unpack31/11 -> Bus Creator31/4  "RCS"
  CAN Unpack31/16 -> Bus Creator31/7  "CAN ID"
  CAN Unpack31/17 -> Bus Creator31/8  "Timestamp"
  CAN Unpack31/9 -> Terminator270/1
  Bus Creator31/1 -> Bus Creator1/31  "Data_030"
  CAN Unpack32/4 -> Terminator274/1
  CAN Unpack32/2 -> Bus Creator32/2  "EL_Angle"
  CAN Unpack32/13 -> Terminator280/1
  CAN Unpack32/5 -> Terminator275/1
  CAN Unpack32/7 -> Terminator277/1
  CAN Unpack32/3 -> Terminator273/1
  CAN Unpack32/8 -> Terminator278/1
  CAN Unpack32/1 -> Bus Creator32/1  "AZ_Winkel"
  CAN Unpack32/6 -> Terminator276/1
  CAN Unpack32/10 -> Bus Creator32/3  "Mode_Signal"
  CAN Unpack32/15 -> Bus Creator32/6  "Speed_Radial"
  CAN Unpack32/14 -> Terminator281/1
  CAN Unpack32/12 -> Bus Creator32/5  "Range"
  CAN Unpack32/11 -> Bus Creator32/4  "RCS"
  CAN Unpack32/16 -> Bus Creator32/7  "CAN ID"
  CAN Unpack32/17 -> Bus Creator32/8  "Timestamp"
  CAN Unpack32/9 -> Terminator279/1
  Bus Creator32/1 -> Bus Creator1/32  "Data_031"
  CAN Unpack33/4 -> Terminator283/1
  CAN Unpack33/2 -> Bus Creator33/2  "EL_Angle"
  CAN Unpack33/13 -> Terminator289/1
  CAN Unpack33/5 -> Terminator284/1
  CAN Unpack33/7 -> Terminator286/1
  CAN Unpack33/3 -> Terminator282/1
  CAN Unpack33/8 -> Terminator287/1
  CAN Unpack33/1 -> Bus Creator33/1  "AZ_Winkel"
  CAN Unpack33/6 -> Terminator285/1
  CAN Unpack33/10 -> Bus Creator33/3  "Mode_Signal"
  CAN Unpack33/15 -> Bus Creator33/6  "Speed_Radial"
  CAN Unpack33/14 -> Terminator290/1
  CAN Unpack33/12 -> Bus Creator33/5  "Range"
  CAN Unpack33/11 -> Bus Creator33/4  "RCS"
  CAN Unpack33/16 -> Bus Creator33/7  "CAN ID"
  CAN Unpack33/17 -> Bus Creator33/8  "Timestamp"
  CAN Unpack33/9 -> Terminator288/1
  Bus Creator33/1 -> Bus Creator1/33  "Data_032"
  CAN Unpack34/4 -> Terminator292/1
  CAN Unpack34/2 -> Bus Creator34/2  "EL_Angle"
  CAN Unpack34/13 -> Terminator298/1
  CAN Unpack34/5 -> Terminator293/1
  CAN Unpack34/7 -> Terminator295/1
  CAN Unpack34/3 -> Terminator291/1
  CAN Unpack34/8 -> Terminator296/1
  CAN Unpack34/1 -> Bus Creator34/1  "AZ_Winkel"
  CAN Unpack34/6 -> Terminator294/1
  CAN Unpack34/10 -> Bus Creator34/3  "Mode_Signal"
  CAN Unpack34/15 -> Bus Creator34/6  "Speed_Radial"
  CAN Unpack34/14 -> Terminator299/1
  CAN Unpack34/12 -> Bus Creator34/5  "Range"
  CAN Unpack34/11 -> Bus Creator34/4  "RCS"
  CAN Unpack34/16 -> Bus Creator34/7  "CAN ID"
  CAN Unpack34/17 -> Bus Creator34/8  "Timestamp"
  CAN Unpack34/9 -> Terminator297/1
  Bus Creator34/1 -> Bus Creator1/34  "Data_033"
  CAN Unpack35/4 -> Terminator301/1
  CAN Unpack35/2 -> Bus Creator35/2  "EL_Angle"
  CAN Unpack35/13 -> Terminator307/1
  CAN Unpack35/5 -> Terminator302/1
  CAN Unpack35/7 -> Terminator304/1
  CAN Unpack35/3 -> Terminator300/1
  CAN Unpack35/8 -> Terminator305/1
  CAN Unpack35/1 -> Bus Creator35/1  "AZ_Winkel"
  CAN Unpack35/6 -> Terminator303/1
  CAN Unpack35/10 -> Bus Creator35/3  "Mode_Signal"
  CAN Unpack35/15 -> Bus Creator35/6  "Speed_Radial"
  CAN Unpack35/14 -> Terminator308/1
  CAN Unpack35/12 -> Bus Creator35/5  "Range"
  CAN Unpack35/11 -> Bus Creator35/4  "RCS"
  CAN Unpack35/16 -> Bus Creator35/7  "CAN ID"
  CAN Unpack35/17 -> Bus Creator35/8  "Timestamp"
  CAN Unpack35/9 -> Terminator306/1
  Bus Creator35/1 -> Bus Creator1/35  "Data_034"
  CAN Unpack36/4 -> Terminator310/1
  CAN Unpack36/2 -> Bus Creator36/2  "EL_Angle"
  CAN Unpack36/13 -> Terminator316/1
  CAN Unpack36/5 -> Terminator311/1
  CAN Unpack36/7 -> Terminator313/1
  CAN Unpack36/3 -> Terminator309/1
  CAN Unpack36/8 -> Terminator314/1
  CAN Unpack36/1 -> Bus Creator36/1  "AZ_Winkel"
  CAN Unpack36/6 -> Terminator312/1
  CAN Unpack36/10 -> Bus Creator36/3  "Mode_Signal"
  CAN Unpack36/15 -> Bus Creator36/6  "Speed_Radial"
  CAN Unpack36/14 -> Terminator317/1
  CAN Unpack36/12 -> Bus Creator36/5  "Range"
  CAN Unpack36/11 -> Bus Creator36/4  "RCS"
  CAN Unpack36/16 -> Bus Creator36/7  "CAN ID"
  CAN Unpack36/17 -> Bus Creator36/8  "Timestamp"
  CAN Unpack36/9 -> Terminator315/1
  Bus Creator36/1 -> Bus Creator1/36  "Data_035"
  CAN Unpack37/4 -> Terminator319/1
  CAN Unpack37/2 -> Bus Creator37/2  "EL_Angle"
  CAN Unpack37/13 -> Terminator325/1
  CAN Unpack37/5 -> Terminator320/1
  CAN Unpack37/7 -> Terminator322/1
  CAN Unpack37/3 -> Terminator318/1
  CAN Unpack37/8 -> Terminator323/1
  CAN Unpack37/1 -> Bus Creator37/1  "AZ_Winkel"
  CAN Unpack37/6 -> Terminator321/1
  CAN Unpack37/10 -> Bus Creator37/3  "Mode_Signal"
  CAN Unpack37/15 -> Bus Creator37/6  "Speed_Radial"
  CAN Unpack37/14 -> Terminator326/1
  CAN Unpack37/12 -> Bus Creator37/5  "Range"
  CAN Unpack37/11 -> Bus Creator37/4  "RCS"
  CAN Unpack37/16 -> Bus Creator37/7  "CAN ID"
  CAN Unpack37/17 -> Bus Creator37/8  "Timestamp"
  CAN Unpack37/9 -> Terminator324/1
  Bus Creator37/1 -> Bus Creator1/37  "Data_036"
  CAN Unpack38/4 -> Terminator328/1
  CAN Unpack38/2 -> Bus Creator38/2  "EL_Angle"
  CAN Unpack38/13 -> Terminator334/1
  CAN Unpack38/5 -> Terminator329/1
  CAN Unpack38/7 -> Terminator331/1
  CAN Unpack38/3 -> Terminator327/1
  CAN Unpack38/8 -> Terminator332/1
  CAN Unpack38/1 -> Bus Creator38/1  "AZ_Winkel"
  CAN Unpack38/6 -> Terminator330/1
  CAN Unpack38/10 -> Bus Creator38/3  "Mode_Signal"
  CAN Unpack38/15 -> Bus Creator38/6  "Speed_Radial"
  CAN Unpack38/14 -> Terminator335/1
  CAN Unpack38/12 -> Bus Creator38/5  "Range"
  CAN Unpack38/11 -> Bus Creator38/4  "RCS"
  CAN Unpack38/16 -> Bus Creator38/7  "CAN ID"
  CAN Unpack38/17 -> Bus Creator38/8  "Timestamp"
  CAN Unpack38/9 -> Terminator333/1
  Bus Creator38/1 -> Bus Creator1/38  "Data_037"
  CAN Unpack39/4 -> Terminator337/1
  CAN Unpack39/2 -> Bus Creator39/2  "EL_Angle"
  CAN Unpack39/13 -> Terminator343/1
  CAN Unpack39/5 -> Terminator338/1
  CAN Unpack39/7 -> Terminator340/1
  CAN Unpack39/3 -> Terminator336/1
  CAN Unpack39/8 -> Terminator341/1
  CAN Unpack39/1 -> Bus Creator39/1  "AZ_Winkel"
  CAN Unpack39/6 -> Terminator339/1
  CAN Unpack39/10 -> Bus Creator39/3  "Mode_Signal"
  CAN Unpack39/15 -> Bus Creator39/6  "Speed_Radial"
  CAN Unpack39/14 -> Terminator344/1
  CAN Unpack39/12 -> Bus Creator39/5  "Range"
  CAN Unpack39/11 -> Bus Creator39/4  "RCS"
  CAN Unpack39/16 -> Bus Creator39/7  "CAN ID"
  CAN Unpack39/17 -> Bus Creator39/8  "Timestamp"
  CAN Unpack39/9 -> Terminator342/1
  Bus Creator39/1 -> Bus Creator1/39  "Data_038"
  CAN Unpack40/4 -> Terminator346/1
  CAN Unpack40/2 -> Bus Creator40/2  "EL_Angle"
  CAN Unpack40/13 -> Terminator352/1
  CAN Unpack40/5 -> Terminator347/1
  CAN Unpack40/7 -> Terminator349/1
  CAN Unpack40/3 -> Terminator345/1
  CAN Unpack40/8 -> Terminator350/1
  CAN Unpack40/1 -> Bus Creator40/1  "AZ_Winkel"
  CAN Unpack40/6 -> Terminator348/1
  CAN Unpack40/10 -> Bus Creator40/3  "Mode_Signal"
  CAN Unpack40/15 -> Bus Creator40/6  "Speed_Radial"
  CAN Unpack40/14 -> Terminator353/1
  CAN Unpack40/12 -> Bus Creator40/5  "Range"
  CAN Unpack40/11 -> Bus Creator40/4  "RCS"
  CAN Unpack40/16 -> Bus Creator40/7  "CAN ID"
  CAN Unpack40/17 -> Bus Creator40/8  "Timestamp"
  CAN Unpack40/9 -> Terminator351/1
  Bus Creator40/1 -> Bus Creator1/40  "Data_039"
  CAN Unpack41/4 -> Terminator355/1
  CAN Unpack41/2 -> Bus Creator41/2  "EL_Angle"
  CAN Unpack41/13 -> Terminator361/1
  CAN Unpack41/5 -> Terminator356/1
  CAN Unpack41/7 -> Terminator358/1
  CAN Unpack41/3 -> Terminator354/1
  CAN Unpack41/8 -> Terminator359/1
  CAN Unpack41/1 -> Bus Creator41/1  "AZ_Winkel"
  CAN Unpack41/6 -> Terminator357/1
  CAN Unpack41/10 -> Bus Creator41/3  "Mode_Signal"
  CAN Unpack41/15 -> Bus Creator41/6  "Speed_Radial"
  CAN Unpack41/14 -> Terminator362/1
  CAN Unpack41/12 -> Bus Creator41/5  "Range"
  CAN Unpack41/11 -> Bus Creator41/4  "RCS"
  CAN Unpack41/16 -> Bus Creator41/7  "CAN ID"
  CAN Unpack41/17 -> Bus Creator41/8  "Timestamp"
  CAN Unpack41/9 -> Terminator360/1
  Bus Creator41/1 -> Bus Creator1/41  "Data_040"
  CAN Unpack42/4 -> Terminator364/1
  CAN Unpack42/2 -> Bus Creator42/2  "EL_Angle"
  CAN Unpack42/13 -> Terminator370/1
  CAN Unpack42/5 -> Terminator365/1
  CAN Unpack42/7 -> Terminator367/1
  CAN Unpack42/3 -> Terminator363/1
  CAN Unpack42/8 -> Terminator368/1
  CAN Unpack42/1 -> Bus Creator42/1  "AZ_Winkel"
  CAN Unpack42/6 -> Terminator366/1
  CAN Unpack42/10 -> Bus Creator42/3  "Mode_Signal"
  CAN Unpack42/15 -> Bus Creator42/6  "Speed_Radial"
  CAN Unpack42/14 -> Terminator371/1
  CAN Unpack42/12 -> Bus Creator42/5  "Range"
  CAN Unpack42/11 -> Bus Creator42/4  "RCS"
  CAN Unpack42/16 -> Bus Creator42/7  "CAN ID"
  CAN Unpack42/17 -> Bus Creator42/8  "Timestamp"
  CAN Unpack42/9 -> Terminator369/1
  Bus Creator42/1 -> Bus Creator1/42  "Data_041"
  CAN Unpack43/4 -> Terminator373/1
  CAN Unpack43/2 -> Bus Creator43/2  "EL_Angle"
  CAN Unpack43/13 -> Terminator379/1
  CAN Unpack43/5 -> Terminator374/1
  CAN Unpack43/7 -> Terminator376/1
  CAN Unpack43/3 -> Terminator372/1
  CAN Unpack43/8 -> Terminator377/1
  CAN Unpack43/1 -> Bus Creator43/1  "AZ_Winkel"
  CAN Unpack43/6 -> Terminator375/1
  CAN Unpack43/10 -> Bus Creator43/3  "Mode_Signal"
  CAN Unpack43/15 -> Bus Creator43/6  "Speed_Radial"
  CAN Unpack43/14 -> Terminator380/1
  CAN Unpack43/12 -> Bus Creator43/5  "Range"
  CAN Unpack43/11 -> Bus Creator43/4  "RCS"
  CAN Unpack43/16 -> Bus Creator43/7  "CAN ID"
  CAN Unpack43/17 -> Bus Creator43/8  "Timestamp"
  CAN Unpack43/9 -> Terminator378/1
  Bus Creator43/1 -> Bus Creator1/43  "Data_042"
  CAN Unpack44/4 -> Terminator382/1
  CAN Unpack44/2 -> Bus Creator44/2  "EL_Angle"
  CAN Unpack44/13 -> Terminator388/1
  CAN Unpack44/5 -> Terminator383/1
  CAN Unpack44/7 -> Terminator385/1
  CAN Unpack44/3 -> Terminator381/1
  CAN Unpack44/8 -> Terminator386/1
  CAN Unpack44/1 -> Bus Creator44/1  "AZ_Winkel"
  CAN Unpack44/6 -> Terminator384/1
  CAN Unpack44/10 -> Bus Creator44/3  "Mode_Signal"
  CAN Unpack44/15 -> Bus Creator44/6  "Speed_Radial"
  CAN Unpack44/14 -> Terminator389/1
  CAN Unpack44/12 -> Bus Creator44/5  "Range"
  CAN Unpack44/11 -> Bus Creator44/4  "RCS"
  CAN Unpack44/16 -> Bus Creator44/7  "CAN ID"
  CAN Unpack44/17 -> Bus Creator44/8  "Timestamp"
  CAN Unpack44/9 -> Terminator387/1
  Bus Creator44/1 -> Bus Creator1/44  "Data_043"
  CAN Unpack45/4 -> Terminator391/1
  CAN Unpack45/2 -> Bus Creator45/2  "EL_Angle"
  CAN Unpack45/13 -> Terminator397/1
  CAN Unpack45/5 -> Terminator392/1
  CAN Unpack45/7 -> Terminator394/1
  CAN Unpack45/3 -> Terminator390/1
  CAN Unpack45/8 -> Terminator395/1
  CAN Unpack45/1 -> Bus Creator45/1  "AZ_Winkel"
  CAN Unpack45/6 -> Terminator393/1
  CAN Unpack45/10 -> Bus Creator45/3  "Mode_Signal"
  CAN Unpack45/15 -> Bus Creator45/6  "Speed_Radial"
  CAN Unpack45/14 -> Terminator398/1
  CAN Unpack45/12 -> Bus Creator45/5  "Range"
  CAN Unpack45/11 -> Bus Creator45/4  "RCS"
  CAN Unpack45/16 -> Bus Creator45/7  "CAN ID"
  CAN Unpack45/17 -> Bus Creator45/8  "Timestamp"
  CAN Unpack45/9 -> Terminator396/1
  Bus Creator45/1 -> Bus Creator1/45  "Data_044"
  CAN Unpack46/16 -> Bus Creator46/7  "CAN ID"
  CAN Unpack46/9 -> Terminator405/1
  CAN Unpack46/17 -> Bus Creator46/8  "Timestamp"
  CAN Unpack46/11 -> Bus Creator46/4  "RCS"
  CAN Unpack46/1 -> Bus Creator46/1  "AZ_Winkel"
  CAN Unpack46/14 -> Terminator407/1
  CAN Unpack46/6 -> Terminator402/1
  CAN Unpack46/15 -> Bus Creator46/6  "Speed_Radial"
  CAN Unpack46/10 -> Bus Creator46/3  "Mode_Signal"
  CAN Unpack46/2 -> Bus Creator46/2  "EL_Angle"
  CAN Unpack46/12 -> Bus Creator46/5  "Range"
  CAN Unpack46/7 -> Terminator403/1
  CAN Unpack46/8 -> Terminator404/1
  CAN Unpack46/5 -> Terminator401/1
  CAN Unpack46/4 -> Terminator400/1
  CAN Unpack46/13 -> Terminator406/1
  CAN Unpack46/3 -> Terminator399/1
  Bus Creator46/1 -> Bus Creator1/46  "Data_045"
  CAN Unpack47/3 -> Terminator408/1
  CAN Unpack47/2 -> Bus Creator47/2  "EL_Angle"
  CAN Unpack47/13 -> Terminator415/1
  CAN Unpack47/7 -> Terminator412/1
  CAN Unpack47/12 -> Bus Creator47/5  "Range"
  CAN Unpack47/10 -> Bus Creator47/3  "Mode_Signal"
  CAN Unpack47/4 -> Terminator409/1
  CAN Unpack47/5 -> Terminator410/1
  CAN Unpack47/8 -> Terminator413/1
  CAN Unpack47/11 -> Bus Creator47/4  "RCS"
  CAN Unpack47/14 -> Terminator416/1
  CAN Unpack47/15 -> Bus Creator47/6  "Speed_Radial"
  CAN Unpack47/9 -> Terminator414/1
  CAN Unpack47/6 -> Terminator411/1
  CAN Unpack47/16 -> Bus Creator47/7  "CAN ID"
  CAN Unpack47/17 -> Bus Creator47/8  "Timestamp"
  Bus Creator47/1 -> Bus Creator1/47  "Data_046"
  CAN Unpack47/1 -> Bus Creator47/1  "AZ_Winkel"
  CAN Unpack48/3 -> Terminator417/1
  CAN Unpack48/2 -> Bus Creator48/2  "EL_Angle"
  CAN Unpack48/13 -> Terminator424/1
  CAN Unpack48/7 -> Terminator421/1
  CAN Unpack48/12 -> Bus Creator48/5  "Range"
  CAN Unpack48/10 -> Bus Creator48/3  "Mode_Signal"
  CAN Unpack48/4 -> Terminator418/1
  CAN Unpack48/5 -> Terminator419/1
  CAN Unpack48/8 -> Terminator422/1
  CAN Unpack48/11 -> Bus Creator48/4  "RCS"
  CAN Unpack48/14 -> Terminator425/1
  CAN Unpack48/15 -> Bus Creator48/6  "Speed_Radial"
  CAN Unpack48/9 -> Terminator423/1
  CAN Unpack48/6 -> Terminator420/1
  CAN Unpack48/16 -> Bus Creator48/7  "CAN ID"
  CAN Unpack48/17 -> Bus Creator48/8  "Timestamp"
  Bus Creator48/1 -> Bus Creator1/48  "Data_047"
  CAN Unpack48/1 -> Bus Creator48/1  "AZ_Winkel"
  CAN Unpack49/3 -> Terminator426/1
  CAN Unpack49/2 -> Bus Creator49/2  "EL_Angle"
  CAN Unpack49/13 -> Terminator433/1
  CAN Unpack49/7 -> Terminator430/1
  CAN Unpack49/12 -> Bus Creator49/5  "Range"
  CAN Unpack49/10 -> Bus Creator49/3  "Mode_Signal"
  CAN Unpack49/4 -> Terminator427/1
  CAN Unpack49/5 -> Terminator428/1
  CAN Unpack49/8 -> Terminator431/1
  CAN Unpack49/11 -> Bus Creator49/4  "RCS"
  CAN Unpack49/14 -> Terminator434/1
  CAN Unpack49/15 -> Bus Creator49/6  "Speed_Radial"
  CAN Unpack49/9 -> Terminator432/1
  CAN Unpack49/6 -> Terminator429/1
  CAN Unpack49/16 -> Bus Creator49/7  "CAN ID"
  CAN Unpack49/17 -> Bus Creator49/8  "Timestamp"
  Bus Creator49/1 -> Bus Creator1/49  "Data_048"
  CAN Unpack49/1 -> Bus Creator49/1  "AZ_Winkel"
  CAN Unpack50/3 -> Terminator435/1
  CAN Unpack50/2 -> Bus Creator50/2  "EL_Angle"
  CAN Unpack50/13 -> Terminator442/1
  CAN Unpack50/7 -> Terminator439/1
  CAN Unpack50/12 -> Bus Creator50/5  "Range"
  CAN Unpack50/10 -> Bus Creator50/3  "Mode_Signal"
  CAN Unpack50/4 -> Terminator436/1
  CAN Unpack50/5 -> Terminator437/1
  CAN Unpack50/8 -> Terminator440/1
  CAN Unpack50/11 -> Bus Creator50/4  "RCS"
  CAN Unpack50/14 -> Terminator443/1
  CAN Unpack50/15 -> Bus Creator50/6  "Speed_Radial"
  CAN Unpack50/9 -> Terminator441/1
  CAN Unpack50/6 -> Terminator438/1
  CAN Unpack50/16 -> Bus Creator50/7  "CAN ID"
  CAN Unpack50/17 -> Bus Creator50/8  "Timestamp"
  Bus Creator50/1 -> Bus Creator1/50  "Data_049"
  CAN Unpack50/1 -> Bus Creator50/1  "AZ_Winkel"
  CAN Unpack51/3 -> Terminator444/1
  CAN Unpack51/2 -> Bus Creator51/2  "EL_Angle"
  CAN Unpack51/13 -> Terminator451/1
  CAN Unpack51/7 -> Terminator448/1
  CAN Unpack51/12 -> Bus Creator51/5  "Range"
  CAN Unpack51/10 -> Bus Creator51/3  "Mode_Signal"
  CAN Unpack51/4 -> Terminator445/1
  CAN Unpack51/5 -> Terminator446/1
  CAN Unpack51/8 -> Terminator449/1
  CAN Unpack51/11 -> Bus Creator51/4  "RCS"
  CAN Unpack51/14 -> Terminator452/1
  CAN Unpack51/15 -> Bus Creator51/6  "Speed_Radial"
  CAN Unpack51/9 -> Terminator450/1
  CAN Unpack51/6 -> Terminator447/1
  CAN Unpack51/16 -> Bus Creator51/7  "CAN ID"
  CAN Unpack51/17 -> Bus Creator51/8  "Timestamp"
  Bus Creator51/1 -> Bus Creator1/51  "Data_050"
  CAN Unpack51/1 -> Bus Creator51/1  "AZ_Winkel"
  CAN Unpack52/3 -> Terminator453/1
  CAN Unpack52/2 -> Bus Creator52/2  "EL_Angle"
  CAN Unpack52/13 -> Terminator460/1
  CAN Unpack52/7 -> Terminator457/1
  CAN Unpack52/12 -> Bus Creator52/5  "Range"
  CAN Unpack52/10 -> Bus Creator52/3  "Mode_Signal"
  CAN Unpack52/4 -> Terminator454/1
  CAN Unpack52/5 -> Terminator455/1
  CAN Unpack52/8 -> Terminator458/1
  CAN Unpack52/11 -> Bus Creator52/4  "RCS"
  CAN Unpack52/14 -> Terminator461/1
  CAN Unpack52/15 -> Bus Creator52/6  "Speed_Radial"
  CAN Unpack52/9 -> Terminator459/1
  CAN Unpack52/6 -> Terminator456/1
  CAN Unpack52/16 -> Bus Creator52/7  "CAN ID"
  CAN Unpack52/17 -> Bus Creator52/8  "Timestamp"
  Bus Creator52/1 -> Bus Creator1/52  "Data_051"
  CAN Unpack52/1 -> Bus Creator52/1  "AZ_Winkel"
  CAN Unpack53/3 -> Terminator462/1
  CAN Unpack53/2 -> Bus Creator53/2  "EL_Angle"
  CAN Unpack53/13 -> Terminator469/1
  CAN Unpack53/7 -> Terminator466/1
  CAN Unpack53/12 -> Bus Creator53/5  "Range"
  CAN Unpack53/10 -> Bus Creator53/3  "Mode_Signal"
  CAN Unpack53/4 -> Terminator463/1
  CAN Unpack53/5 -> Terminator464/1
  CAN Unpack53/8 -> Terminator467/1
  CAN Unpack53/11 -> Bus Creator53/4  "RCS"
  CAN Unpack53/14 -> Terminator470/1
  CAN Unpack53/15 -> Bus Creator53/6  "Speed_Radial"
  CAN Unpack53/9 -> Terminator468/1
  CAN Unpack53/6 -> Terminator465/1
  CAN Unpack53/16 -> Bus Creator53/7  "CAN ID"
  CAN Unpack53/17 -> Bus Creator53/8  "Timestamp"
  Bus Creator53/1 -> Bus Creator1/53  "Data_052"
  CAN Unpack53/1 -> Bus Creator53/1  "AZ_Winkel"
  CAN Unpack54/3 -> Terminator471/1
  CAN Unpack54/2 -> Bus Creator54/2  "EL_Angle"
  CAN Unpack54/13 -> Terminator478/1
  CAN Unpack54/7 -> Terminator475/1
  CAN Unpack54/12 -> Bus Creator54/5  "Range"
  CAN Unpack54/10 -> Bus Creator54/3  "Mode_Signal"
  CAN Unpack54/4 -> Terminator472/1
  CAN Unpack54/5 -> Terminator473/1
  CAN Unpack54/8 -> Terminator476/1
  CAN Unpack54/11 -> Bus Creator54/4  "RCS"
  CAN Unpack54/14 -> Terminator479/1
  CAN Unpack54/15 -> Bus Creator54/6  "Speed_Radial"
  CAN Unpack54/9 -> Terminator477/1
  CAN Unpack54/6 -> Terminator474/1
  CAN Unpack54/16 -> Bus Creator54/7  "CAN ID"
  CAN Unpack54/17 -> Bus Creator54/8  "Timestamp"
  Bus Creator54/1 -> Bus Creator1/54  "Data_053"
  CAN Unpack54/1 -> Bus Creator54/1  "AZ_Winkel"
  CAN Unpack55/3 -> Terminator480/1
  CAN Unpack55/2 -> Bus Creator55/2  "EL_Angle"
  CAN Unpack55/13 -> Terminator487/1
  CAN Unpack55/7 -> Terminator484/1
  CAN Unpack55/12 -> Bus Creator55/5  "Range"
  CAN Unpack55/10 -> Bus Creator55/3  "Mode_Signal"
  CAN Unpack55/4 -> Terminator481/1
  CAN Unpack55/5 -> Terminator482/1
  CAN Unpack55/8 -> Terminator485/1
  CAN Unpack55/11 -> Bus Creator55/4  "RCS"
  CAN Unpack55/14 -> Terminator488/1
  CAN Unpack55/15 -> Bus Creator55/6  "Speed_Radial"
  CAN Unpack55/9 -> Terminator486/1
  CAN Unpack55/6 -> Terminator483/1
  CAN Unpack55/16 -> Bus Creator55/7  "CAN ID"
  CAN Unpack55/17 -> Bus Creator55/8  "Timestamp"
  Bus Creator55/1 -> Bus Creator1/55  "Data_054"
  CAN Unpack55/1 -> Bus Creator55/1  "AZ_Winkel"
  CAN Unpack56/3 -> Terminator489/1
  CAN Unpack56/2 -> Bus Creator56/2  "EL_Angle"
  CAN Unpack56/13 -> Terminator496/1
  CAN Unpack56/7 -> Terminator493/1
  CAN Unpack56/12 -> Bus Creator56/5  "Range"
  CAN Unpack56/10 -> Bus Creator56/3  "Mode_Signal"
  CAN Unpack56/4 -> Terminator490/1
  CAN Unpack56/5 -> Terminator491/1
  CAN Unpack56/8 -> Terminator494/1
  CAN Unpack56/11 -> Bus Creator56/4  "RCS"
  CAN Unpack56/14 -> Terminator497/1
  CAN Unpack56/15 -> Bus Creator56/6  "Speed_Radial"
  CAN Unpack56/9 -> Terminator495/1
  CAN Unpack56/6 -> Terminator492/1
  CAN Unpack56/16 -> Bus Creator56/7  "CAN ID"
  CAN Unpack56/17 -> Bus Creator56/8  "Timestamp"
  Bus Creator56/1 -> Bus Creator1/56  "Data_055"
  CAN Unpack56/1 -> Bus Creator56/1  "AZ_Winkel"
  CAN Unpack57/3 -> Terminator498/1
  CAN Unpack57/2 -> Bus Creator57/2  "EL_Angle"
  CAN Unpack57/13 -> Terminator505/1
  CAN Unpack57/7 -> Terminator502/1
  CAN Unpack57/12 -> Bus Creator57/5  "Range"
  CAN Unpack57/10 -> Bus Creator57/3  "Mode_Signal"
  CAN Unpack57/4 -> Terminator499/1
  CAN Unpack57/5 -> Terminator500/1
  CAN Unpack57/8 -> Terminator503/1
  CAN Unpack57/11 -> Bus Creator57/4  "RCS"
  CAN Unpack57/14 -> Terminator506/1
  CAN Unpack57/15 -> Bus Creator57/6  "Speed_Radial"
  CAN Unpack57/9 -> Terminator504/1
  CAN Unpack57/6 -> Terminator501/1
  CAN Unpack57/16 -> Bus Creator57/7  "CAN ID"
  CAN Unpack57/17 -> Bus Creator57/8  "Timestamp"
  Bus Creator57/1 -> Bus Creator1/57  "Data_056"
  CAN Unpack57/1 -> Bus Creator57/1  "AZ_Winkel"
  CAN Unpack58/3 -> Terminator507/1
  CAN Unpack58/2 -> Bus Creator58/2  "EL_Angle"
  CAN Unpack58/13 -> Terminator514/1
  CAN Unpack58/7 -> Terminator511/1
  CAN Unpack58/12 -> Bus Creator58/5  "Range"
  CAN Unpack58/10 -> Bus Creator58/3  "Mode_Signal"
  CAN Unpack58/4 -> Terminator508/1
  CAN Unpack58/5 -> Terminator509/1
  CAN Unpack58/8 -> Terminator512/1
  CAN Unpack58/11 -> Bus Creator58/4  "RCS"
  CAN Unpack58/14 -> Terminator515/1
  CAN Unpack58/15 -> Bus Creator58/6  "Speed_Radial"
  CAN Unpack58/9 -> Terminator513/1
  CAN Unpack58/6 -> Terminator510/1
  CAN Unpack58/16 -> Bus Creator58/7  "CAN ID"
  CAN Unpack58/17 -> Bus Creator58/8  "Timestamp"
  Bus Creator58/1 -> Bus Creator1/58  "Data_057"
  CAN Unpack58/1 -> Bus Creator58/1  "AZ_Winkel"
  CAN Unpack59/3 -> Terminator516/1
  CAN Unpack59/2 -> Bus Creator59/2  "EL_Angle"
  CAN Unpack59/13 -> Terminator523/1
  CAN Unpack59/7 -> Terminator520/1
  CAN Unpack59/12 -> Bus Creator59/5  "Range"
  CAN Unpack59/10 -> Bus Creator59/3  "Mode_Signal"
  CAN Unpack59/4 -> Terminator517/1
  CAN Unpack59/5 -> Terminator518/1
  CAN Unpack59/8 -> Terminator521/1
  CAN Unpack59/11 -> Bus Creator59/4  "RCS"
  CAN Unpack59/14 -> Terminator524/1
  CAN Unpack59/15 -> Bus Creator59/6  "Speed_Radial"
  CAN Unpack59/9 -> Terminator522/1
  CAN Unpack59/6 -> Terminator519/1
  CAN Unpack59/16 -> Bus Creator59/7  "CAN ID"
  CAN Unpack59/17 -> Bus Creator59/8  "Timestamp"
  Bus Creator59/1 -> Bus Creator1/59  "Data_058"
  CAN Unpack59/1 -> Bus Creator59/1  "AZ_Winkel"
  CAN Unpack60/3 -> Terminator525/1
  CAN Unpack60/2 -> Bus Creator60/2  "EL_Angle"
  CAN Unpack60/13 -> Terminator532/1
  CAN Unpack60/7 -> Terminator529/1
  CAN Unpack60/12 -> Bus Creator60/5  "Range"
  CAN Unpack60/10 -> Bus Creator60/3  "Mode_Signal"
  CAN Unpack60/4 -> Terminator526/1
  CAN Unpack60/5 -> Terminator527/1
